simulink library "outp"  (R2021b)
settings: Solver=VariableStepAuto  StartTime=0.0  StopTime=10.0  RelTol=1e-3
undefined symbols (not defined in the file): ENUM_PMMMODE_CHARGE, ENUM_PMMMODE_IDLE, ENUM_PMMMODE_INITIALIZE, ENUM_PMMMODE_POWERDOWN, ENUM_PMMMODE_SLEEP, Left, outp, slcm, TRUE
libraries: FVT_lib x1177, hcu_lib x4, simulink x1
(part 2 of 11)

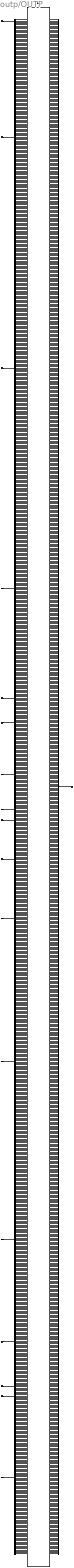
== system outp/OUTP ==
  BACC_outputs : Inport  OutDataTypeStr=Bus: BACC_outputs
  BAPM_outputs : Inport  Port=2  OutDataTypeStr=Bus: BAPM_outputs
  BBCM_outputs : Inport  Port=3  OutDataTypeStr=Bus: BBCM_outputs
  BDDM_outputs : Inport  Port=4  OutDataTypeStr=Bus: BDDM_outputs
  BDHP_outputs : Inport  Port=5  OutDataTypeStr=Bus: BDHP_outputs
  BDID_outputs : Inport  Port=6  OutDataTypeStr=Bus: BDID_outputs
  BDKC_outputs : Inport  Port=7  OutDataTypeStr=Bus: BDKC_outputs
  BDSC_outputs : Inport  Port=8  OutDataTypeStr=Bus: BDSC_outputs
  BNMM_outputs : Inport  Port=9  OutDataTypeStr=Bus: BNMM_outputs
  BPMM_outputs : Inport  Port=10  OutDataTypeStr=Bus: BPMM_outputs
  BSYS_outputs : Inport  Port=11  OutDataTypeStr=Bus: BSYS_outputs
  BTHC_outputs : Inport  Port=12  OutDataTypeStr=Bus: BTHC_outputs
  BTPM_outputs : Inport  Port=13  OutDataTypeStr=Bus: BTPM_outputs
  BTQD_outputs : Inport  Port=14  OutDataTypeStr=Bus: BTQD_outputs
  BTQR_outputs : Inport  Port=15  OutDataTypeStr=Bus: BTQR_outputs
  BV2L_outputs : Inport  Port=16  OutDataTypeStr=Bus: BV2L_outputs
  BVMC_outputs : Inport  Port=17  OutDataTypeStr=Bus: BVMC_outputs
  trig_OUTP : TriggerPort  TriggerType=function-call  VariantControl=(inherit)
  bus_creator : BusCreator  Inputs=1177  OutDataTypeStr=Bus: BOUTP_outputs  NonVirtualBus=on
  bus_selector1 : BusSelector  OutputSignals=VACC_HVTHCMSysAvail_enum,VACC_LVBattVoltSta_enum,VACC_VehHVPwrAvail4THCM_W
  bus_selector10 : BusSelector  OutputSignals=VPMM_PowerUpState_enum,VPMM_PowerDownState_enum,VPMM_PowerUpFault_enum,VPMM_PowerDownFault_enum,VPMM_ActiveDischargeReq_flg,VPMM_DCDCEnaReq_flg,VPMM_DCDCVoltSetpoint_V,VPMM_HVBatCnctReq_flg,VPMM_HVSysReadyToCharge_enum,VPMM_PowerSta_enum,VPMM_LVPwrSta_flg,VPMM_HVPwrSta_flg,VPMM_SysPowerMode_enum,VPMM_FrMCUEnaReq_flg,VPMM_RrMCUEnaReq_flg,VPMM_DrivetrainSelect_enum,VPMM_DrSeatSta_enum,VPMM_PwrStaSelect_enum,VPMM_PwrStaConstraint_enum,VPMM_TCountSta_enum,VPMM_PwrUpReq_enum,VPMM_PwrDownReq_enum,VPMM_LowSOCWarn_enum,VPMM_ReVehThdChkSta_enum,VPMM_EvccAplusPwrUpReq_flg,VPMM_PwrStaONTOPopReq_flg,VPMM_IVIPwrStaONTOPopT_s,VPMM_LVChrgHoldTtimer_s,VPMM_LVBattChrgTimeCnt_s,VPMM_SilentChkAllowSleep_flg,VPMM_TimerAllowSleep_flg,VPMM_FDADC12VDetAvg_mV,VPMM_PMMAllowECUSleep_flg,VPMM_LVSilentChrgSta_enum,VPMM_LVSilentChrgReq_flg,VPMM_LVSilentChrgLv_enum,VPMM_CtrlFrPwrStbA1P_flg,VPMM_CtrlFrRC1_flg,VPMM_CtrlFrBMSCCUCIR_flg,VPMM_CtrlFrEDUINVERTER_flg,VPMM_HWResetSta_enum,VPMM_CtrlDrPwrStbA2_flg,VPMM_PwrStaTOSta_enum,VPMM_Sched_ChgTOSta_enum,VPMM_PwrReq_OTA_enum,VPMM_OTAPwrReqOFFChkSta_enum,VPMM_OTAPwrReqStdChkSta_enum,VPMM_PwrReqRAPSAvail_flg
  bus_selector11 : BusSelector  OutputSignals=VSYS_HWVer1_cnt,VSYS_HWVer2_cnt,VSYS_HWVer3_cnt,VSYS_CarModel1_cnt,VSYS_CarModel2_cnt,VSYS_CarModel3_cnt,VSYS_ECU1_cnt,VSYS_ECU2_cnt,VSYS_Major1_cnt,VSYS_Major2_cnt,VSYS_Minor1_cnt,VSYS_Minor2_cnt,VSYS_Patch1_cnt,VSYS_Patch2_cnt,VSYS_Country1_cnt,VSYS_Country2_cnt,VSYS_Variation_cnt,VSYS_Dash1_cnt,VSYS_Change1_cnt,VSYS_Change2_cnt,VSYS_Dash2_cnt,VSYS_SHA1_cnt,VSYS_SHA2_cnt,VSYS_SHA3_cnt,VSYS_SHA4_cnt,VSYS_SHA5_cnt,VSYS_SHA6_cnt,VSYS_SHA7_cnt,VSYS_SHA8_cnt,VSYS_NvWriteReqRisingEdge_flg,VSYS_FdcSlpReqRisingEdge_flg,VSYS_FdcSlpTime_sec,VSYS_PmicBootReason_enum,VSYS_WisrBootReason_raw32,VSYS_AcoreRebootCmdACK_flg,VSYS_CurrentNmState_enum,VSYS_ECUGen1_cnt,VSYS_ECUGen2_cnt,VSYS_PmicBootPath_raw32,VSYS_DrivingMode_cnt,VSYS_ModelYear_cnt,VSYS_Var4_cnt,VSYS_Var5_cnt
  bus_selector12 : BusSelector  OutputSignals=VTHC_FDCompCmd_rpm,VTHC_FDSOV1Cmd_flg,VTHC_FDSOV2Cmd_flg,VTHC_FDSOV3Cmd_flg,VTHC_FDEXV1Cmd_step,VTHC_FDEXV2Cmd_step,VTHC_FDSOTXVCmd_flg,VTHC_FDFWVCmd_flg,VTHC_FDTWVCmd_pct,VTHC_FDFrWPTCHeatPwrCmd_W,VTHC_CoolgFanActDuty_pct,VTHC_FDAGSCmd_enum,VTHC_FDEWP1Cmd_enum,VTHC_FDEWP2Cmd_enum,VTHC_FDEWP3Cmd_enum,VTHC_FDFrLeAPTCHeatPwrCmd_W,VTHC_FDFrRiAPTCHeatPwrCmd_W,VTHC_FDRrAPTCHeatPwrCmd_W,VTHC_FDBlowerCmd_pct,VTHC_BatteryMode_enum,VTHC_EDriveMode_enum,VTHC_CabinMode_enum,VTHC_CCUACLampSts_flg,VTHC_CCUAutoLampSts_flg,VTHC_CCUACMaxLampSts_flg,VTHC_CCUSyncLampSts_flg,VTHC_sigAirIntenZon1St_enum,VTHC_sigWindDirZon1St_enum,VTHC_sigRecircSt_flg,VTHC_sigSetTempZon1St_C,VTHC_sigSetTempZon2St_C,VTHC_sigClntTHvBattOut_C,VTHC_sigCbnSolarLeft_W,VTHC_sigClntTHvBattIn_C,VTHC_sigCbnSolarRight_W,VTHC_sigAmbAirT_C,VTHC_sigCbnAirT_C,VTHC_ACSubMode_enum,VTHC_FDRecyAutoCmd_enum,VTHC_ACModeMem_enum,VTHC_Face_flg,VTHC_Foot_flg,VTHC_Frost_flg,VTHC_FaceM_flg,VTHC_FootM_flg,VTHC_CCUSyncSts_flg,VTHC_ACForceOFF_flg,VTHC_RecAutoFlg_flg,VTHC_AirIntenZone1M_enum,VTHC_fdefog_flg,VTHC_sigSetTempZon2StM_C,VTHC_sigDfrstSt_flg,VTHC_FDCTHCAirIntZ3Sta_enum,VTHC_FDCTHCLEVentModeSta_enum,VTHC_FDCTHCREVentModeSta_enum,VTHC_FDCTHCLEVentZSta_enum,VTHC_FDCTHCCLEVentZSta_enum,VTHC_FDCTHCREVentZSta_enum,VTHC_FDCTHCCREVentZSta_enum,VTHC_FDCTHCLEVentYSta_enum,VTHC_FDCTHCLVentENSta_flg,VTHC_FDCTHCCLEVentYSta_enum,VTHC_FDCTHCCLVentENSta_flg,VTHC_FDCTHCREVentYSta_enum,VTHC_FDCTHCRVentENSta_flg,VTHC_FDCTHCCREVentYSta_enum,VTHC_FDCTHCCRVentENSta_flg,VTHC_FDCTHCMAPTCForceOFFSta_flg,VTHC_FDCFGSAirIntSta_enum,VTHC_FDCFGSChSta_enum,VTHC_FDCFGSAirIntCmd_enum,VTHC_FDCFGSFuncSta_enum,VTHC_FDCFGSChCmd_enum,VTHC_FDCFGSIONSWSta_flg,VTHC_FDCFGSIONCmd_flg,VTHC_FDCTHCMPreWPTCHeatSta_enum,VTHC_EWPBUflag1_flg,VTHC_EWPBUflag2_flg,VTHC_EWPBUflag3_flg,VTHC_FaceMSet_enum,VTHC_FootMSet_enum,VTHC_fdefogSet_enum,VTHC_CCUSyncStsSet_enum,VTHC_sigRecircStSet_enum,VTHC_RecyAutoSet_enum,VTHC_AirIntenZone1MSet1_enum,VTHC_AirIntenZone1MSet2_enum,VTHC_AirIntenZone1MSet3_enum,VTHC_AirIntenZone1MSet4_enum,VTHC_AirIntenZone1MSet5_enum,VTHC_AirIntenZone1MSet7_enum,VTHC_AirIntenZone3MSet1_enum,VTHC_AirIntenZone3MSet2_enum,VTHC_AirIntenZone3MSet3_enum,VTHC_AirIntenZone3MSet4_enum,VTHC_AirIntenZone3MSet5_enum,VTHC_AirIntenZone3MSet7_enum,VTHC_IONSWStaSet_enum,VTHC_FDCFGSChStaSet123_enum,VTHC_FDCFGSChStaSet457_enum,VTHC_FDCFGSAirIntStaSet123_enum,VTHC_FDCFGSAirIntStaSet457_enum,VTHC_LVentENSet_enum,VTHC_CLVentENSet_enum,VTHC_RVentENSet_enum,VTHC_CRVentENSet_enum,VTHC_LEVentModeStaSet123_enum,VTHC_LEVentModeStaSet457_enum,VTHC_REVentModeStaSet123_enum,VTHC_REVentModeStaSet457_enum,VTHC_FDCTHCLEVentZStaSet1_enum,VTHC_FDCTHCLEVentZStaSet2_enum,VTHC_FDCTHCLEVentZStaSet3_enum,VTHC_FDCTHCLEVentZStaSet4_enum,VTHC_FDCTHCLEVentZStaSet5_enum,VTHC_FDCTHCLEVentZStaSet7_enum,VTHC_FDCTHCCLEVentZStaSet1_enum,VTHC_FDCTHCCLEVentZStaSet2_enum,VTHC_FDCTHCCLEVentZStaSet3_enum,VTHC_FDCTHCCLEVentZStaSet4_enum,VTHC_FDCTHCCLEVentZStaSet5_enum,VTHC_FDCTHCCLEVentZStaSet7_enum,VTHC_FDCTHCREVentZStaSet1_enum,VTHC_FDCTHCREVentZStaSet2_enum,VTHC_FDCTHCREVentZStaSet3_enum,VTHC_FDCTHCREVentZStaSet4_enum,VTHC_FDCTHCREVentZStaSet5_enum,VTHC_FDCTHCREVentZStaSet7_enum,VTHC_FDCTHCCREVentZStaSet1_enum,VTHC_FDCTHCCREVentZStaSet2_enum,VTHC_FDCTHCCREVentZStaSet3_enum,VTHC_FDCTHCCREVentZStaSet4_enum,VTHC_FDCTHCCREVentZStaSet5_enum,VTHC_FDCTHCCREVentZStaSet7_enum,VTHC_FDCTHCLEVentYStaSet1_enum,VTHC_FDCTHCLEVentYStaSet2_enum,VTHC_FDCTHCLEVentYStaSet3_enum,VTHC_FDCTHCLEVentYStaSet4_enum,VTHC_FDCTHCLEVentYStaSet5_enum,VTHC_FDCTHCLEVentYStaSet7_enum,VTHC_FDCTHCCLEVentYStaSet1_enum,VTHC_FDCTHCCLEVentYStaSet2_enum,VTHC_FDCTHCCLEVentYStaSet3_enum,VTHC_FDCTHCCLEVentYStaSet4_enum,VTHC_FDCTHCCLEVentYStaSet5_enum,VTHC_FDCTHCCLEVentYStaSet7_enum,VTHC_FDCTHCREVentYStaSet1_enum,VTHC_FDCTHCREVentYStaSet2_enum,VTHC_FDCTHCREVentYStaSet3_enum,VTHC_FDCTHCREVentYStaSet4_enum,VTHC_FDCTHCREVentYStaSet5_enum,VTHC_FDCTHCREVentYStaSet7_enum,VTHC_FDCTHCCREVentYStaSet1_enum,VTHC_FDCTHCCREVentYStaSet2_enum,VTHC_FDCTHCCREVentYStaSet3_enum,VTHC_FDCTHCCREVentYStaSet4_enum,VTHC_FDCTHCCREVentYStaSet5_enum,VTHC_FDCTHCCREVentYStaSet7_enum,VTHC_SettempZon1Set1_enum,VTHC_SettempZon1Set2_enum,VTHC_SettempZon1Set3_enum,VTHC_SettempZon1Set4_enum,VTHC_SettempZon1Set5_enum,VTHC_SettempZon1Set7_enum,VTHC_ACModeSet123_enum,VTHC_ACModeSet457_enum,VTHC_FACESet_enum,VTHC_FOOTSet_enum,VTHC_FrostSet_enum,VTHC_LVentEN_flg,VTHC_CLVentEN_flg,VTHC_RVentEN_flg,VTHC_CRVentEN_flg,VTHC_FDCFGSLearnCmd_enum,VTHC_FDCFGSFuncSta_flg,VTHC_THSysErrlampReq_flg
  bus_selector13 : BusSelector  OutputSignals=VTPM_LFBatWarn_flg,VTPM_RFBatWarn_flg,VTPM_LRBatWarn_flg,VTPM_RRBatWarn_flg,VTPM_LFWheelPress_raw8,VTPM_RFWheelPress_raw8,VTPM_LRWheelPress_raw8,VTPM_RRWheelPress_raw8,VTPM_LFWheelTemp_C,VTPM_RFWheelTemp_C,VTPM_LRWheelTemp_C,VTPM_RRWheelTemp_C,VTPM_LFSensorFail_flg,VTPM_RFSensorFail_flg,VTPM_LRSensorFail_flg,VTPM_RRSensorFail_flg,VTPM_LFWheelDebug_flg,VTPM_LRWheelDebug_flg,VTPM_RFWheelDebug_flg,VTPM_RRWheelDebug_flg,VTPM_TPMSResButtAllow_flg,VTPM_TPMSCaliButtAllow_flg,VTPM_LFPressIndi_enum,VTPM_RFPressIndi_enum,VTPM_LRPressIndi_enum,VTPM_RRPressIndi_enum,VTPM_TPMSWarnIndi_enum,VTPM_LFWheelTmpIndi_flg,VTPM_RFWheelTmpIndi_flg,VTPM_LRWheelTmpIndi_flg,VTPM_RRWheelTmpIndi_flg,VTPM_LFWheelPSW_raw8,VTPM_LRWheelPSW_raw8,VTPM_RFWheelPSW_raw8,VTPM_RRWheelPSW_raw8,VTPM_CWheelTips_enum,VTPM_AutoLTips_enum,VTPM_LFSensorMode_flg,VTPM_RFSensorMode_flg,VTPM_LRSensorMode_flg,VTPM_RRSensorMode_flg,VTPM_S1ID_raw32,VTPM_S2ID_raw32,VTPM_S3ID_raw32,VTPM_S4ID_raw32,VTPM_S1L_enum,VTPM_S2L_enum,VTPM_S3L_enum,VTPM_S4L_enum,VTPM_ALFin_flg,VTPM_LFP20_raw8,VTPM_RFP20_raw8,VTPM_LRP20_raw8,VTPM_RRP20_raw8,VTPM_FAT_flg,VTPM_IDin_raw32,VTPM_S1WheelDebugALTU_pct,VTPM_S2WheelDebugALTU_pct,VTPM_S3WheelDebugALTU_pct,VTPM_S4WheelDebugALTU_pct,VTPM_ID1messageALTU_raw8,VTPM_ID2messageALTU_raw8,VTPM_ID3messageALTU_raw8,VTPM_ID4messageALTU_raw8,VTPM_Chkfin_flg,VTPM_SetIDLoc_flg,VTPM_TPMSStorge_flg,VTPM_ChkStorge_flg,VTPM_TPMSResButt_flg,VTPM_LFPindi_enum,VTPM_RFPind_enum,VTPM_LRPindi_enum,VTPM_RRPindi_enum,VTPM_WriteChkLFID_raw,VTPM_WriteChkRFID_raw,VTPM_WriteChkLRID_raw,VTPM_WriteChkRRID_raw,VTPM_WriteChkfinLFID_raw,VTPM_WriteChkfinRFID_raw,VTPM_WriteChkfinLRID_raw,VTPM_WriteChkfinRRID_raw,VTPM_Flashchkdatavalid_enum,VTPM_Flashdatavalid_enum,VTPM_unlearnSfali_flg,VTPM_unlearnSfailvalid_enum,VTPM_Prepresstempvalid_enum,VTPM_FlashS1ID_raw,VTPM_FlashS2ID_raw,VTPM_FlashS3ID_raw,VTPM_FlashS4ID_raw,VTPM_FlashIDvalid_enum,VTPM_WritingCnt_enum,VTPM_TPMSTLCmd_flg,VTPM_LProgress_enum,VTPM_TPMSSensorIDRegStart_flg,VTPM_ModelVersion_raw,VTPM_ModelVersionChksum_raw
  bus_selector14 : BusSelector  OutputSignals=VTQD_ParkRequest_flg,VTQD_TqSourceFr_enum,VTQD_TqSourceRr_enum,VTQD_FrEDUAvailBrkRgnTq_Nm,VTQD_RrEDUAvailBrkRgnTq_Nm,VTQD_EVDriveMode_enum,VTQD_ShiftGearPosn_enum,VTQD_PButtonSta_enum,VTQD_FrActvDmpDisabReq_flg,VTQD_RrActvDmpDisabReq_flg,VTQD_FrRgnDecrSta_flg,VTQD_RrRgnDecrSta_flg,VTQD_DriverWhlTqDemFr_Nm,VTQD_DriverWhlTqDemRr_Nm,VTQD_FrEDUActTq_Nm,VTQD_RrEDUActTq_Nm,VTQD_FrEDURolRgnTq_Nm,VTQD_RrEDURolRgnTq_Nm,VTQD_FrEDUSpd_rpm,VTQD_RrEDUSpd_rpm,VTQD_FrEDUSpdValid_flg,VTQD_FrEDUAvailBrkRgnTqV_flg,VTQD_RrEDUSpdValid_flg,VTQD_RrEDUAvailBrkRgnTqV_flg,VTQD_RgnAbnorSta_flg,VTQD_PTCSPermSta_flg,VTQD_FrRgnPermSta_flg,VTQD_RrRgnPermSta_flg,VTQD_FrIdcMin_A,VTQD_FrIdcMax_A,VTQD_FrUdcMin_V,VTQD_FrUdcMax_V,VTQD_RrIdcMin_A,VTQD_RrIdcMax_A,VTQD_RrUdcMin_V,VTQD_RrUdcMax_V,VTQD_ReBrakeLPReq_flg,VTQD_BOSEnable_flg,VTQD_CreepON_flg,VTQD_RDCActive_enum,VTQD_EquivAccPedalSWSta_flg,VTQD_DriveProtEn_flg,VTQD_ActParkRequest_flg,VTQD_RegenTqLimitEn_flg,VTQD_IVIPwrLockSta_enum,VTQD_OPDHoldLamp_flg,VTQD_SaveRegenMode_enum,VTQD_FDCVCURegenMode_enum,VTQD_SpdCtrlMode_enum,VTQD_SpdCtrlSta_flg,VTQD_SetSpd_kph,VTQD_VehActSpd_kph,VTQD_RegenLimIndSta_flg,VTQD_SetSpdLimWarn_flg,VTQD_MaxWhlSlideRate_pct,VTQD_TrailerDisOPDSta_flg,VTQD_ForceP_flg,VTQD_SlideRegenLimTq_Nm,VTQD_SimSoundCmd_pct,VTQD_SimSouWaveReq_pct
  bus_selector15 : BusSelector  OutputSignals=VTQR_FrTMTqReq_Nm,VTQR_RrTMTqReq_Nm,VTQR_FrFirstOrderInpTs_c,VTQR_RrFirstOrderInpTs_c,VTQR_FrRateLimitInc_Nm,VTQR_FrRateLimitDec_Nm,VTQR_RrRateLimitInc_Nm,VTQR_RrRateLimitDec_Nm
  bus_selector16 : BusSelector  OutputSignals=VV2L_ReqOBCV2LEna_enum,VV2L_ReqV2LIVIPopup_enum,VV2L_ReqV2LIVIDisChrg_enum,VV2L_ReqOBCExtrV2LEna_enum,VV2L_ReqOBCIntrV2LEna_enum,VV2L_HVPO120VGrpALDSt_enum,VV2L_HVPO120VGrpBLDSt_enum
  bus_selector17 : BusSelector  OutputSignals=VVMC_FeatSetSpdFinal_raw32,VVMC_VehicleSpeed_mph,VVMC_VehicleSpeed_kph,VVMC_MeterIndSpeed_raw32,VVMC_VMCAEBCtrlAvail_flg,VVMC_VMCACCCtrlAvail_flg,VVMC_VMCCCCtrlAvail_flg,VVMC_VMCMSACtrlAvail_flg,VVMC_FeatArbitrSta_enum,VVMC_FeatReqSpd_kph,VVMC_JerkPCT_pct,VVMC_LimitPCT_pct,VVMC_FrontRearSlipRatioCtrl_flg,VVMC_RearWhlSlipRatioCtrl_flg,VVMC_SingleWhlSlipRatioCtrl_flg,VVMC_LatAccCtrl_flg,VVMC_SafetyCtrl_flg,VVMC_SPD2ACCAct_flg,VVMC_AccCalcuPID_mps2,VVMC_ISOAccLimit_mps2,VVMC_ISODecLimit_mps2,VVMC_ISOJerkLimit_mps3,VVMC_ACCRequiredAccel_mps2,VVMC_DISCReqAcc_mps2,VVMC_FeatArbitrFinal_enum,VVMC_ActACCRequiredAccel_mps2,VVMC_LateralCtrl_flg,VVMC_ADASLKASta_enum,VVMC_LKAStrToqReq_Nm,VVMC_LKATOIFault_flg,VVMC_LKATOIAct_enum,VVMC_ADASAEBReq_enum,VVMC_ADASFaultSta_flg,VVMC_AEBVehHoldReq_flg,VVMC_ACCVehHoldReq_flg,VVMC_ADASDBSReq_enum,VVMC_ADASACCSta_enum,VVMC_ACCObjDist_m,VVMC_ACCObjRelSpd_mps,VVMC_TimeGapLevel_enum,VVMC_ACCJerkUpperLimit_mps3,VVMC_ACCComfortBandUpper_mps2,VVMC_ACCJerkLowerLimit_mps3,VVMC_ACCComfortBandLower_mps2,VVMC_ADASVehSpdLim_raw32,VVMC_ADASShftPosnReqA_flg,VVMC_ADASShftPosnReq_enum,VVMC_ADASForceIdle_flg,VVMC_HazardWarningReq_flg,VVMC_RightTurnLightReq_flg,VVMC_LeftTurnLightReq_flg,VVMC_ADASFCWSta_enum,VVMC_ADASLDWSta_enum,VVMC_ADASFltWrnReq_flg,VVMC_ACCObjDstLvl_enum,VVMC_ForceLowBeam_enum,VVMC_ACCTakeoverReq_flg,VVMC_ADASWarningMsg_enum,VVMC_ADASCAMSpdLim_enum,VVMC_TargetType_enum,VVMC_ADASSLIFSpdLim_enum,VVMC_LKAHODDisplayWarning_flg,VVMC_LKAHODSoundWarning_flg,VVMC_ADASLFCSta_enum,VVMC_ADASLaneModeL_enum,VVMC_ADASLaneModeR_enum,VVMC_ADASSLIFSta_enum,VVMC_ADASISASta_enum,VVMC_ADASLDWMute_flg,VVMC_ADASFCWMute_flg,VVMC_ADASLFCHandsOffWarning_enum,VVMC_LVDADisabled_flg,VVMC_LVDAMuteSta_enum,VVMC_LVDAFailinfo_flg,VVMC_LVDAWarning_flg,VVMC_LVDAACCStatusInformation_flg,VVMC_ADASLFCWarnSound_enum,VVMC_FCMACCmode_enum,VVMC_ADASLanetypeR_enum,VVMC_ADASLanetypeL_enum,VVMC_ADASLanecurveL_raw32,VVMC_ADASLanecurveR_raw32,VVMC_ADASAEBSta_enum,VVMC_FCMLDWRequest_enum,VVMC_FCMLDWFault_flg,VVMC_ACCCtrlAvail_flg,VVMC_ACCPedalOvrd_flg,VVMC_TimeGapCalcu_s,VVMC_CCCtrlSta_enum,VVMC_MSACtrlSta_enum,VVMC_APSCtrlAvail_flg,VVMC_APSActive_flg,VVMC_APSStaSys_enum,VVMC_APSDecReqA_flg,VVMC_APSDecReq_mps2,VVMC_APSReq_enum,VVMC_LongAcc_Gps,VVMC_CCMSASpdWar_flg,VVMC_IMUEnaCmd_flg,VVMC_ActStESCYaw_Dps,VVMC_CAASCtrlAvail_flg,VVMC_CAASActive_flg,VVMC_ExtraMSACtrlSta_enum,VVMC_CalibratedAccX_G,VVMC_CalibratedAccY_G,VVMC_CalibratedAccZ_G,VVMC_CalibratedGyroX_Dps,VVMC_CalibratedGyroY_Dps,VVMC_CalibratedGyroZ_Dps,VVMC_FDCVMCAPSVRqEPSCtrl_flg,VVMC_FDCVMCAPSAngleTarget_deg,VVMC_FDCVMCAPSRqEPSCtrl_flg,VVMC_FDCVMCAngCtrlTqWtGn_pct,VVMC_FDCVMCDrInpTqBstAct_flg,VVMC_FDCVMCMaxAngCtrlOutTqLim_Nm,VVMC_FDCVMCDrInpTqBstGn_pct,VVMC_VehPitchAngleSta_enum,VVMC_DMSModeCmd_enum
  bus_selector2 : BusSelector  OutputSignals=VAPM_VehSpeed_kph,VAPM_VehSpeedTimeOut_flg,VAPM_FSOffSw_enum,VAPM_FSOffSwTimeOut_flg,VAPM_ChrgPlugSta_enum,VAPM_PASDRMR_cm,VAPM_PASDRML_cm,VAPM_PASDRCR_cm,VAPM_PASDRCL_cm,VAPM_PASDFMR_cm,VAPM_PASDFML_cm,VAPM_PASDFCR_cm,VAPM_PASDFCL_cm,VAPM_APSDRLR_cm,VAPM_APSDRLL_cm,VAPM_APSDFLR_cm,VAPM_APSDFLL_cm,VAPM_PASAFCL_enum,VAPM_PASARMR_enum,VAPM_PASARML_enum,VAPM_PASARCR_enum,VAPM_PASARCL_enum,VAPM_PASAFMR_enum,VAPM_PASAFML_enum,VAPM_PASAFCR_enum,VAPM_USSStaRMR_flg,VAPM_USSStaRML_flg,VAPM_USSStaRLR_flg,VAPM_USSStaRLL_flg,VAPM_USSStaRCR_flg,VAPM_USSStaRCL_flg,VAPM_USSStaFMR_flg,VAPM_USSStaFML_flg,VAPM_USSStaFLR_flg,VAPM_USSStaFLL_flg,VAPM_USSStaFCR_flg,VAPM_USSStaFCL_flg,VAPM_Chime_enum,VAPM_SNSRLayout_enum,VAPM_StaFSya_flg,VAPM_ModOperation_enum,VAPM_BrkPedalPos_pct,VAPM_BrkPedalPosTimeOut_flg,VAPM_LFRawWhlSpeed_kph,VAPM_LFRawWhlSpeedTimeOut_flg,VAPM_RFRawWhlSpeed_kph,VAPM_RFRawWhlSpeedTimeOut_flg,VAPM_LRRawWhlSpeed_kph,VAPM_LRRawWhlSpeedTimeOut_flg,VAPM_RRRawWhlSpeed_kph,VAPM_RRRawWhlSpeedTimeOut_flg,VAPM_LFRawWhlSpeedV_flg,VAPM_LFRawWhlSpeedVTimeOut_flg,VAPM_RFRawWhlSpeedV_flg,VAPM_RFRawWhlSpeedVTimeOut_flg,VAPM_LRRawWhlSpeedV_flg,VAPM_LRRawWhlSpeedVTimeOut_flg,VAPM_RRRawWhlSpeedV_flg,VAPM_RRRawWhlSpeedVTimeOut_flg,VAPM_LFWhlRotDir_enum,VAPM_LFWhlRotDirTimeOut_flg,VAPM_RFWhlRotDir_enum,VAPM_RFWhlRotDirTimeOut_flg,VAPM_LRWhlRotDir_enum,VAPM_LRWhlRotDirTimeOut_flg,VAPM_RRWhlRotDir_enum,VAPM_RRWhlRotDirTimeOut_flg,VAPM_LFPulseCountV_flg,VAPM_LFPulseCountVTimeOut_flg,VAPM_RFPulseCountV_flg,VAPM_RFPulseCountVTimeOut_flg,VAPM_LRPulseCountV_flg,VAPM_LRPulseCountVTimeOut_flg,VAPM_RRPulseCountV_flg,VAPM_RRPulseCountVTimeOut_flg,VAPM_LFPulseCount_enum,VAPM_LFPulseCountTimeOut_flg,VAPM_RFPulseCount_enum,VAPM_RFPulseCountTimeOut_flg,VAPM_LRPulseCount_enum,VAPM_LRPulseCountTimeOut_flg,VAPM_RRPulseCount_enum,VAPM_RRPulseCountTimeOut_flg,VAPM_ShifterHandleCmd_enum,VAPM_ShifterHandleCmdTimeOut_flg,VAPM_DriIntend_enum,VAPM_DriIntendTimeOut_flg,VAPM_EPSAOIControl_enum,VAPM_EPSAOIControlTimeOut_flg,VAPM_SASAngle_Deg,VAPM_SASAngleTimeOut_flg,VAPM_SASSpeed_degps,VAPM_SASSpeedTimeOut_flg,VAPM_SASSpeedValid_flg,VAPM_SASSpeedValidTimeOut_flg,VAPM_SASCAL_flg,VAPM_SASCALTimeOut_flg,VAPM_SASV_flg,VAPM_SASVTimeOut_flg,VAPM_GRADE_Deg,VAPM_GRADETimeOut_flg,VAPM_YawRate_degps,VAPM_YawRateTimeOut_flg,VAPM_LatAccel_Gps,VAPM_LatAccelTimeOut_flg,VAPM_LongAccel_Gps,VAPM_LongAccelTimeOut_flg,VAPM_MCPressure_bar,VAPM_MCPressureTimeOut_flg,VAPM_YawRateV_flg,VAPM_YawRateVTimeOut_flg,VAPM_LatAccelV_flg,VAPM_LatAccelVTimeOut_flg,VAPM_LongAccelV_flg,VAPM_LongAccelVTimeOut_flg,VAPM_MCPressureV_bar,VAPM_MCPressureVTimeOut_flg,VAPM_BrkSwSta_flg,VAPM_BrkSwStaTimeOut_flg,VAPM_BrkSwV_flg,VAPM_BrkSwVTimeOut_flg,VAPM_ESCStandstill_flg,VAPM_ESCStandstillTimeOut_flg,VAPM_ESCAPSSta_enum,VAPM_ESCAPSStaTimeOut_flg,VAPM_EPBExtReleaseAvail_flg,VAPM_EPBExtReleaseAvailTimeOut_flg,VAPM_EPBExtApplyAvail_flg,VAPM_EPBExtApplyAvailTimeOut_flg,VAPM_EPBErrSta_enum,VAPM_EPBErrStaTimeOut_flg,VAPM_EPBSta_enum,VAPM_EPBStaTimeOut_flg,VAPM_AVMparkingcancel_enum,VAPM_AVMparkingcancelTimeOut_flg,VAPM_AVMparkingexcute_enum,VAPM_AVMparkingexcuteTimeOut_flg,VAPM_AVMParkingmode_enum,VAPM_AVMParkingmodeTimeOut_flg,VAPM_AVMErrSTA_flg,VAPM_AVMErrSTATimeOut_flg,VAPM_IVIStatus_flg,VAPM_IVIStatusTimeOut_flg,VAPM_CAASSw_enum,VAPM_CAASSwTimeOut_flg,VAPM_IVIScreen_enum,VAPM_IVIScreenTimeOut_flg,VAPM_ABSActive_flg,VAPM_ABSActiveTimeOut_flg,VAPM_TCSActive_flg,VAPM_TCSActiveTimeOut_flg,VAPM_DriverSeatBeltCmd_flg,VAPM_DriverSeatBeltCmdTimeOut_flg,VAPM_APSProgressPCT_pct,VAPM_APSRQDisplay_enum,VAPM_APSSWVer_enum,VAPM_APSHWVer_enum,VAPM_APSExitCondition_enum,VAPM_APSAngleTarget_Deg,VAPM_APSVRqEPASCtrl_flg,VAPM_APSRqEPASCtrl_flg,VAPM_CAASSta_enum,VAPM_DKCPDkeyAreaRAPSSta_enum,VAPM_DKCParkingModeCmd_enum,VAPM_PUIDLowPower_flg,VAPM_CAASVMCReqA_flg,VAPM_APSShiftPosnReq_enum,VAPM_APSSpeedCMD_kph,VAPM_APSVMCReqA_flg,VAPM_RAPSBCMLamp_enum,VAPM_RAPSBCMLockReq_flg,VAPM_APSPwrReq_enum,VAPM_RAPSErrWarnSta_enum,VAPM_RAPSErrLv1_flg,VAPM_IVIUserTakeOverAPSSta_flg
  bus_selector3 : BusSelector  OutputSignals=VBCM_AntitheftSta_enum,VBCM_TailgateRemote_enum,VBCM_HornCtrl_flg,VBCM_AllDoorSW_flg,VBCM_BCMDoorLockSta_flg,VBCM_AntitheftSeatFlod_flg,VBCM_HoodSW_flg,VBCM_TailgateSW_flg,VBCM_DrDoorSW_flg,VBCM_PsDoorSW_flg,VBCM_RLDoorSW_flg,VBCM_RRDoorSW_flg,VBCM_LockSetting_flg,VBCM_FrChargingDoorCtrl_enum,VBCM_RrChargingDoorCtrl_enum,VBCM_CrashDetd_flg,VBCM_CTDCtrl_enum,VBCM_DoorLockIND_flg,VBCM_CTDLockSW_flg,VBCM_Dimmer_pct,VBCM_DimmerEN_flg,VBCM_PosLamp_flg,VBCM_LBeam_flg,VBCM_HBeam_flg,VBCM_RrFogLamp_flg,VBCM_BrakeLamp_flg,VBCM_ReverseLamp_flg,VBCM_LDRL_flg,VBCM_RDRL_flg,VBCM_LBSD_flg,VBCM_RBSD_flg,VBCM_HazardSW_flg,VBCM_LTurnLP_flg,VBCM_RTurnLP_flg,VBCM_BCMBuzzerReq_flg,VBCM_MirrorCtrl_enum,VBCM_MirrorDefog_flg,VBCM_RrDefog_flg,VBCM_RoomLampH_flg,VBCM_RoomLampL_flg,VBCM_TrunkRel_flg,VBCM_TailgateHDSW_flg,VBCM_FrWiperL_flg,VBCM_FrWiperH_flg,VBCM_RrWiper_flg,VBCM_WasherCtrl_enum,VBCM_WiperFixMode_flg,VBCM_AmbLightBreath1_enum,VBCM_AmbLightBreath2_enum,VBCM_AmbLightBreath3_enum,VBCM_AmbLightBreath4_enum,VBCM_AmbLightBreath5_enum,VBCM_AmbLightBreath6_enum,VBCM_AmbLightBrightness1_enum,VBCM_AmbLightBrightness2_enum,VBCM_AmbLightBrightness3_enum,VBCM_AmbLightBrightness4_enum,VBCM_AmbLightBrightness5_enum,VBCM_AmbLightBrightness6_enum,VBCM_AmbLightColor1_enum,VBCM_AmbLightColor2_enum,VBCM_AmbLightColor3_enum,VBCM_AmbLightColor4_enum,VBCM_AmbLightColor5_enum,VBCM_AmbLightColor6_enum,VBCM_LampPwr_flg,VBCM_SPTGDet_flg,VBCM_APSOpenPTG_flg,VBCM_FollowMe_flg,VBCM_IVIRST_flg,VBCM_CountAlarm_enum,VBCM_MFSWTri_flg,VBCM_MirrorFlodPos_flg,VBCM_FuelDoorPos_flg,VBCM_MFRDNBrightReq_pct,VBCM_PTGInnerSW2_enum,VBCM_DrvWdwCtrlCmd_pct,VBCM_PasWdwCtrlCmd_pct,VBCM_DrRWdwCtrlCmd_pct,VBCM_PsRWdwCtrlCmd_pct,VBCM_APMDoorControlSta_flg,VBCM_AmbFunEN_flg,VBCM_AmbWelEN_flg,VBCM_AmbDimEN_flg,VBCM_AmbLinkDriSta_flg,VBCM_AmbPwrWarnEN_flg,VBCM_AmbODAEN_flg,VBCM_AmbColorSta_enum,VBCM_AmbBrightSta_enum,VBCM_LockAlarm_enum,VBCM_ATCtrl_enum,VBCM_fUnlockSingle_flg,VBCM_UserNow_enum,VBCM_AmbFunENFlash_enum,VBCM_AmbWelENFlash_enum,VBCM_AmbDimENFlash_enum,VBCM_AmbLinkDriStaFlash_enum,VBCM_AmbPwrWarnENFlash_enum,VBCM_AmbODAENFlash_enum,VBCM_AmbColorSta1_enum,VBCM_AmbColorSta2_enum,VBCM_AmbColorSta3_enum,VBCM_AmbColorSta4_enum,VBCM_AmbColorSta5_enum,VBCM_AmbColorSta7_enum,VBCM_AmbBrightnessSta1_enum,VBCM_AmbBrightnessSta2_enum,VBCM_AmbBrightnessSta3_enum,VBCM_AmbBrightnessSta4_enum,VBCM_AmbBrightnessSta5_enum,VBCM_AmbBrightnessSta7_enum,VBCM_HazardIND_flg,VBCM_DimSwSta_flg,VBCM_PassSWSta_flg,VBCM_FWipSwSta_enum,VBCM_FWasSwSta_enum,VBCM_TurnSwSta_enum,VBCM_TurnSwTSetSta_enum,VBCM_SPTGENFun_flg,VBCM_SPTGENFunMem_enum,VBCM_OutMode_enum,VBCM_TurnSwTimeSetSta123_enum,VBCM_TurnSwTimeSetSta457_enum,VBCM_FDLHandleLampCmd_flg,VBCM_FDRHandleLampCmd_flg,VBCM_FDHandleCmd_enum,VBCM_HBeamADB_enum,VBCM_WalkInUnLkENMem_enum,VBCM_WalkOutLkENMem_enum,VBCM_RmLpModeENMem_enum,VBCM_LockSettingStaMem_enum,VBCM_FollowMeENMem_enum,VBCM_WalkInUnLkENFunSta_flg,VBCM_WalkOutLkENFunSta_flg,VBCM_RmLpModeENFunSta_flg,VBCM_FollowMeENFunSta_flg,VBCM_HoodRelCmd_flg,VBCM_WelcomeLight_enum,VBCM_PTGOpenHeightSta_enum,VBCM_UserHeightSet_cnt,VBCM_PTGUserHeight1_cnt,VBCM_PTGUserHeight2_cnt,VBCM_PTGUserHeight3_cnt,VBCM_PTGUserHeight4_cnt,VBCM_PTGUserHeight5_cnt,VBCM_PTGUserHeight7_cnt,VBCM_PTGOpenHeight12_enum,VBCM_PTGOpenHeight34_enum,VBCM_PTGOpenHeight57_enum,VBCM_SenstivityPosnCmd_enum,VBCM_TimeGapLevelSta_enum,VBCM_ACCLevelMem12_enum,VBCM_ACCLevelMem34_enum,VBCM_ACCLevelMem57_enum,VBCM_LRightStaCmd_flg,VBCM_LLeftStaCmd_flg,VBCM_AutoLockSta_flg,VBCM_AutoLockMem_enum,VBCM_AutoUnlockSta_flg,VBCM_AutoUnlockMem_enum,VBCM_HMIKey1FuncSta_enum,VBCM_HMIKey2FuncSta_enum,VBCM_HMIKey3FuncSta_enum,VBCM_HMIKey4FuncSta_enum,VBCM_HMIKey5FuncSta_enum,VBCM_HMIKey6FuncSta_enum,VBCM_HMIKey7FuncSta_enum,VBCM_HMIKey8FuncSta_enum,VBCM_AutoWipHSpdENSta_flg,VBCM_DrvWdwReqAP_enum,VBCM_PasWdwReqAP_enum,VBCM_DrRWdwReqAP_enum,VBCM_PsRWdwReqAP_enum,VBCM_CLWinLockDrSta_flg,VBCM_CLWinLockDrStaMem_enum,VBCM_WinLFOpenedSta_pct,VBCM_WinRFOpenedSta_pct,VBCM_WinLROpenedSta_pct,VBCM_WinRROpenedSta_pct
  bus_selector4 : BusSelector  OutputSignals=VDDM_C3BMS6RCDTC_raw32,VDDM_C3BMS6CSDTC_raw32,VDDM_C3BMS6LCDTC_raw32,VDDM_C3BMS1RCDTC_raw32,VDDM_C3BMS1CSDTC_raw32,VDDM_C3BMS1LCDTC_raw32,VDDM_C3CCU1RCDTC_raw32,VDDM_C3CCU1CSDTC_raw32,VDDM_C3CCU1LCDTC_raw32,VDDM_C3CCU2RCDTC_raw32,VDDM_C3CCU2CSDTC_raw32,VDDM_C3CCU2LCDTC_raw32,VDDM_C1ABM1RCDTC_raw32,VDDM_C1ABM1CSDTC_raw32,VDDM_C1ABM1LCDTC_raw32,VDDM_Lv1ErrDTC_raw32,VDDM_Lv2ErrDTC_raw32,VDDM_Lv3ErrDTC_raw32,VDDM_Lv4ErrDTC_raw32,VDDM_BrkSWErrDTC_raw32,VDDM_BrkSWNoBacDTC_raw32,VDDM_KeyAuthDTC_raw32,VDDM_ONtoRdyDTC_raw32,VDDM_HVB4PreDTC_raw32,VDDM_MCU4PreDTC_raw32,VDDM_DCDC4PreDTC_raw32,VDDM_HVRlyCloDTC_raw32,VDDM_BMSRdyDTC_raw32,VDDM_DCDCEnaDTC_raw32,VDDM_HiLvSaChkDTC_raw32,VDDM_MidLvSaChkDTC_raw32,VDDM_MCUDisDTC_raw32,VDDM_DCDCDisDTC_raw32,VDDM_HVRlyOpDTC_raw32,VDDM_MCUActDTC_raw32,VDDM_OBC4PreDTC_raw32,VDDM_IniLVLoDTC_raw32,VDDM_LVSupLoDTC_raw32,VDDM_LVSupHiDTC_raw32,VDDM_DrStSWDTC_raw32,VDDM_FLDoorSWDTC_raw32,VDDM_RLDoorSWDTC_raw32,VDDM_FRDoorSWDTC_raw32,VDDM_RRDoorSWDTC_raw32,VDDM_HoodSWDTC_raw32,VDDM_TailgaSWDTC_raw32,VDDM_EDriveSysErrVCUErr_flg,VDDM_VehMalfunLevel_enum,VDDM_APS1SigOoRDTC_raw32,VDDM_APS2SigOoRDTC_raw32,VDDM_APSCorrErrDTC_raw32,VDDM_MCUF1NoComDTC_raw32,VDDM_MCUR1NoComDTC_raw32,VDDM_Shifter1NoComDTC_raw32,VDDM_ESC7NoComDTC_raw32,VDDM_ESC1NoComDTC_raw32,VDDM_ESC5NoComDTC_raw32,VDDM_EnterNewOperCyc_flg,VDDM_DiagHCrashDTC_raw32,VDDM_DiagFLTSDTC_raw32,VDDM_DiagFRTSDTC_raw32,VDDM_DiagRLTSDTC_raw32,VDDM_DiagRRTSDTC_raw32,VDDM_FCLUSSDTC_raw32,VDDM_FMLUSSDTC_raw32,VDDM_FMRUSSDTC_raw32,VDDM_FCRUSSDTC_raw32,VDDM_RCLUSSDTC_raw32,VDDM_RMLUSSDTC_raw32,VDDM_RMRUSSDTC_raw32,VDDM_RCRUSSDTC_raw32,VDDM_FLLUSSDTC_raw32,VDDM_FLRUSSDTC_raw32,VDDM_RLLUSSDTC_raw32,VDDM_RLRUSSDTC_raw32,VDDM_FCM2NoComDTC_raw32,VDDM_FCM2RCErrDTC_raw32,VDDM_FCM2CSErrDTC_raw32,VDDM_FCM3NoComDTC_raw32,VDDM_FCM3RCErrDTC_raw32,VDDM_FCM3CSErrDTC_raw32,VDDM_FCM4NoComDTC_raw32,VDDM_FCM4CSErrDTC_raw32,VDDM_FCM5NoComDTC_raw32,VDDM_FCM5CSErrDTC_raw32,VDDM_ZoneSCPNoComDTC_raw32,VDDM_BMSSigErrDetDTC_raw32,VDDM_FCMACCSigErrDetDTC_raw32,VDDM_FrMCUSigErrDetDTC_raw32,VDDM_RrMCUSigErrDetDTC_raw32,VDDM_CCUSigErrDetDTC_raw32,VDDM_ACCAccelCmdErrDetDTC_raw32,VDDM_ACCMalfuncDetDTC_raw32,VDDM_CCMalfuncDetDTC_raw32,VDDM_MSAMalfuncDetDTC_raw32,VDDM_ISAMalfuncDetDTC_raw32,VDDM_MCUF1RCErrDTC_raw32,VDDM_MCUR1RCErrDTC_raw32,VDDM_MCUF1CSErrDTC_raw32,VDDM_MCUR1CSErrDTC_raw32,VDDM_Shifter1RCErrDTC_raw32,VDDM_Shifter1CSErrDTC_raw32,VDDM_ESC7RCErrDTC_raw32,VDDM_ESC7CSErrDTC_raw32,VDDM_ESC1RCErrDTC_raw32,VDDM_ESC1CSErrDTC_raw32,VDDM_ESC5RCErrDTC_raw32,VDDM_ESC5CSErrDTC_raw32,VDDM_FrMCUTqErrDTC_raw32,VDDM_RrMCUTqErrDTC_raw32,VDDM_LFBatwarnDTC_raw32,VDDM_RFBatwarnDTC_raw32,VDDM_LRBatwarnDTC_raw32,VDDM_RRBatwarnDTC_raw32,VDDM_LFPressIndiDTC_raw32,VDDM_RFPressIndiDTC_raw32,VDDM_LRPressIndiDTC_raw32,VDDM_RRPressIndiDTC_raw32,VDDM_LFWheelTmpHighDTC_raw32,VDDM_RFWheelTmpHighDTC_raw32,VDDM_LRWheelTmpHighDTC_raw32,VDDM_RRWheelTmpHighDTC_raw32,VDDM_LFSensorFailDTC_raw32,VDDM_RFSensorFailDTC_raw32,VDDM_LRSensorFailDTC_raw32,VDDM_RRSensorFailDTC_raw32,VDDM_C1EPAS2LCDTC_raw32,VDDM_5vAPS1PwrErrDTC_raw32,VDDM_5vAPS2PwrErrDTC_raw32,VDDM_EPBLockTODTC_raw32,VDDM_EPBUnlockTODTC_raw32,VDDM_LimpHomeAct_flg,VDDM_DTCDetect_enum,VDDM_EngagePFail_flg,VDDM_DisengagePFail_flg,VDDM_VCURAPSErrLv2_flg,VDDM_VCURAPSErrLv3_flg,VDDM_EDriveSysErrShifterErr_flg,VDDM_LVSysErrPwrOutErr_flg,VDDM_HVRlyOpFail_flg,VDDM_MCUActDisFail_flg,VDDM_VCUBrkSWSta_enum,VDDM_VCUFLDoorSta_flg,VDDM_VCUFRDoorSta_flg,VDDM_VCURLDoorSta_flg,VDDM_VCURRDoorSta_flg,VDDM_SysAllowReadySta_flg,VDDM_VCUHoodSWSta_flg,VDDM_VCUTailgateSWSta_flg,VDDM_CAN1BusErrorDTC_raw32,VDDM_CAN2BusErrorDTC_raw32,VDDM_CAN3BusErrorDTC_raw32,VDDM_CAN4BusErrorDTC_raw32,VDDM_CAN5BusErrorDTC_raw32,VDDM_CAN6BusErrorDTC_raw32,VDDM_FrMCU4PreDTC_raw32,VDDM_FrMCUDisDTC_raw32,VDDM_FrMCUActDTC_raw32,VDDM_RegenErrDTC_raw32
  bus_selector5 : BusSelector  OutputSignals=VDHP_ActAPSPosn_pct,VDHP_LowIdleAccPedal_flg,VDHP_EAPS1MIN_pct,VDHP_EAPS2MIN_pct,VDHP_ResetPedalZeroPosStart_flg,VDHP_EAPS1NRM_pct,VDHP_EAPS2NRM_pct,VDHP_EAPS1RAW_pct,VDHP_EAPS2RAW_pct
  bus_selector6 : BusSelector  OutputSignals=VDID_VSS_kph,VDID_RUNTM_s,VDID_MILDIST_km,VDID_CLRDIST_km,VDID_APPD_pct,VDID_APPE_pct,VDID_ODOMETER_km,VDID_NUMPSATRIPSFLTMEMCLR_cnt,VDID_PSAR_sec,VDID_PSAL_sec,VDID_IPSAR_sec,VDID_IPSAL_sec,VDID_CPSAR_sec,VDID_CPSAL_sec,VDID_PKER_kphsqr,VDID_PKEL_kphsqr,VDID_ResetCDEODTR_km,VDID_CDEODTR_km,VDID_CDEODTL_km,VDID_QTYPSATRIPSR_cnt,VDID_QTYPSATRIPSL_cnt,VDID_PROTOCOLID_enum,VDID_CALID_cnt,VDID_ECUNAME_cnt,VDID_PKERNumerator_kphsqr,VDID_PKELNumerator_kphsqr,VDID_VinCode_cnt,VDID_DIDModelVersion_raw,VDID_DIDModelVersionChksum_raw
  bus_selector7 : BusSelector  OutputSignals=VDKC_DKCTimeSN_cnt,VDKC_DKCAuthSta_enum,VDKC_TimeSNDKCFbk_cnt,VDKC_PCommandToBCM_enum,VDKC_KeyAreaLockUnlock_enum,VDKC_KeyMissSta_flg,VDKC_ShippingMode_flg,VDKC_KeyNumSta_enum,VDKC_DkeyShowIVISta_enum,VDKC_DkeyAreaRAPSSta_enum,VDKC_KeyAreaPS_enum,VDKC_KeyAreaSPTGSta_enum,VDKC_KeyAreaPTG_enum,VDKC_UWB4Invalid_flg,VDKC_UWBOnOff_flg,VDKC_UWB3Invalid_flg,VDKC_UWB1Invalid_flg,VDKC_UWB2Invalid_flg,VDKC_UWB0Invalid_flg,VDKC_UIDBatVolt_enum,VDKC_CoordinateX_enum,VDKC_FDCSPTGDet_flg,VDKC_FDCSPTGOpen_flg,VDKC_UIDLowPowerSta_flg,VDKC_CoordinateY_enum,VDKC_AllowSleep_flg,VDKC_KeyTypeSta_enum,VDKC_CalDistance_enum,VDKC_UWBDetPTGArea_enum,VDKC_A0UWBEvent_enum,VDKC_ParkingModeCmd_enum,VDKC_KeyModeSta_enum,VDKC_ReVehData_enum,VDKC_UWB0Distance_enum,VDKC_DKeyWelcomeSta_enum,VDKC_UWB1Distance_enum,VDKC_UWB2Distance_enum,VDKC_UWB3Distance_enum,VDKC_UWB4Distance_enum,VDKC_BLERSSI_enum,VDKC_BLEdcEvent_enum,VDKC_UWB0FPP_enum,VDKC_UWB1FPP_enum,VDKC_UWB2FPP_enum,VDKC_UWB3FPP_enum,VDKC_UWB4FPP_enum,VDKC_UWBDetArea_enum,VDKC_OutputPCMDModule_enum,VDKC_FDCDKCAllowSleep_flg,VDKC_JudgeKeepUnlockZone_flg
  bus_selector8 : BusSelector  OutputSignals=VDSC_DISCTurn_flg,VDSC_DISCTargetSpd_kph,VDSC_DISCSta_enum,VDSC_DISCButtSta_flg
  bus_selector9 : BusSelector  OutputSignals=VNMM_AllCANTxReq_flg,VNMM_NMmTxReq_flg,VNMM_Awake_enum,VNMM_CSB_flg,VNMM_ErrorState_enum,VNMM_NodeID_enum,VNMM_PNI_flg,VNMM_RptMsgReq_flg,VNMM_WakeUp_enum,VNMM_ActiveWU_flg,VNMM_SysNMmSta_enum,VNMM_NetworkReq_flg
  outpmodule : Subsystem
  BOUTP_outputs : Outport  OutDataTypeStr=Bus: BOUTP_outputs
  wires:
  outpmodule/204(VOUTP_BrakeLamp_flg) -> bus_creator/204
  outpmodule/209(VOUTP_RBSD_flg) -> bus_creator/209
  outpmodule/367(VOUTP_C3CCU2RCDTC_raw32) -> bus_creator/367
  outpmodule/355(VOUTP_WinRFOpenedSta_pct) -> bus_creator/355
  outpmodule/273(VOUTP_AmbWelENFlash_enum) -> bus_creator/273
  outpmodule/1000(VOUTP_RrEDUActTq_Nm) -> bus_creator/1000
  outpmodule/999(VOUTP_FrEDUActTq_Nm) -> bus_creator/999
  outpmodule/998(VOUTP_DriverWhlTqDemRr_Nm) -> bus_creator/998
  outpmodule/996(VOUTP_RrRgnDecrSta_flg) -> bus_creator/996
  outpmodule/995(VOUTP_FrRgnDecrSta_flg) -> bus_creator/995
  outpmodule/993(VOUTP_FrActvDmpDisabReq_flg) -> bus_creator/993
  outpmodule/994(VOUTP_RrActvDmpDisabReq_flg) -> bus_creator/994
  outpmodule/992(VOUTP_PButtonSta_enum) -> bus_creator/992
  outpmodule/990(VOUTP_EVDriveMode_enum) -> bus_creator/990
  outpmodule/988(VOUTP_FrEDUAvailBrkRgnTq_Nm) -> bus_creator/988
  outpmodule/989(VOUTP_RrEDUAvailBrkRgnTq_Nm) -> bus_creator/989
  outpmodule/986(VOUTP_TqSourceFr_enum) -> bus_creator/986
  outpmodule/987(VOUTP_TqSourceRr_enum) -> bus_creator/987
  outpmodule/984(VOUTP_ModelVersionChksum_raw) -> bus_creator/984
  outpmodule/983(VOUTP_ModelVersion_raw) -> bus_creator/983
  outpmodule/981(VOUTP_LProgress_enum) -> bus_creator/981
  outpmodule/977(VOUTP_FlashS4ID_raw) -> bus_creator/977
  outpmodule/975(VOUTP_FlashS2ID_raw) -> bus_creator/975
  outpmodule/973(VOUTP_Prepresstempvalid_enum) -> bus_creator/973
  outpmodule/972(VOUTP_unlearnSfailvalid_enum) -> bus_creator/972
  outpmodule/969(VOUTP_Flashchkdatavalid_enum) -> bus_creator/969
  outpmodule/970(VOUTP_Flashdatavalid_enum) -> bus_creator/970
  outpmodule/967(VOUTP_WriteChkfinLRID_raw) -> bus_creator/967
  outpmodule/965(VOUTP_WriteChkfinLFID_raw) -> bus_creator/965
  outpmodule/1002(VOUTP_RrEDURolRgnTq_Nm) -> bus_creator/1002
  outpmodule/1003(VOUTP_FrEDUSpd_rpm) -> bus_creator/1003
  bus_selector7/7 -> outpmodule/561(VDKC_ShippingMode_flg)  "<VDKC_ShippingMode_flg>"
  bus_selector7/6 -> outpmodule/560(VDKC_KeyMissSta_flg)  "<VDKC_KeyMissSta_flg>"
  bus_selector7/4 -> outpmodule/558(VDKC_PCommandToBCM_enum)  "<VDKC_PCommandToBCM_enum>"
  BDID_outputs/1 -> bus_selector6/1
  bus_selector6/28 -> outpmodule/553(VDID_DIDModelVersion_raw)  "<VDID_DIDModelVersion_raw>"
  bus_selector6/26 -> outpmodule/551(VDID_PKELNumerator_kphsqr)  "<VDID_PKELNumerator_kphsqr>"
  bus_selector6/25 -> outpmodule/550(VDID_PKERNumerator_kphsqr)  "<VDID_PKERNumerator_kphsqr>"
  bus_selector6/23 -> outpmodule/548(VDID_CALID_cnt)  "<VDID_CALID_cnt>"
  bus_selector6/22 -> outpmodule/547(VDID_PROTOCOLID_enum)  "<VDID_PROTOCOLID_enum>"
  bus_selector6/24 -> outpmodule/549(VDID_ECUNAME_cnt)  "<VDID_ECUNAME_cnt>"
  bus_selector6/21 -> outpmodule/546(VDID_QTYPSATRIPSL_cnt)  "<VDID_QTYPSATRIPSL_cnt>"
  bus_selector6/19 -> outpmodule/544(VDID_CDEODTL_km)  "<VDID_CDEODTL_km>"
  bus_selector6/18 -> outpmodule/543(VDID_CDEODTR_km)  "<VDID_CDEODTR_km>"
  bus_selector6/13 -> outpmodule/538(VDID_CPSAR_sec)  "<VDID_CPSAR_sec>"
  bus_selector6/16 -> outpmodule/541(VDID_PKEL_kphsqr)  "<VDID_PKEL_kphsqr>"
  bus_selector6/15 -> outpmodule/540(VDID_PKER_kphsqr)  "<VDID_PKER_kphsqr>"
  bus_selector17/116 -> outpmodule/1175(VVMC_FDCVMCDrInpTqBstGn_pct)  "<VVMC_FDCVMCDrInpTqBstGn_pct>"
  bus_selector17/111 -> outpmodule/1170(VVMC_FDCVMCAPSAngleTarget_deg)  "<VVMC_FDCVMCAPSAngleTarget_deg>"
  bus_selector17/112 -> outpmodule/1171(VVMC_FDCVMCAPSRqEPSCtrl_flg)  "<VVMC_FDCVMCAPSRqEPSCtrl_flg>"
  bus_selector17/113 -> outpmodule/1172(VVMC_FDCVMCAngCtrlTqWtGn_pct)  "<VVMC_FDCVMCAngCtrlTqWtGn_pct>"
  bus_selector17/110 -> outpmodule/1169(VVMC_FDCVMCAPSVRqEPSCtrl_flg)  "<VVMC_FDCVMCAPSVRqEPSCtrl_flg>"
  bus_selector17/109 -> outpmodule/1168(VVMC_CalibratedGyroZ_Dps)  "<VVMC_CalibratedGyroZ_Dps>"
  bus_selector17/108 -> outpmodule/1167(VVMC_CalibratedGyroY_Dps)  "<VVMC_CalibratedGyroY_Dps>"
  bus_selector17/106 -> outpmodule/1165(VVMC_CalibratedAccZ_G)  "<VVMC_CalibratedAccZ_G>"
  bus_selector17/107 -> outpmodule/1166(VVMC_CalibratedGyroX_Dps)  "<VVMC_CalibratedGyroX_Dps>"
  bus_selector17/104 -> outpmodule/1163(VVMC_CalibratedAccX_G)  "<VVMC_CalibratedAccX_G>"
  bus_selector17/103 -> outpmodule/1162(VVMC_ExtraMSACtrlSta_enum)  "<VVMC_ExtraMSACtrlSta_enum>"
  bus_selector17/102 -> outpmodule/1161(VVMC_CAASActive_flg)  "<VVMC_CAASActive_flg>"
  bus_selector17/101 -> outpmodule/1160(VVMC_CAASCtrlAvail_flg)  "<VVMC_CAASCtrlAvail_flg>"
  bus_selector17/100 -> outpmodule/1159(VVMC_ActStESCYaw_Dps)  "<VVMC_ActStESCYaw_Dps>"
  bus_selector17/97 -> outpmodule/1156(VVMC_LongAcc_Gps)  "<VVMC_LongAcc_Gps>"
  bus_selector17/95 -> outpmodule/1154(VVMC_APSDecReq_mps2)  "<VVMC_APSDecReq_mps2>"
  bus_selector17/96 -> outpmodule/1155(VVMC_APSReq_enum)  "<VVMC_APSReq_enum>"
  bus_selector17/94 -> outpmodule/1153(VVMC_APSDecReqA_flg)  "<VVMC_APSDecReqA_flg>"
  bus_selector17/91 -> outpmodule/1150(VVMC_APSCtrlAvail_flg)  "<VVMC_APSCtrlAvail_flg>"
  bus_selector17/93 -> outpmodule/1152(VVMC_APSStaSys_enum)  "<VVMC_APSStaSys_enum>"
  bus_selector17/87 -> outpmodule/1146(VVMC_ACCPedalOvrd_flg)  "<VVMC_ACCPedalOvrd_flg>"
  bus_selector17/85 -> outpmodule/1144(VVMC_FCMLDWFault_flg)  "<VVMC_FCMLDWFault_flg>"
  bus_selector17/89 -> outpmodule/1148(VVMC_CCCtrlSta_enum)  "<VVMC_CCCtrlSta_enum>"
  bus_selector17/88 -> outpmodule/1147(VVMC_TimeGapCalcu_s)  "<VVMC_TimeGapCalcu_s>"
  bus_selector17/86 -> outpmodule/1145(VVMC_ACCCtrlAvail_flg)  "<VVMC_ACCCtrlAvail_flg>"
  bus_selector17/82 -> outpmodule/1141(VVMC_ADASLanecurveR_raw32)  "<VVMC_ADASLanecurveR_raw32>"
  bus_selector17/79 -> outpmodule/1138(VVMC_ADASLanetypeR_enum)  "<VVMC_ADASLanetypeR_enum>"
  bus_selector17/80 -> outpmodule/1139(VVMC_ADASLanetypeL_enum)  "<VVMC_ADASLanetypeL_enum>"
  bus_selector17/78 -> outpmodule/1137(VVMC_FCMACCmode_enum)  "<VVMC_FCMACCmode_enum>"
  bus_selector17/81 -> outpmodule/1140(VVMC_ADASLanecurveL_raw32)  "<VVMC_ADASLanecurveL_raw32>"
  bus_selector17/74 -> outpmodule/1133(VVMC_LVDAFailinfo_flg)  "<VVMC_LVDAFailinfo_flg>"
  bus_selector17/73 -> outpmodule/1132(VVMC_LVDAMuteSta_enum)  "<VVMC_LVDAMuteSta_enum>"
  bus_selector17/72 -> outpmodule/1131(VVMC_LVDADisabled_flg)  "<VVMC_LVDADisabled_flg>"
  bus_selector17/68 -> outpmodule/1127(VVMC_ADASISASta_enum)  "<VVMC_ADASISASta_enum>"
  bus_selector17/70 -> outpmodule/1129(VVMC_ADASFCWMute_flg)  "<VVMC_ADASFCWMute_flg>"
  bus_selector17/71 -> outpmodule/1130(VVMC_ADASLFCHandsOffWarning_enum)  "<VVMC_ADASLFCHandsOffWarning_enum>"
  bus_selector17/69 -> outpmodule/1128(VVMC_ADASLDWMute_flg)  "<VVMC_ADASLDWMute_flg>"
  bus_selector17/66 -> outpmodule/1125(VVMC_ADASLaneModeR_enum)  "<VVMC_ADASLaneModeR_enum>"
  outpmodule/279(VOUTP_AmbColorSta2_enum) -> bus_creator/279
  bus_selector4/132 -> outpmodule/489(VDDM_LimpHomeAct_flg)  "<VDDM_LimpHomeAct_flg>"
  bus_selector4/131 -> outpmodule/488(VDDM_EPBUnlockTODTC_raw32)  "<VDDM_EPBUnlockTODTC_raw32>"
  bus_selector4/130 -> outpmodule/487(VDDM_EPBLockTODTC_raw32)  "<VDDM_EPBLockTODTC_raw32>"
  bus_selector4/129 -> outpmodule/486(VDDM_5vAPS2PwrErrDTC_raw32)  "<VDDM_5vAPS2PwrErrDTC_raw32>"
  bus_selector4/124 -> outpmodule/481(VDDM_RFSensorFailDTC_raw32)  "<VDDM_RFSensorFailDTC_raw32>"
  bus_selector4/123 -> outpmodule/480(VDDM_LFSensorFailDTC_raw32)  "<VDDM_LFSensorFailDTC_raw32>"
  bus_selector4/119 -> outpmodule/476(VDDM_LFWheelTmpHighDTC_raw32)  "<VDDM_LFWheelTmpHighDTC_raw32>"
  bus_selector4/116 -> outpmodule/473(VDDM_RFPressIndiDTC_raw32)  "<VDDM_RFPressIndiDTC_raw32>"
  bus_selector4/117 -> outpmodule/474(VDDM_LRPressIndiDTC_raw32)  "<VDDM_LRPressIndiDTC_raw32>"
  bus_selector4/114 -> outpmodule/471(VDDM_RRBatwarnDTC_raw32)  "<VDDM_RRBatwarnDTC_raw32>"
  bus_selector4/107 -> outpmodule/464(VDDM_ESC5RCErrDTC_raw32)  "<VDDM_ESC5RCErrDTC_raw32>"
  bus_selector4/106 -> outpmodule/463(VDDM_ESC1CSErrDTC_raw32)  "<VDDM_ESC1CSErrDTC_raw32>"
  bus_selector4/105 -> outpmodule/462(VDDM_ESC1RCErrDTC_raw32)  "<VDDM_ESC1RCErrDTC_raw32>"
  bus_selector4/104 -> outpmodule/461(VDDM_ESC7CSErrDTC_raw32)  "<VDDM_ESC7CSErrDTC_raw32>"
  bus_selector4/103 -> outpmodule/460(VDDM_ESC7RCErrDTC_raw32)  "<VDDM_ESC7RCErrDTC_raw32>"
  bus_selector4/102 -> outpmodule/459(VDDM_Shifter1CSErrDTC_raw32)  "<VDDM_Shifter1CSErrDTC_raw32>"
  bus_selector4/101 -> outpmodule/458(VDDM_Shifter1RCErrDTC_raw32)  "<VDDM_Shifter1RCErrDTC_raw32>"
  bus_selector4/99 -> outpmodule/456(VDDM_MCUF1CSErrDTC_raw32)  "<VDDM_MCUF1CSErrDTC_raw32>"
  bus_selector4/97 -> outpmodule/454(VDDM_MCUF1RCErrDTC_raw32)  "<VDDM_MCUF1RCErrDTC_raw32>"
  bus_selector4/95 -> outpmodule/452(VDDM_MSAMalfuncDetDTC_raw32)  "<VDDM_MSAMalfuncDetDTC_raw32>"
  bus_selector4/93 -> outpmodule/450(VDDM_ACCMalfuncDetDTC_raw32)  "<VDDM_ACCMalfuncDetDTC_raw32>"
  bus_selector4/92 -> outpmodule/449(VDDM_ACCAccelCmdErrDetDTC_raw32)  "<VDDM_ACCAccelCmdErrDetDTC_raw32>"
  bus_selector4/89 -> outpmodule/446(VDDM_FrMCUSigErrDetDTC_raw32)  "<VDDM_FrMCUSigErrDetDTC_raw32>"
  bus_selector4/91 -> outpmodule/448(VDDM_CCUSigErrDetDTC_raw32)  "<VDDM_CCUSigErrDetDTC_raw32>"
  bus_selector2/116 -> outpmodule/119(VAPM_MCPressureV_bar)  "<VAPM_MCPressureV_bar>"
  bus_selector2/118 -> outpmodule/121(VAPM_BrkSwSta_flg)  "<VAPM_BrkSwSta_flg>"
  bus_selector2/113 -> outpmodule/116(VAPM_LatAccelVTimeOut_flg)  "<VAPM_LatAccelVTimeOut_flg>"
  bus_selector2/115 -> outpmodule/118(VAPM_LongAccelVTimeOut_flg)  "<VAPM_LongAccelVTimeOut_flg>"
  bus_selector2/111 -> outpmodule/114(VAPM_YawRateVTimeOut_flg)  "<VAPM_YawRateVTimeOut_flg>"
  bus_selector2/112 -> outpmodule/115(VAPM_LatAccelV_flg)  "<VAPM_LatAccelV_flg>"
  bus_selector2/109 -> outpmodule/112(VAPM_MCPressureTimeOut_flg)  "<VAPM_MCPressureTimeOut_flg>"
  bus_selector2/110 -> outpmodule/113(VAPM_YawRateV_flg)  "<VAPM_YawRateV_flg>"
  bus_selector2/105 -> outpmodule/108(VAPM_LatAccelTimeOut_flg)  "<VAPM_LatAccelTimeOut_flg>"
  bus_selector2/133 -> outpmodule/136(VAPM_EPBStaTimeOut_flg)  "<VAPM_EPBStaTimeOut_flg>"
  bus_selector2/126 -> outpmodule/129(VAPM_EPBExtReleaseAvail_flg)  "<VAPM_EPBExtReleaseAvail_flg>"
  bus_selector2/128 -> outpmodule/131(VAPM_EPBExtApplyAvail_flg)  "<VAPM_EPBExtApplyAvail_flg>"
  bus_selector2/131 -> outpmodule/134(VAPM_EPBErrStaTimeOut_flg)  "<VAPM_EPBErrStaTimeOut_flg>"
  bus_selector2/129 -> outpmodule/132(VAPM_EPBExtApplyAvailTimeOut_flg)  "<VAPM_EPBExtApplyAvailTimeOut_flg>"
  bus_selector2/127 -> outpmodule/130(VAPM_EPBExtReleaseAvailTimeOut_flg)  "<VAPM_EPBExtReleaseAvailTimeOut_flg>"
  bus_selector2/130 -> outpmodule/133(VAPM_EPBErrSta_enum)  "<VAPM_EPBErrSta_enum>"
  bus_selector2/125 -> outpmodule/128(VAPM_ESCAPSStaTimeOut_flg)  "<VAPM_ESCAPSStaTimeOut_flg>"
  bus_selector2/121 -> outpmodule/124(VAPM_BrkSwVTimeOut_flg)  "<VAPM_BrkSwVTimeOut_flg>"
  bus_selector2/122 -> outpmodule/125(VAPM_ESCStandstill_flg)  "<VAPM_ESCStandstill_flg>"
  bus_selector2/120 -> outpmodule/123(VAPM_BrkSwV_flg)  "<VAPM_BrkSwV_flg>"
  bus_selector2/119 -> outpmodule/122(VAPM_BrkSwStaTimeOut_flg)  "<VAPM_BrkSwStaTimeOut_flg>"
  bus_selector3/127 -> outpmodule/305(VBCM_HBeamADB_enum)  "<VBCM_HBeamADB_enum>"
  bus_selector3/128 -> outpmodule/306(VBCM_WalkInUnLkENMem_enum)  "<VBCM_WalkInUnLkENMem_enum>"
  bus_selector3/126 -> outpmodule/304(VBCM_FDHandleCmd_enum)  "<VBCM_FDHandleCmd_enum>"
  bus_selector3/124 -> outpmodule/302(VBCM_FDLHandleLampCmd_flg)  "<VBCM_FDLHandleLampCmd_flg>"
  bus_selector3/122 -> outpmodule/300(VBCM_TurnSwTimeSetSta123_enum)  "<VBCM_TurnSwTimeSetSta123_enum>"
  bus_selector3/121 -> outpmodule/299(VBCM_OutMode_enum)  "<VBCM_OutMode_enum>"
  bus_selector3/118 -> outpmodule/296(VBCM_TurnSwTSetSta_enum)  "<VBCM_TurnSwTSetSta_enum>"
  bus_selector3/117 -> outpmodule/295(VBCM_TurnSwSta_enum)  "<VBCM_TurnSwSta_enum>"
  bus_selector3/111 -> outpmodule/289(VBCM_AmbBrightnessSta7_enum)  "<VBCM_AmbBrightnessSta7_enum>"
  bus_selector3/112 -> outpmodule/290(VBCM_HazardIND_flg)  "<VBCM_HazardIND_flg>"
  bus_selector3/114 -> outpmodule/292(VBCM_PassSWSta_flg)  "<VBCM_PassSWSta_flg>"
  bus_selector3/104 -> outpmodule/282(VBCM_AmbColorSta5_enum)  "<VBCM_AmbColorSta5_enum>"
  bus_selector3/105 -> outpmodule/283(VBCM_AmbColorSta7_enum)  "<VBCM_AmbColorSta7_enum>"
  bus_selector3/131 -> outpmodule/309(VBCM_LockSettingStaMem_enum)  "<VBCM_LockSettingStaMem_enum>"
  bus_selector3/102 -> outpmodule/280(VBCM_AmbColorSta3_enum)  "<VBCM_AmbColorSta3_enum>"
  bus_selector3/103 -> outpmodule/281(VBCM_AmbColorSta4_enum)  "<VBCM_AmbColorSta4_enum>"
  bus_selector3/100 -> outpmodule/278(VBCM_AmbColorSta1_enum)  "<VBCM_AmbColorSta1_enum>"
  bus_selector3/130 -> outpmodule/308(VBCM_RmLpModeENMem_enum)  "<VBCM_RmLpModeENMem_enum>"
  bus_selector3/96 -> outpmodule/274(VBCM_AmbDimENFlash_enum)  "<VBCM_AmbDimENFlash_enum>"
  bus_selector3/95 -> outpmodule/273(VBCM_AmbWelENFlash_enum)  "<VBCM_AmbWelENFlash_enum>"
  bus_selector3/94 -> outpmodule/272(VBCM_AmbFunENFlash_enum)  "<VBCM_AmbFunENFlash_enum>"
  bus_selector3/90 -> outpmodule/268(VBCM_LockAlarm_enum)  "<VBCM_LockAlarm_enum>"
  bus_selector3/129 -> outpmodule/307(VBCM_WalkOutLkENMem_enum)  "<VBCM_WalkOutLkENMem_enum>"
  bus_selector6/27 -> outpmodule/552(VDID_VinCode_cnt)  "<VDID_VinCode_cnt>"
  bus_selector3/93 -> outpmodule/271(VBCM_UserNow_enum)  "<VBCM_UserNow_enum>"
  bus_selector3/92 -> outpmodule/270(VBCM_fUnlockSingle_flg)  "<VBCM_fUnlockSingle_flg>"
  bus_selector3/89 -> outpmodule/267(VBCM_AmbBrightSta_enum)  "<VBCM_AmbBrightSta_enum>"
  bus_selector3/88 -> outpmodule/266(VBCM_AmbColorSta_enum)  "<VBCM_AmbColorSta_enum>"
  bus_selector3/86 -> outpmodule/264(VBCM_AmbPwrWarnEN_flg)  "<VBCM_AmbPwrWarnEN_flg>"
  bus_selector3/83 -> outpmodule/261(VBCM_AmbWelEN_flg)  "<VBCM_AmbWelEN_flg>"
  bus_selector3/85 -> outpmodule/263(VBCM_AmbLinkDriSta_flg)  "<VBCM_AmbLinkDriSta_flg>"
  bus_selector3/81 -> outpmodule/259(VBCM_APMDoorControlSta_flg)  "<VBCM_APMDoorControlSta_flg>"
  bus_selector3/84 -> outpmodule/262(VBCM_AmbDimEN_flg)  "<VBCM_AmbDimEN_flg>"
  outpmodule/183(VOUTP_BCMDoorLockSta_flg) -> bus_creator/183
  outpmodule/182(VOUTP_AllDoorSW_flg) -> bus_creator/182
  outpmodule/180(VOUTP_TailgateRemote_enum) -> bus_creator/180
  outpmodule/179(VOUTP_AntitheftSta_enum) -> bus_creator/179
  bus_selector13/97 -> outpmodule/984(VTPM_ModelVersionChksum_raw)  "<VTPM_ModelVersionChksum_raw>"
  bus_selector13/94 -> outpmodule/981(VTPM_LProgress_enum)  "<VTPM_LProgress_enum>"
  bus_selector13/95 -> outpmodule/982(VTPM_TPMSSensorIDRegStart_flg)  "<VTPM_TPMSSensorIDRegStart_flg>"
  bus_selector13/92 -> outpmodule/979(VTPM_WritingCnt_enum)  "<VTPM_WritingCnt_enum>"
  bus_selector13/93 -> outpmodule/980(VTPM_TPMSTLCmd_flg)  "<VTPM_TPMSTLCmd_flg>"
  bus_selector13/89 -> outpmodule/976(VTPM_FlashS3ID_raw)  "<VTPM_FlashS3ID_raw>"
  bus_selector13/88 -> outpmodule/975(VTPM_FlashS2ID_raw)  "<VTPM_FlashS2ID_raw>"
  bus_selector13/87 -> outpmodule/974(VTPM_FlashS1ID_raw)  "<VTPM_FlashS1ID_raw>"
  bus_selector13/86 -> outpmodule/973(VTPM_Prepresstempvalid_enum)  "<VTPM_Prepresstempvalid_enum>"
  bus_selector13/85 -> outpmodule/972(VTPM_unlearnSfailvalid_enum)  "<VTPM_unlearnSfailvalid_enum>"
  bus_selector13/84 -> outpmodule/971(VTPM_unlearnSfali_flg)  "<VTPM_unlearnSfali_flg>"
  bus_selector13/83 -> outpmodule/970(VTPM_Flashdatavalid_enum)  "<VTPM_Flashdatavalid_enum>"
  bus_selector13/81 -> outpmodule/968(VTPM_WriteChkfinRRID_raw)  "<VTPM_WriteChkfinRRID_raw>"
  bus_selector13/78 -> outpmodule/965(VTPM_WriteChkfinLFID_raw)  "<VTPM_WriteChkfinLFID_raw>"
  outpmodule/447(VOUTP_RrMCUSigErrDetDTC_raw32) -> bus_creator/447
  outpmodule/443(VOUTP_ZoneSCPNoComDTC_raw32) -> bus_creator/443
  outpmodule/444(VOUTP_BMSSigErrDetDTC_raw32) -> bus_creator/444
  outpmodule/445(VOUTP_FCMACCSigErrDetDTC_raw32) -> bus_creator/445
  outpmodule/442(VOUTP_FCM5CSErrDTC_raw32) -> bus_creator/442
  outpmodule/440(VOUTP_FCM4CSErrDTC_raw32) -> bus_creator/440
  outpmodule/436(VOUTP_FCM3NoComDTC_raw32) -> bus_creator/436
  outpmodule/434(VOUTP_FCM2RCErrDTC_raw32) -> bus_creator/434
  outpmodule/435(VOUTP_FCM2CSErrDTC_raw32) -> bus_creator/435
  outpmodule/432(VOUTP_RLRUSSDTC_raw32) -> bus_creator/432
  outpmodule/433(VOUTP_FCM2NoComDTC_raw32) -> bus_creator/433
  outpmodule/431(VOUTP_RLLUSSDTC_raw32) -> bus_creator/431
  outpmodule/429(VOUTP_FLLUSSDTC_raw32) -> bus_creator/429
  outpmodule/430(VOUTP_FLRUSSDTC_raw32) -> bus_creator/430
  outpmodule/428(VOUTP_RCRUSSDTC_raw32) -> bus_creator/428
  outpmodule/427(VOUTP_RMRUSSDTC_raw32) -> bus_creator/427
  outpmodule/426(VOUTP_RMLUSSDTC_raw32) -> bus_creator/426
  outpmodule/181(VOUTP_HornCtrl_flg) -> bus_creator/181
  outpmodule/424(VOUTP_FCRUSSDTC_raw32) -> bus_creator/424
  outpmodule/425(VOUTP_RCLUSSDTC_raw32) -> bus_creator/425
  outpmodule/422(VOUTP_FMLUSSDTC_raw32) -> bus_creator/422
  outpmodule/421(VOUTP_FCLUSSDTC_raw32) -> bus_creator/421
  outpmodule/420(VOUTP_DiagRRTSDTC_raw32) -> bus_creator/420
  outpmodule/418(VOUTP_DiagFRTSDTC_raw32) -> bus_creator/418
  outpmodule/498(VOUTP_MCUActDisFail_flg) -> bus_creator/498
  outpmodule/493(VOUTP_VCURAPSErrLv2_flg) -> bus_creator/493
  outpmodule/490(VOUTP_DTCDetect_enum) -> bus_creator/490
  outpmodule/491(VOUTP_EngagePFail_flg) -> bus_creator/491
  outpmodule/485(VOUTP_5vAPS1PwrErrDTC_raw32) -> bus_creator/485
  outpmodule/482(VOUTP_LRSensorFailDTC_raw32) -> bus_creator/482
  outpmodule/481(VOUTP_RFSensorFailDTC_raw32) -> bus_creator/481
  outpmodule/476(VOUTP_LFWheelTmpHighDTC_raw32) -> bus_creator/476
  outpmodule/475(VOUTP_RRPressIndiDTC_raw32) -> bus_creator/475
  bus_selector4/113 -> outpmodule/470(VDDM_LRBatwarnDTC_raw32)  "<VDDM_LRBatwarnDTC_raw32>"
  outpmodule/474(VOUTP_LRPressIndiDTC_raw32) -> bus_creator/474
  outpmodule/470(VOUTP_LRBatwarnDTC_raw32) -> bus_creator/470
  outpmodule/469(VOUTP_RFBatwarnDTC_raw32) -> bus_creator/469
  outpmodule/468(VOUTP_LFBatwarnDTC_raw32) -> bus_creator/468
  outpmodule/461(VOUTP_ESC7CSErrDTC_raw32) -> bus_creator/461
  outpmodule/460(VOUTP_ESC7RCErrDTC_raw32) -> bus_creator/460
  outpmodule/458(VOUTP_Shifter1RCErrDTC_raw32) -> bus_creator/458
  outpmodule/457(VOUTP_MCUR1CSErrDTC_raw32) -> bus_creator/457
  outpmodule/495(VOUTP_EDriveSysErrShifterErr_flg) -> bus_creator/495
  outpmodule/497(VOUTP_HVRlyOpFail_flg) -> bus_creator/497
  outpmodule/496(VOUTP_LVSysErrPwrOutErr_flg) -> bus_creator/496
  bus_selector3/29 -> outpmodule/207(VBCM_RDRL_flg)  "<VBCM_RDRL_flg>"
  outpmodule/369(VOUTP_C3CCU2LCDTC_raw32) -> bus_creator/369
  bus_selector4/122 -> outpmodule/479(VDDM_RRWheelTmpHighDTC_raw32)  "<VDDM_RRWheelTmpHighDTC_raw32>"
  bus_selector10/41 -> outpmodule/661(VPMM_HWResetSta_enum)  "<VPMM_HWResetSta_enum>"
  bus_selector10/37 -> outpmodule/657(VPMM_CtrlFrPwrStbA1P_flg)  "<VPMM_CtrlFrPwrStbA1P_flg>"
  bus_selector10/36 -> outpmodule/656(VPMM_LVSilentChrgLv_enum)  "<VPMM_LVSilentChrgLv_enum>"
  bus_selector10/31 -> outpmodule/651(VPMM_TimerAllowSleep_flg)  "<VPMM_TimerAllowSleep_flg>"
  bus_selector10/25 -> outpmodule/645(VPMM_EvccAplusPwrUpReq_flg)  "<VPMM_EvccAplusPwrUpReq_flg>"
  bus_selector10/26 -> outpmodule/646(VPMM_PwrStaONTOPopReq_flg)  "<VPMM_PwrStaONTOPopReq_flg>"
  bus_selector10/24 -> outpmodule/644(VPMM_ReVehThdChkSta_enum)  "<VPMM_ReVehThdChkSta_enum>"
  bus_selector17/92 -> outpmodule/1151(VVMC_APSActive_flg)  "<VVMC_APSActive_flg>"
  bus_selector10/17 -> outpmodule/637(VPMM_DrSeatSta_enum)  "<VPMM_DrSeatSta_enum>"
  bus_selector10/9 -> outpmodule/629(VPMM_HVSysReadyToCharge_enum)  "<VPMM_HVSysReadyToCharge_enum>"
  bus_selector10/10 -> outpmodule/630(VPMM_PowerSta_enum)  "<VPMM_PowerSta_enum>"
  bus_selector10/7 -> outpmodule/627(VPMM_DCDCVoltSetpoint_V)  "<VPMM_DCDCVoltSetpoint_V>"
  bus_selector10/2 -> outpmodule/622(VPMM_PowerDownState_enum)  "<VPMM_PowerDownState_enum>"
  BTPM_outputs/1 -> bus_selector13/1
  bus_selector13/25 -> outpmodule/912(VTPM_LRPressIndi_enum)  "<VTPM_LRPressIndi_enum>"
  bus_selector13/24 -> outpmodule/911(VTPM_RFPressIndi_enum)  "<VTPM_RFPressIndi_enum>"
  bus_selector13/18 -> outpmodule/905(VTPM_LRWheelDebug_flg)  "<VTPM_LRWheelDebug_flg>"
  bus_selector13/19 -> outpmodule/906(VTPM_RFWheelDebug_flg)  "<VTPM_RFWheelDebug_flg>"
  bus_selector13/13 -> outpmodule/900(VTPM_LFSensorFail_flg)  "<VTPM_LFSensorFail_flg>"
  bus_selector13/6 -> outpmodule/893(VTPM_RFWheelPress_raw8)  "<VTPM_RFWheelPress_raw8>"
  bus_selector13/1 -> outpmodule/888(VTPM_LFBatWarn_flg)  "<VTPM_LFBatWarn_flg>"
  bus_selector2/89 -> outpmodule/92(VAPM_EPSAOIControlTimeOut_flg)  "<VAPM_EPSAOIControlTimeOut_flg>"
  bus_selector2/50 -> outpmodule/53(VAPM_RRRawWhlSpeed_kph)  "<VAPM_RRRawWhlSpeed_kph>"
  bus_selector2/46 -> outpmodule/49(VAPM_RFRawWhlSpeed_kph)  "<VAPM_RFRawWhlSpeed_kph>"
  bus_selector2/43 -> outpmodule/46(VAPM_BrkPedalPosTimeOut_flg)  "<VAPM_BrkPedalPosTimeOut_flg>"
  bus_selector2/134 -> outpmodule/137(VAPM_AVMparkingcancel_enum)  "<VAPM_AVMparkingcancel_enum>"
  bus_selector2/40 -> outpmodule/43(VAPM_StaFSya_flg)  "<VAPM_StaFSya_flg>"
  bus_selector2/41 -> outpmodule/44(VAPM_ModOperation_enum)  "<VAPM_ModOperation_enum>"
  outpmodule/923(VOUTP_CWheelTips_enum) -> bus_creator/923
  outpmodule/920(VOUTP_LRWheelPSW_raw8) -> bus_creator/920
  outpmodule/914(VOUTP_TPMSWarnIndi_enum) -> bus_creator/914
  outpmodule/488(VOUTP_EPBUnlockTODTC_raw32) -> bus_creator/488
  outpmodule/912(VOUTP_LRPressIndi_enum) -> bus_creator/912
  outpmodule/910(VOUTP_LFPressIndi_enum) -> bus_creator/910
  bus_selector3/109 -> outpmodule/287(VBCM_AmbBrightnessSta4_enum)  "<VBCM_AmbBrightnessSta4_enum>"
  outpmodule/907(VOUTP_RRWheelDebug_flg) -> bus_creator/907
  outpmodule/904(VOUTP_LFWheelDebug_flg) -> bus_creator/904
  outpmodule/901(VOUTP_RFSensorFail_flg) -> bus_creator/901
  outpmodule/356(VOUTP_WinLROpenedSta_pct) -> bus_creator/356
  outpmodule/902(VOUTP_LRSensorFail_flg) -> bus_creator/902
  outpmodule/898(VOUTP_LRWheelTemp_C) -> bus_creator/898
  outpmodule/978(VOUTP_FlashIDvalid_enum) -> bus_creator/978
  outpmodule/899(VOUTP_RRWheelTemp_C) -> bus_creator/899
  bus_selector2/124 -> outpmodule/127(VAPM_ESCAPSSta_enum)  "<VAPM_ESCAPSSta_enum>"
  outpmodule/925(VOUTP_LFSensorMode_flg) -> bus_creator/925
  outpmodule/514(VOUTP_FrMCUDisDTC_raw32) -> bus_creator/514
  outpmodule/509(VOUTP_CAN3BusErrorDTC_raw32) -> bus_creator/509
  bus_selector13/76 -> outpmodule/963(VTPM_WriteChkLRID_raw)  "<VTPM_WriteChkLRID_raw>"
  outpmodule/504(VOUTP_SysAllowReadySta_flg) -> bus_creator/504
  outpmodule/503(VOUTP_VCURRDoorSta_flg) -> bus_creator/503
  outpmodule/502(VOUTP_VCURLDoorSta_flg) -> bus_creator/502
  outpmodule/499(VOUTP_VCUBrkSWSta_enum) -> bus_creator/499
  bus_selector2/59 -> outpmodule/62(VAPM_RRRawWhlSpeedVTimeOut_flg)  "<VAPM_RRRawWhlSpeedVTimeOut_flg>"
  bus_selector2/55 -> outpmodule/58(VAPM_RFRawWhlSpeedVTimeOut_flg)  "<VAPM_RFRawWhlSpeedVTimeOut_flg>"
  bus_selector10/38 -> outpmodule/658(VPMM_CtrlFrRC1_flg)  "<VPMM_CtrlFrRC1_flg>"
  bus_selector2/54 -> outpmodule/57(VAPM_RFRawWhlSpeedV_flg)  "<VAPM_RFRawWhlSpeedV_flg>"
  bus_selector2/52 -> outpmodule/55(VAPM_LFRawWhlSpeedV_flg)  "<VAPM_LFRawWhlSpeedV_flg>"
  bus_selector12/175 -> outpmodule/886(VTHC_FDCFGSFuncSta_flg)  "<VTHC_FDCFGSFuncSta_flg>"
  bus_selector12/176 -> outpmodule/887(VTHC_THSysErrlampReq_flg)  "<VTHC_THSysErrlampReq_flg>"
  bus_selector12/169 -> outpmodule/880(VTHC_FrostSet_enum)  "<VTHC_FrostSet_enum>"
  bus_selector12/170 -> outpmodule/881(VTHC_LVentEN_flg)  "<VTHC_LVentEN_flg>"
  bus_selector13/68 -> outpmodule/955(VTPM_ChkStorge_flg)  "<VTPM_ChkStorge_flg>"
  bus_selector13/69 -> outpmodule/956(VTPM_TPMSResButt_flg)  "<VTPM_TPMSResButt_flg>"
  bus_selector13/65 -> outpmodule/952(VTPM_Chkfin_flg)  "<VTPM_Chkfin_flg>"
  bus_selector13/61 -> outpmodule/948(VTPM_ID1messageALTU_raw8)  "<VTPM_ID1messageALTU_raw8>"
  bus_selector13/58 -> outpmodule/945(VTPM_S2WheelDebugALTU_pct)  "<VTPM_S2WheelDebugALTU_pct>"
  bus_selector13/60 -> outpmodule/947(VTPM_S4WheelDebugALTU_pct)  "<VTPM_S4WheelDebugALTU_pct>"
  bus_selector13/57 -> outpmodule/944(VTPM_S1WheelDebugALTU_pct)  "<VTPM_S1WheelDebugALTU_pct>"
  bus_selector13/55 -> outpmodule/942(VTPM_FAT_flg)  "<VTPM_FAT_flg>"
  bus_selector13/51 -> outpmodule/938(VTPM_LFP20_raw8)  "<VTPM_LFP20_raw8>"
  bus_selector13/50 -> outpmodule/937(VTPM_ALFin_flg)  "<VTPM_ALFin_flg>"
  bus_selector13/49 -> outpmodule/936(VTPM_S4L_enum)  "<VTPM_S4L_enum>"
  bus_selector13/45 -> outpmodule/932(VTPM_S4ID_raw32)  "<VTPM_S4ID_raw32>"
  bus_selector13/39 -> outpmodule/926(VTPM_RFSensorMode_flg)  "<VTPM_RFSensorMode_flg>"
  bus_selector13/30 -> outpmodule/917(VTPM_LRWheelTmpIndi_flg)  "<VTPM_LRWheelTmpIndi_flg>"
  bus_selector13/27 -> outpmodule/914(VTPM_TPMSWarnIndi_enum)  "<VTPM_TPMSWarnIndi_enum>"
  bus_selector4/120 -> outpmodule/477(VDDM_RFWheelTmpHighDTC_raw32)  "<VDDM_RFWheelTmpHighDTC_raw32>"
  outpmodule/916(VOUTP_RFWheelTmpIndi_flg) -> bus_creator/916
  bus_selector13/72 -> outpmodule/959(VTPM_LRPindi_enum)  "<VTPM_LRPindi_enum>"
  bus_selector17/10 -> outpmodule/1069(VVMC_FeatReqSpd_kph)  "<VVMC_FeatReqSpd_kph>"
  bus_selector17/11 -> outpmodule/1070(VVMC_JerkPCT_pct)  "<VVMC_JerkPCT_pct>"
  bus_selector17/12 -> outpmodule/1071(VVMC_LimitPCT_pct)  "<VVMC_LimitPCT_pct>"
  bus_selector17/6 -> outpmodule/1065(VVMC_VMCACCCtrlAvail_flg)  "<VVMC_VMCACCCtrlAvail_flg>"
  bus_selector17/7 -> outpmodule/1066(VVMC_VMCCCCtrlAvail_flg)  "<VVMC_VMCCCCtrlAvail_flg>"
  outpmodule/915(VOUTP_LFWheelTmpIndi_flg) -> bus_creator/915
  bus_selector13/46 -> outpmodule/933(VTPM_S1L_enum)  "<VTPM_S1L_enum>"
  bus_selector17/3 -> outpmodule/1062(VVMC_VehicleSpeed_kph)  "<VVMC_VehicleSpeed_kph>"
  bus_selector17/17 -> outpmodule/1076(VVMC_SafetyCtrl_flg)  "<VVMC_SafetyCtrl_flg>"
  bus_selector17/15 -> outpmodule/1074(VVMC_SingleWhlSlipRatioCtrl_flg)  "<VVMC_SingleWhlSlipRatioCtrl_flg>"
  bus_selector17/16 -> outpmodule/1075(VVMC_LatAccCtrl_flg)  "<VVMC_LatAccCtrl_flg>"
  outpmodule/67(VOUTP_LRWhlRotDir_enum) -> bus_creator/67
  outpmodule/63(VOUTP_LFWhlRotDir_enum) -> bus_creator/63
  outpmodule/62(VOUTP_RRRawWhlSpeedVTimeOut_flg) -> bus_creator/62
  outpmodule/61(VOUTP_RRRawWhlSpeedV_flg) -> bus_creator/61
  outpmodule/58(VOUTP_RFRawWhlSpeedVTimeOut_flg) -> bus_creator/58
  outpmodule/57(VOUTP_RFRawWhlSpeedV_flg) -> bus_creator/57
  outpmodule/56(VOUTP_LFRawWhlSpeedVTimeOut_flg) -> bus_creator/56
  outpmodule/917(VOUTP_LRWheelTmpIndi_flg) -> bus_creator/917
  outpmodule/55(VOUTP_LFRawWhlSpeedV_flg) -> bus_creator/55
  outpmodule/53(VOUTP_RRRawWhlSpeed_kph) -> bus_creator/53
  outpmodule/50(VOUTP_RFRawWhlSpeedTimeOut_flg) -> bus_creator/50
  outpmodule/47(VOUTP_LFRawWhlSpeed_kph) -> bus_creator/47
  outpmodule/46(VOUTP_BrkPedalPosTimeOut_flg) -> bus_creator/46
  outpmodule/45(VOUTP_BrkPedalPos_pct) -> bus_creator/45
  outpmodule/921(VOUTP_RFWheelPSW_raw8) -> bus_creator/921
  outpmodule/44(VOUTP_ModOperation_enum) -> bus_creator/44
  outpmodule/43(VOUTP_StaFSya_flg) -> bus_creator/43
  outpmodule/69(VOUTP_RRWhlRotDir_enum) -> bus_creator/69
  outpmodule/68(VOUTP_LRWhlRotDirTimeOut_flg) -> bus_creator/68
  outpmodule/848(VOUTP_FDCTHCLEVentYStaSet3_enum) -> bus_creator/848
  outpmodule/845(VOUTP_FDCTHCCREVentZStaSet7_enum) -> bus_creator/845
  bus_selector7/5 -> outpmodule/559(VDKC_KeyAreaLockUnlock_enum)  "<VDKC_KeyAreaLockUnlock_enum>"
  outpmodule/477(VOUTP_RFWheelTmpHighDTC_raw32) -> bus_creator/477
  outpmodule/918(VOUTP_RRWheelTmpIndi_flg) -> bus_creator/918
  outpmodule/846(VOUTP_FDCTHCLEVentYStaSet1_enum) -> bus_creator/846
  outpmodule/841(VOUTP_FDCTHCCREVentZStaSet2_enum) -> bus_creator/841
  outpmodule/842(VOUTP_FDCTHCCREVentZStaSet3_enum) -> bus_creator/842
  outpmodule/840(VOUTP_FDCTHCCREVentZStaSet1_enum) -> bus_creator/840
  outpmodule/837(VOUTP_FDCTHCREVentZStaSet4_enum) -> bus_creator/837
  outpmodule/836(VOUTP_FDCTHCREVentZStaSet3_enum) -> bus_creator/836
  outpmodule/834(VOUTP_FDCTHCREVentZStaSet1_enum) -> bus_creator/834
  outpmodule/833(VOUTP_FDCTHCCLEVentZStaSet7_enum) -> bus_creator/833
  outpmodule/832(VOUTP_FDCTHCCLEVentZStaSet5_enum) -> bus_creator/832
  outpmodule/829(VOUTP_FDCTHCCLEVentZStaSet2_enum) -> bus_creator/829
  bus_selector2/44 -> outpmodule/47(VAPM_LFRawWhlSpeed_kph)  "<VAPM_LFRawWhlSpeed_kph>"
  outpmodule/828(VOUTP_FDCTHCCLEVentZStaSet1_enum) -> bus_creator/828
  outpmodule/826(VOUTP_FDCTHCLEVentZStaSet5_enum) -> bus_creator/826
  outpmodule/824(VOUTP_FDCTHCLEVentZStaSet3_enum) -> bus_creator/824
  outpmodule/823(VOUTP_FDCTHCLEVentZStaSet2_enum) -> bus_creator/823
  outpmodule/976(VOUTP_FlashS3ID_raw) -> bus_creator/976
  outpmodule/825(VOUTP_FDCTHCLEVentZStaSet4_enum) -> bus_creator/825
  outpmodule/821(VOUTP_REVentModeStaSet457_enum) -> bus_creator/821
  outpmodule/822(VOUTP_FDCTHCLEVentZStaSet1_enum) -> bus_creator/822
  outpmodule/820(VOUTP_REVentModeStaSet123_enum) -> bus_creator/820
  outpmodule/818(VOUTP_LEVentModeStaSet123_enum) -> bus_creator/818
  outpmodule/966(VOUTP_WriteChkfinRFID_raw) -> bus_creator/966
  outpmodule/815(VOUTP_CLVentENSet_enum) -> bus_creator/815
  outpmodule/812(VOUTP_FDCFGSAirIntStaSet123_enum) -> bus_creator/812
  outpmodule/811(VOUTP_FDCFGSChStaSet457_enum) -> bus_creator/811
  outpmodule/208(VOUTP_LBSD_flg) -> bus_creator/208
  outpmodule/235(VOUTP_AmbLightBrightness4_enum) -> bus_creator/235
  outpmodule/233(VOUTP_AmbLightBrightness2_enum) -> bus_creator/233
  outpmodule/234(VOUTP_AmbLightBrightness3_enum) -> bus_creator/234
  outpmodule/231(VOUTP_AmbLightBreath6_enum) -> bus_creator/231
  bus_selector3/26 -> outpmodule/204(VBCM_BrakeLamp_flg)  "<VBCM_BrakeLamp_flg>"
  outpmodule/232(VOUTP_AmbLightBrightness1_enum) -> bus_creator/232
  outpmodule/228(VOUTP_AmbLightBreath3_enum) -> bus_creator/228
  bus_selector17/67 -> outpmodule/1126(VVMC_ADASSLIFSta_enum)  "<VVMC_ADASSLIFSta_enum>"
  outpmodule/229(VOUTP_AmbLightBreath4_enum) -> bus_creator/229
  outpmodule/224(VOUTP_WasherCtrl_enum) -> bus_creator/224
  outpmodule/216(VOUTP_RrDefog_flg) -> bus_creator/216
  outpmodule/218(VOUTP_RoomLampL_flg) -> bus_creator/218
  outpmodule/608(VOUTP_DISCButtSta_flg) -> bus_creator/608
  outpmodule/605(VOUTP_DISCTurn_flg) -> bus_creator/605
  outpmodule/600(VOUTP_UWB4FPP_enum) -> bus_creator/600
  bus_selector13/42 -> outpmodule/929(VTPM_S1ID_raw32)  "<VTPM_S1ID_raw32>"
  outpmodule/597(VOUTP_UWB1FPP_enum) -> bus_creator/597
  outpmodule/596(VOUTP_UWB0FPP_enum) -> bus_creator/596
  outpmodule/595(VOUTP_BLEdcEvent_enum) -> bus_creator/595
  outpmodule/589(VOUTP_DKeyWelcomeSta_enum) -> bus_creator/589
  outpmodule/588(VOUTP_UWB0Distance_enum) -> bus_creator/588
  outpmodule/587(VOUTP_ReVehData_enum) -> bus_creator/587
  outpmodule/581(VOUTP_KeyTypeSta_enum) -> bus_creator/581
  outpmodule/579(VOUTP_CoordinateY_enum) -> bus_creator/579
  outpmodule/574(VOUTP_UIDBatVolt_enum) -> bus_creator/574
  bus_selector10/16 -> outpmodule/636(VPMM_DrivetrainSelect_enum)  "<VPMM_DrivetrainSelect_enum>"
  outpmodule/573(VOUTP_UWB0Invalid_flg) -> bus_creator/573
  outpmodule/572(VOUTP_UWB2Invalid_flg) -> bus_creator/572
  bus_selector16/7 -> outpmodule/1059(VV2L_HVPO120VGrpBLDSt_enum)  "<VV2L_HVPO120VGrpBLDSt_enum>"
  BV2L_outputs/1 -> bus_selector16/1
  bus_selector16/3 -> outpmodule/1055(VV2L_ReqV2LIVIDisChrg_enum)  "<VV2L_ReqV2LIVIDisChrg_enum>"
  outpmodule/604(VOUTP_JudgeKeepUnlockZone_flg) -> bus_creator/604
  bus_selector16/2 -> outpmodule/1054(VV2L_ReqV2LIVIPopup_enum)  "<VV2L_ReqV2LIVIPopup_enum>"
  bus_selector16/4 -> outpmodule/1056(VV2L_ReqOBCExtrV2LEna_enum)  "<VV2L_ReqOBCExtrV2LEna_enum>"
  bus_selector15/7 -> outpmodule/1051(VTQR_RrRateLimitInc_Nm)  "<VTQR_RrRateLimitInc_Nm>"
  bus_selector15/8 -> outpmodule/1052(VTQR_RrRateLimitDec_Nm)  "<VTQR_RrRateLimitDec_Nm>"
  bus_selector15/3 -> outpmodule/1047(VTQR_FrFirstOrderInpTs_c)  "<VTQR_FrFirstOrderInpTs_c>"
  bus_selector15/2 -> outpmodule/1046(VTQR_RrTMTqReq_Nm)  "<VTQR_RrTMTqReq_Nm>"
  bus_selector15/6 -> outpmodule/1050(VTQR_FrRateLimitDec_Nm)  "<VTQR_FrRateLimitDec_Nm>"
  bus_selector15/4 -> outpmodule/1048(VTQR_RrFirstOrderInpTs_c)  "<VTQR_RrFirstOrderInpTs_c>"
  BVMC_outputs/1 -> bus_selector17/1
  outpmodule/467(VOUTP_RrMCUTqErrDTC_raw32) -> bus_creator/467
  outpmodule/900(VOUTP_LFSensorFail_flg) -> bus_creator/900
  bus_selector17/118 -> outpmodule/1177(VVMC_DMSModeCmd_enum)  "<VVMC_DMSModeCmd_enum>"
  bus_selector2/17 -> outpmodule/20(VAPM_APSDFLL_cm)  "<VAPM_APSDFLL_cm>"
  outpmodule/459(VOUTP_Shifter1CSErrDTC_raw32) -> bus_creator/459
  bus_selector2/12 -> outpmodule/15(VAPM_PASDFCR_cm)  "<VAPM_PASDFCR_cm>"
  bus_selector2/13 -> outpmodule/16(VAPM_PASDFCL_cm)  "<VAPM_PASDFCL_cm>"
  bus_selector2/10 -> outpmodule/13(VAPM_PASDFMR_cm)  "<VAPM_PASDFMR_cm>"
  bus_selector4/88 -> outpmodule/445(VDDM_FCMACCSigErrDetDTC_raw32)  "<VDDM_FCMACCSigErrDetDTC_raw32>"
  bus_selector2/37 -> outpmodule/40(VAPM_USSStaFCL_flg)  "<VAPM_USSStaFCL_flg>"
  bus_selector17/114 -> outpmodule/1173(VVMC_FDCVMCDrInpTqBstAct_flg)  "<VVMC_FDCVMCDrInpTqBstAct_flg>"
  bus_selector2/33 -> outpmodule/36(VAPM_USSStaFML_flg)  "<VAPM_USSStaFML_flg>"
  bus_selector2/35 -> outpmodule/38(VAPM_USSStaFLL_flg)  "<VAPM_USSStaFLL_flg>"
  bus_selector2/31 -> outpmodule/34(VAPM_USSStaRCL_flg)  "<VAPM_USSStaRCL_flg>"
  bus_selector2/32 -> outpmodule/35(VAPM_USSStaFMR_flg)  "<VAPM_USSStaFMR_flg>"
  bus_selector2/141 -> outpmodule/144(VAPM_AVMErrSTATimeOut_flg)  "<VAPM_AVMErrSTATimeOut_flg>"
  bus_selector2/29 -> outpmodule/32(VAPM_USSStaRLL_flg)  "<VAPM_USSStaRLL_flg>"
  bus_selector2/27 -> outpmodule/30(VAPM_USSStaRML_flg)  "<VAPM_USSStaRML_flg>"
  outpmodule/896(VOUTP_LFWheelTemp_C) -> bus_creator/896
  bus_selector2/137 -> outpmodule/140(VAPM_AVMparkingexcuteTimeOut_flg)  "<VAPM_AVMparkingexcuteTimeOut_flg>"
  bus_selector2/26 -> outpmodule/29(VAPM_USSStaRMR_flg)  "<VAPM_USSStaRMR_flg>"
  bus_selector2/21 -> outpmodule/24(VAPM_PASARCR_enum)  "<VAPM_PASARCR_enum>"
  bus_selector2/20 -> outpmodule/23(VAPM_PASARML_enum)  "<VAPM_PASARML_enum>"
  bus_selector17/90 -> outpmodule/1149(VVMC_MSACtrlSta_enum)  "<VVMC_MSACtrlSta_enum>"
  bus_selector2/164 -> outpmodule/167(VAPM_DKCParkingModeCmd_enum)  "<VAPM_DKCParkingModeCmd_enum>"
  bus_selector2/149 -> outpmodule/152(VAPM_ABSActiveTimeOut_flg)  "<VAPM_ABSActiveTimeOut_flg>"
  bus_selector2/150 -> outpmodule/153(VAPM_TCSActive_flg)  "<VAPM_TCSActive_flg>"
  bus_selector2/148 -> outpmodule/151(VAPM_ABSActive_flg)  "<VAPM_ABSActive_flg>"
  bus_selector3/116 -> outpmodule/294(VBCM_FWasSwSta_enum)  "<VBCM_FWasSwSta_enum>"
  outpmodule/65(VOUTP_RFWhlRotDir_enum) -> bus_creator/65
  bus_selector2/171 -> outpmodule/174(VAPM_RAPSBCMLockReq_flg)  "<VAPM_RAPSBCMLockReq_flg>"
  bus_selector2/163 -> outpmodule/166(VAPM_DKCPDkeyAreaRAPSSta_enum)  "<VAPM_DKCPDkeyAreaRAPSSta_enum>"
  bus_selector2/159 -> outpmodule/162(VAPM_APSAngleTarget_Deg)  "<VAPM_APSAngleTarget_Deg>"
  bus_selector2/160 -> outpmodule/163(VAPM_APSVRqEPASCtrl_flg)  "<VAPM_APSVRqEPASCtrl_flg>"
  bus_selector2/155 -> outpmodule/158(VAPM_APSRQDisplay_enum)  "<VAPM_APSRQDisplay_enum>"
  bus_selector2/151 -> outpmodule/154(VAPM_TCSActiveTimeOut_flg)  "<VAPM_TCSActiveTimeOut_flg>"
  bus_selector3/115 -> outpmodule/293(VBCM_FWipSwSta_enum)  "<VBCM_FWipSwSta_enum>"
  outpmodule/211(VOUTP_LTurnLP_flg) -> bus_creator/211
  outpmodule/199(VOUTP_DimmerEN_flg) -> bus_creator/199
  outpmodule/190(VOUTP_RRDoorSW_flg) -> bus_creator/190
  outpmodule/924(VOUTP_AutoLTips_enum) -> bus_creator/924
  outpmodule/205(VOUTP_ReverseLamp_flg) -> bus_creator/205
  outpmodule/1176(VOUTP_VehPitchAngleSta_enum) -> bus_creator/1176
  bus_selector2/68 -> outpmodule/71(VAPM_LFPulseCountV_flg)  "<VAPM_LFPulseCountV_flg>"
  bus_selector2/67 -> outpmodule/70(VAPM_RRWhlRotDirTimeOut_flg)  "<VAPM_RRWhlRotDirTimeOut_flg>"
  bus_selector2/138 -> outpmodule/141(VAPM_AVMParkingmode_enum)  "<VAPM_AVMParkingmode_enum>"
  bus_selector2/63 -> outpmodule/66(VAPM_RFWhlRotDirTimeOut_flg)  "<VAPM_RFWhlRotDirTimeOut_flg>"
  bus_selector13/16 -> outpmodule/903(VTPM_RRSensorFail_flg)  "<VTPM_RRSensorFail_flg>"
  bus_selector2/64 -> outpmodule/67(VAPM_LRWhlRotDir_enum)  "<VAPM_LRWhlRotDir_enum>"
  bus_selector10/35 -> outpmodule/655(VPMM_LVSilentChrgReq_flg)  "<VPMM_LVSilentChrgReq_flg>"
  outpmodule/449(VOUTP_ACCAccelCmdErrDetDTC_raw32) -> bus_creator/449
  outpmodule/1077(VOUTP_SPD2ACCAct_flg) -> bus_creator/1077
  outpmodule/1076(VOUTP_SafetyCtrl_flg) -> bus_creator/1076
  outpmodule/1071(VOUTP_LimitPCT_pct) -> bus_creator/1071
  outpmodule/1068(VOUTP_FeatArbitrSta_enum) -> bus_creator/1068
  outpmodule/178(VOUTP_IVIUserTakeOverAPSSta_flg) -> bus_creator/178
  bus_selector4/126 -> outpmodule/483(VDDM_RRSensorFailDTC_raw32)  "<VDDM_RRSensorFailDTC_raw32>"
  outpmodule/1070(VOUTP_JerkPCT_pct) -> bus_creator/1070
  outpmodule/817(VOUTP_CRVentENSet_enum) -> bus_creator/817
  outpmodule/1067(VOUTP_VMCMSACtrlAvail_flg) -> bus_creator/1067
  outpmodule/1061(VOUTP_VehicleSpeed_mph) -> bus_creator/1061
  outpmodule/1060(VOUTP_FeatSetSpdFinal_raw32) -> bus_creator/1060
  outpmodule/1055(VOUTP_ReqV2LIVIDisChrg_enum) -> bus_creator/1055
  outpmodule/1053(VOUTP_ReqOBCV2LEna_enum) -> bus_creator/1053
  outpmodule/187(VOUTP_DrDoorSW_flg) -> bus_creator/187
  outpmodule/1052(VOUTP_RrRateLimitDec_Nm) -> bus_creator/1052
  outpmodule/1047(VOUTP_FrFirstOrderInpTs_c) -> bus_creator/1047
  outpmodule/1048(VOUTP_RrFirstOrderInpTs_c) -> bus_creator/1048
  outpmodule/1049(VOUTP_FrRateLimitInc_Nm) -> bus_creator/1049
  outpmodule/1046(VOUTP_RrTMTqReq_Nm) -> bus_creator/1046
  outpmodule/1044(VOUTP_SimSouWaveReq_pct) -> bus_creator/1044
  outpmodule/575(VOUTP_CoordinateX_enum) -> bus_creator/575
  outpmodule/1042(VOUTP_SlideRegenLimTq_Nm) -> bus_creator/1042
  outpmodule/1079(VOUTP_ISOAccLimit_mps2) -> bus_creator/1079
  bus_selector2/145 -> outpmodule/148(VAPM_CAASSwTimeOut_flg)  "<VAPM_CAASSwTimeOut_flg>"
  bus_selector2/72 -> outpmodule/75(VAPM_LRPulseCountV_flg)  "<VAPM_LRPulseCountV_flg>"
  bus_selector2/70 -> outpmodule/73(VAPM_RFPulseCountV_flg)  "<VAPM_RFPulseCountV_flg>"
  bus_selector2/73 -> outpmodule/76(VAPM_LRPulseCountVTimeOut_flg)  "<VAPM_LRPulseCountVTimeOut_flg>"
  bus_selector2/71 -> outpmodule/74(VAPM_RFPulseCountVTimeOut_flg)  "<VAPM_RFPulseCountVTimeOut_flg>"
  bus_selector2/7 -> outpmodule/10(VAPM_PASDRML_cm)  "<VAPM_PASDRML_cm>"
  bus_selector2/6 -> outpmodule/9(VAPM_PASDRMR_cm)  "<VAPM_PASDRMR_cm>"
  bus_selector2/5 -> outpmodule/8(VAPM_ChrgPlugSta_enum)  "<VAPM_ChrgPlugSta_enum>"
  bus_selector2/1 -> outpmodule/4(VAPM_VehSpeed_kph)  "<VAPM_VehSpeed_kph>"
  bus_selector17/9 -> outpmodule/1068(VVMC_FeatArbitrSta_enum)  "<VVMC_FeatArbitrSta_enum>"
  bus_selector2/175 -> outpmodule/178(VAPM_IVIUserTakeOverAPSSta_flg)  "<VAPM_IVIUserTakeOverAPSSta_flg>"
  bus_selector2/173 -> outpmodule/176(VAPM_RAPSErrWarnSta_enum)  "<VAPM_RAPSErrWarnSta_enum>"
  outpmodule/1164(VOUTP_CalibratedAccY_G) -> bus_creator/1164
  outpmodule/1059(VOUTP_HVPO120VGrpBLDSt_enum) -> bus_creator/1059
  outpmodule/1165(VOUTP_CalibratedAccZ_G) -> bus_creator/1165
  outpmodule/1156(VOUTP_LongAcc_Gps) -> bus_creator/1156
  outpmodule/1158(VOUTP_IMUEnaCmd_flg) -> bus_creator/1158
  outpmodule/1154(VOUTP_APSDecReq_mps2) -> bus_creator/1154
  outpmodule/1173(VOUTP_FDCVMCDrInpTqBstAct_flg) -> bus_creator/1173
  outpmodule/1168(VOUTP_CalibratedGyroZ_Dps) -> bus_creator/1168
  outpmodule/1169(VOUTP_FDCVMCAPSVRqEPSCtrl_flg) -> bus_creator/1169
  bus_selector2/34 -> outpmodule/37(VAPM_USSStaFLR_flg)  "<VAPM_USSStaFLR_flg>"
  outpmodule/1167(VOUTP_CalibratedGyroY_Dps) -> bus_creator/1167
  outpmodule/1086(VOUTP_LateralCtrl_flg) -> bus_creator/1086
  outpmodule/1085(VOUTP_ActACCRequiredAccel_mps2) -> bus_creator/1085
  bus_selector10/4 -> outpmodule/624(VPMM_PowerDownFault_enum)  "<VPMM_PowerDownFault_enum>"
  outpmodule/1083(VOUTP_DISCReqAcc_mps2) -> bus_creator/1083
  outpmodule/1081(VOUTP_ISOJerkLimit_mps3) -> bus_creator/1081
  outpmodule/1105(VOUTP_ADASShftPosnReqA_flg) -> bus_creator/1105
  bus_selector4/118 -> outpmodule/475(VDDM_RRPressIndiDTC_raw32)  "<VDDM_RRPressIndiDTC_raw32>"
  outpmodule/979(VOUTP_WritingCnt_enum) -> bus_creator/979
  outpmodule/1101(VOUTP_ACCComfortBandUpper_mps2) -> bus_creator/1101
  bus_selector7/1 -> outpmodule/555(VDKC_DKCTimeSN_cnt)  "<VDKC_DKCTimeSN_cnt>"
  outpmodule/1102(VOUTP_ACCJerkLowerLimit_mps3) -> bus_creator/1102
  outpmodule/219(VOUTP_TrunkRel_flg) -> bus_creator/219
  outpmodule/1099(VOUTP_TimeGapLevel_enum) -> bus_creator/1099
  outpmodule/1098(VOUTP_ACCObjRelSpd_mps) -> bus_creator/1098
  outpmodule/1096(VOUTP_ADASACCSta_enum) -> bus_creator/1096
  outpmodule/1097(VOUTP_ACCObjDist_m) -> bus_creator/1097
  outpmodule/225(VOUTP_WiperFixMode_flg) -> bus_creator/225
  outpmodule/897(VOUTP_RFWheelTemp_C) -> bus_creator/897
  outpmodule/1094(VOUTP_ACCVehHoldReq_flg) -> bus_creator/1094
  outpmodule/1093(VOUTP_AEBVehHoldReq_flg) -> bus_creator/1093
  outpmodule/1092(VOUTP_ADASFaultSta_flg) -> bus_creator/1092
  outpmodule/201(VOUTP_LBeam_flg) -> bus_creator/201
  outpmodule/191(VOUTP_LockSetting_flg) -> bus_creator/191
  bus_selector4/82 -> outpmodule/439(VDDM_FCM4NoComDTC_raw32)  "<VDDM_FCM4NoComDTC_raw32>"
  bus_selector4/79 -> outpmodule/436(VDDM_FCM3NoComDTC_raw32)  "<VDDM_FCM3NoComDTC_raw32>"
  bus_selector4/80 -> outpmodule/437(VDDM_FCM3RCErrDTC_raw32)  "<VDDM_FCM3RCErrDTC_raw32>"
  bus_selector4/77 -> outpmodule/434(VDDM_FCM2RCErrDTC_raw32)  "<VDDM_FCM2RCErrDTC_raw32>"
  bus_selector4/74 -> outpmodule/431(VDDM_RLLUSSDTC_raw32)  "<VDDM_RLLUSSDTC_raw32>"
  bus_selector13/22 -> outpmodule/909(VTPM_TPMSCaliButtAllow_flg)  "<VTPM_TPMSCaliButtAllow_flg>"
  bus_selector2/107 -> outpmodule/110(VAPM_LongAccelTimeOut_flg)  "<VAPM_LongAccelTimeOut_flg>"
  bus_selector4/76 -> outpmodule/433(VDDM_FCM2NoComDTC_raw32)  "<VDDM_FCM2NoComDTC_raw32>"
  bus_selector17/77 -> outpmodule/1136(VVMC_ADASLFCWarnSound_enum)  "<VVMC_ADASLFCWarnSound_enum>"
  bus_selector4/70 -> outpmodule/427(VDDM_RMRUSSDTC_raw32)  "<VDDM_RMRUSSDTC_raw32>"
  bus_selector4/64 -> outpmodule/421(VDDM_FCLUSSDTC_raw32)  "<VDDM_FCLUSSDTC_raw32>"
  bus_selector4/63 -> outpmodule/420(VDDM_DiagRRTSDTC_raw32)  "<VDDM_DiagRRTSDTC_raw32>"
  bus_selector4/57 -> outpmodule/414(VDDM_ESC5NoComDTC_raw32)  "<VDDM_ESC5NoComDTC_raw32>"
  outpmodule/1082(VOUTP_ACCRequiredAccel_mps2) -> bus_creator/1082
  bus_selector4/49 -> outpmodule/406(VDDM_APS1SigOoRDTC_raw32)  "<VDDM_APS1SigOoRDTC_raw32>"
  bus_selector4/48 -> outpmodule/405(VDDM_VehMalfunLevel_enum)  "<VDDM_VehMalfunLevel_enum>"
  bus_selector17/5 -> outpmodule/1064(VVMC_VMCAEBCtrlAvail_flg)  "<VVMC_VMCAEBCtrlAvail_flg>"
  bus_selector4/46 -> outpmodule/403(VDDM_TailgaSWDTC_raw32)  "<VDDM_TailgaSWDTC_raw32>"
  outpmodule/506(VOUTP_VCUTailgateSWSta_flg) -> bus_creator/506
  bus_selector4/44 -> outpmodule/401(VDDM_RRDoorSWDTC_raw32)  "<VDDM_RRDoorSWDTC_raw32>"
  bus_selector4/43 -> outpmodule/400(VDDM_FRDoorSWDTC_raw32)  "<VDDM_FRDoorSWDTC_raw32>"
  bus_selector4/42 -> outpmodule/399(VDDM_RLDoorSWDTC_raw32)  "<VDDM_RLDoorSWDTC_raw32>"
  bus_selector4/37 -> outpmodule/394(VDDM_IniLVLoDTC_raw32)  "<VDDM_IniLVLoDTC_raw32>"
  outpmodule/894(VOUTP_LRWheelPress_raw8) -> bus_creator/894
  bus_selector4/40 -> outpmodule/397(VDDM_DrStSWDTC_raw32)  "<VDDM_DrStSWDTC_raw32>"
  bus_selector4/39 -> outpmodule/396(VDDM_LVSupHiDTC_raw32)  "<VDDM_LVSupHiDTC_raw32>"
  outpmodule/210(VOUTP_HazardSW_flg) -> bus_creator/210
  bus_selector10/6 -> outpmodule/626(VPMM_DCDCEnaReq_flg)  "<VPMM_DCDCEnaReq_flg>"
  bus_selector4/85 -> outpmodule/442(VDDM_FCM5CSErrDTC_raw32)  "<VDDM_FCM5CSErrDTC_raw32>"
  bus_selector4/134 -> outpmodule/491(VDDM_EngagePFail_flg)  "<VDDM_EngagePFail_flg>"
  outpmodule/21(VOUTP_PASAFCL_enum) -> bus_creator/21
  outpmodule/20(VOUTP_APSDFLL_cm) -> bus_creator/20
  outpmodule/19(VOUTP_APSDFLR_cm) -> bus_creator/19
  bus_selector2/102 -> outpmodule/105(VAPM_YawRate_degps)  "<VAPM_YawRate_degps>"
  outpmodule/18(VOUTP_APSDRLL_cm) -> bus_creator/18
  outpmodule/17(VOUTP_APSDRLR_cm) -> bus_creator/17
  outpmodule/455(VOUTP_MCUR1RCErrDTC_raw32) -> bus_creator/455
  outpmodule/16(VOUTP_PASDFCL_cm) -> bus_creator/16
  outpmodule/15(VOUTP_PASDFCR_cm) -> bus_creator/15
  outpmodule/14(VOUTP_PASDFML_cm) -> bus_creator/14
  outpmodule/7(VOUTP_FSOffSwTimeOut_flg) -> bus_creator/7
  outpmodule/5(VOUTP_VehSpeedTimeOut_flg) -> bus_creator/5
  outpmodule/42(VOUTP_SNSRLayout_enum) -> bus_creator/42
  outpmodule/39(VOUTP_USSStaFCR_flg) -> bus_creator/39
  outpmodule/36(VOUTP_USSStaFML_flg) -> bus_creator/36
  bus_selector13/34 -> outpmodule/921(VTPM_RFWheelPSW_raw8)  "<VTPM_RFWheelPSW_raw8>"
  outpmodule/35(VOUTP_USSStaFMR_flg) -> bus_creator/35
  outpmodule/1157(VOUTP_CCMSASpdWar_flg) -> bus_creator/1157
  outpmodule/30(VOUTP_USSStaRML_flg) -> bus_creator/30
  bus_selector13/31 -> outpmodule/918(VTPM_RRWheelTmpIndi_flg)  "<VTPM_RRWheelTmpIndi_flg>"
  outpmodule/451(VOUTP_CCMalfuncDetDTC_raw32) -> bus_creator/451
  outpmodule/27(VOUTP_PASAFML_enum) -> bus_creator/27
  bus_selector2/19 -> outpmodule/22(VAPM_PASARMR_enum)  "<VAPM_PASARMR_enum>"
  outpmodule/28(VOUTP_PASAFCR_enum) -> bus_creator/28
  outpmodule/25(VOUTP_PASARCL_enum) -> bus_creator/25
  outpmodule/24(VOUTP_PASARCR_enum) -> bus_creator/24
  outpmodule/1064(VOUTP_VMCAEBCtrlAvail_flg) -> bus_creator/1064
  outpmodule/23(VOUTP_PASARML_enum) -> bus_creator/23
  bus_selector15/1 -> outpmodule/1045(VTQR_FrTMTqReq_Nm)  "<VTQR_FrTMTqReq_Nm>"
  bus_selector14/60 -> outpmodule/1044(VTQD_SimSouWaveReq_pct)  "<VTQD_SimSouWaveReq_pct>"
  bus_selector14/59 -> outpmodule/1043(VTQD_SimSoundCmd_pct)  "<VTQD_SimSoundCmd_pct>"
  bus_selector14/56 -> outpmodule/1040(VTQD_TrailerDisOPDSta_flg)  "<VTQD_TrailerDisOPDSta_flg>"
  outpmodule/184(VOUTP_AntitheftSeatFlod_flg) -> bus_creator/184
  bus_selector14/57 -> outpmodule/1041(VTQD_ForceP_flg)  "<VTQD_ForceP_flg>"
  outpmodule/448(VOUTP_CCUSigErrDetDTC_raw32) -> bus_creator/448
  bus_selector4/61 -> outpmodule/418(VDDM_DiagFRTSDTC_raw32)  "<VDDM_DiagFRTSDTC_raw32>"
  bus_selector14/53 -> outpmodule/1037(VTQD_RegenLimIndSta_flg)  "<VTQD_RegenLimIndSta_flg>"
  bus_selector14/52 -> outpmodule/1036(VTQD_VehActSpd_kph)  "<VTQD_VehActSpd_kph>"
  bus_selector2/91 -> outpmodule/94(VAPM_SASAngleTimeOut_flg)  "<VAPM_SASAngleTimeOut_flg>"
  bus_selector14/55 -> outpmodule/1039(VTQD_MaxWhlSlideRate_pct)  "<VTQD_MaxWhlSlideRate_pct>"
  bus_selector14/48 -> outpmodule/1032(VTQD_FDCVCURegenMode_enum)  "<VTQD_FDCVCURegenMode_enum>"
  outpmodule/1161(VOUTP_CAASActive_flg) -> bus_creator/1161
  bus_selector14/47 -> outpmodule/1031(VTQD_SaveRegenMode_enum)  "<VTQD_SaveRegenMode_enum>"
  bus_selector14/44 -> outpmodule/1028(VTQD_RegenTqLimitEn_flg)  "<VTQD_RegenTqLimitEn_flg>"
  bus_selector14/42 -> outpmodule/1026(VTQD_DriveProtEn_flg)  "<VTQD_DriveProtEn_flg>"
  outpmodule/1170(VOUTP_FDCVMCAPSAngleTarget_deg) -> bus_creator/1170
  bus_selector14/41 -> outpmodule/1025(VTQD_EquivAccPedalSWSta_flg)  "<VTQD_EquivAccPedalSWSta_flg>"
  outpmodule/227(VOUTP_AmbLightBreath2_enum) -> bus_creator/227
  bus_selector14/39 -> outpmodule/1023(VTQD_CreepON_flg)  "<VTQD_CreepON_flg>"
  bus_selector14/33 -> outpmodule/1017(VTQD_RrIdcMin_A)  "<VTQD_RrIdcMin_A>"
  bus_selector14/38 -> outpmodule/1022(VTQD_BOSEnable_flg)  "<VTQD_BOSEnable_flg>"
  bus_selector14/34 -> outpmodule/1018(VTQD_RrIdcMax_A)  "<VTQD_RrIdcMax_A>"
  outpmodule/416(VOUTP_DiagHCrashDTC_raw32) -> bus_creator/416
  bus_selector2/81 -> outpmodule/84(VAPM_LRPulseCountTimeOut_flg)  "<VAPM_LRPulseCountTimeOut_flg>"
  bus_selector14/35 -> outpmodule/1019(VTQD_RrUdcMin_V)  "<VTQD_RrUdcMin_V>"
  outpmodule/196(VOUTP_DoorLockIND_flg) -> bus_creator/196
  bus_selector13/62 -> outpmodule/949(VTPM_ID2messageALTU_raw8)  "<VTPM_ID2messageALTU_raw8>"
  bus_selector4/94 -> outpmodule/451(VDDM_CCMalfuncDetDTC_raw32)  "<VDDM_CCMalfuncDetDTC_raw32>"
  outpmodule/272(VOUTP_AmbFunENFlash_enum) -> bus_creator/272
  outpmodule/816(VOUTP_RVentENSet_enum) -> bus_creator/816
  outpmodule/248(VOUTP_IVIRST_flg) -> bus_creator/248
  outpmodule/486(VOUTP_5vAPS2PwrErrDTC_raw32) -> bus_creator/486
  bus_selector10/15 -> outpmodule/635(VPMM_RrMCUEnaReq_flg)  "<VPMM_RrMCUEnaReq_flg>"
  outpmodule/250(VOUTP_MFSWTri_flg) -> bus_creator/250
  outpmodule/267(VOUTP_AmbBrightSta_enum) -> bus_creator/267
  outpmodule/266(VOUTP_AmbColorSta_enum) -> bus_creator/266
  outpmodule/54(VOUTP_RRRawWhlSpeedTimeOut_flg) -> bus_creator/54
  outpmodule/270(VOUTP_fUnlockSingle_flg) -> bus_creator/270
  bus_selector13/47 -> outpmodule/934(VTPM_S2L_enum)  "<VTPM_S2L_enum>"
  outpmodule/269(VOUTP_ATCtrl_enum) -> bus_creator/269
  outpmodule/274(VOUTP_AmbDimENFlash_enum) -> bus_creator/274
  bus_selector2/76 -> outpmodule/79(VAPM_LFPulseCount_enum)  "<VAPM_LFPulseCount_enum>"
  bus_selector2/78 -> outpmodule/81(VAPM_RFPulseCount_enum)  "<VAPM_RFPulseCount_enum>"
  outpmodule/64(VOUTP_LFWhlRotDirTimeOut_flg) -> bus_creator/64
  bus_selector2/77 -> outpmodule/80(VAPM_LFPulseCountTimeOut_flg)  "<VAPM_LFPulseCountTimeOut_flg>"
  bus_selector2/75 -> outpmodule/78(VAPM_RRPulseCountVTimeOut_flg)  "<VAPM_RRPulseCountVTimeOut_flg>"
  outpmodule/52(VOUTP_LRRawWhlSpeedTimeOut_flg) -> bus_creator/52
  outpmodule/366(VOUTP_C3CCU1LCDTC_raw32) -> bus_creator/366
  bus_selector4/98 -> outpmodule/455(VDDM_MCUR1RCErrDTC_raw32)  "<VDDM_MCUR1RCErrDTC_raw32>"
  outpmodule/1144(VOUTP_FCMLDWFault_flg) -> bus_creator/1144
  outpmodule/1140(VOUTP_ADASLanecurveL_raw32) -> bus_creator/1140
  outpmodule/1142(VOUTP_ADASAEBSta_enum) -> bus_creator/1142
  outpmodule/1139(VOUTP_ADASLanetypeL_enum) -> bus_creator/1139
  outpmodule/1138(VOUTP_ADASLanetypeR_enum) -> bus_creator/1138
  outpmodule/1135(VOUTP_LVDAACCStatusInformation_flg) -> bus_creator/1135
  outpmodule/1136(VOUTP_ADASLFCWarnSound_enum) -> bus_creator/1136
  outpmodule/849(VOUTP_FDCTHCLEVentYStaSet4_enum) -> bus_creator/849
  outpmodule/1134(VOUTP_LVDAWarning_flg) -> bus_creator/1134
  outpmodule/610(VOUTP_NMmTxReq_flg) -> bus_creator/610
  outpmodule/1149(VOUTP_MSACtrlSta_enum) -> bus_creator/1149
  outpmodule/452(VOUTP_MSAMalfuncDetDTC_raw32) -> bus_creator/452
  outpmodule/1148(VOUTP_CCCtrlSta_enum) -> bus_creator/1148
  outpmodule/591(VOUTP_UWB2Distance_enum) -> bus_creator/591
  outpmodule/1147(VOUTP_TimeGapCalcu_s) -> bus_creator/1147
  outpmodule/413(VOUTP_ESC1NoComDTC_raw32) -> bus_creator/413
  outpmodule/411(VOUTP_Shifter1NoComDTC_raw32) -> bus_creator/411
  outpmodule/407(VOUTP_APS2SigOoRDTC_raw32) -> bus_creator/407
  bus_selector2/48 -> outpmodule/51(VAPM_LRRawWhlSpeed_kph)  "<VAPM_LRRawWhlSpeed_kph>"
  outpmodule/409(VOUTP_MCUF1NoComDTC_raw32) -> bus_creator/409
  bus_selector2/69 -> outpmodule/72(VAPM_LFPulseCountVTimeOut_flg)  "<VAPM_LFPulseCountVTimeOut_flg>"
  outpmodule/405(VOUTP_VehMalfunLevel_enum) -> bus_creator/405
  outpmodule/406(VOUTP_APS1SigOoRDTC_raw32) -> bus_creator/406
  outpmodule/402(VOUTP_HoodSWDTC_raw32) -> bus_creator/402
  outpmodule/403(VOUTP_TailgaSWDTC_raw32) -> bus_creator/403
  outpmodule/400(VOUTP_FRDoorSWDTC_raw32) -> bus_creator/400
  outpmodule/847(VOUTP_FDCTHCLEVentYStaSet2_enum) -> bus_creator/847
  outpmodule/399(VOUTP_RLDoorSWDTC_raw32) -> bus_creator/399
  outpmodule/398(VOUTP_FLDoorSWDTC_raw32) -> bus_creator/398
  outpmodule/396(VOUTP_LVSupHiDTC_raw32) -> bus_creator/396
  bus_selector17/1 -> outpmodule/1060(VVMC_FeatSetSpdFinal_raw32)  "<VVMC_FeatSetSpdFinal_raw32>"
  outpmodule/395(VOUTP_LVSupLoDTC_raw32) -> bus_creator/395
  bus_selector3/120 -> outpmodule/298(VBCM_SPTGENFunMem_enum)  "<VBCM_SPTGENFunMem_enum>"
  outpmodule/843(VOUTP_FDCTHCCREVentZStaSet4_enum) -> bus_creator/843
  outpmodule/394(VOUTP_IniLVLoDTC_raw32) -> bus_creator/394
  outpmodule/392(VOUTP_MCUActDTC_raw32) -> bus_creator/392
  outpmodule/393(VOUTP_OBC4PreDTC_raw32) -> bus_creator/393
  outpmodule/391(VOUTP_HVRlyOpDTC_raw32) -> bus_creator/391
  outpmodule/387(VOUTP_HiLvSaChkDTC_raw32) -> bus_creator/387
  outpmodule/389(VOUTP_MCUDisDTC_raw32) -> bus_creator/389
  outpmodule/386(VOUTP_DCDCEnaDTC_raw32) -> bus_creator/386
  outpmodule/911(VOUTP_RFPressIndi_enum) -> bus_creator/911
  outpmodule/385(VOUTP_BMSRdyDTC_raw32) -> bus_creator/385
  bus_selector13/79 -> outpmodule/966(VTPM_WriteChkfinRFID_raw)  "<VTPM_WriteChkfinRFID_raw>"
  outpmodule/381(VOUTP_HVB4PreDTC_raw32) -> bus_creator/381
  outpmodule/378(VOUTP_BrkSWNoBacDTC_raw32) -> bus_creator/378
  outpmodule/376(VOUTP_Lv4ErrDTC_raw32) -> bus_creator/376
  outpmodule/374(VOUTP_Lv2ErrDTC_raw32) -> bus_creator/374
  bus_selector10/13 -> outpmodule/633(VPMM_SysPowerMode_enum)  "<VPMM_SysPowerMode_enum>"
  bus_selector17/99 -> outpmodule/1158(VVMC_IMUEnaCmd_flg)  "<VVMC_IMUEnaCmd_flg>"
  outpmodule/913(VOUTP_RRPressIndi_enum) -> bus_creator/913
  bus_selector13/21 -> outpmodule/908(VTPM_TPMSResButtAllow_flg)  "<VTPM_TPMSResButtAllow_flg>"
  outpmodule/375(VOUTP_Lv3ErrDTC_raw32) -> bus_creator/375
  bus_selector6/29 -> outpmodule/554(VDID_DIDModelVersionChksum_raw)  "<VDID_DIDModelVersionChksum_raw>"
  outpmodule/1118(VOUTP_ADASCAMSpdLim_enum) -> bus_creator/1118
  bus_selector2/88 -> outpmodule/91(VAPM_EPSAOIControl_enum)  "<VAPM_EPSAOIControl_enum>"
  outpmodule/1115(VOUTP_ForceLowBeam_enum) -> bus_creator/1115
  outpmodule/1112(VOUTP_ADASLDWSta_enum) -> bus_creator/1112
  bus_selector10/18 -> outpmodule/638(VPMM_PwrStaSelect_enum)  "<VPMM_PwrStaSelect_enum>"
  outpmodule/827(VOUTP_FDCTHCLEVentZStaSet7_enum) -> bus_creator/827
  outpmodule/1108(VOUTP_HazardWarningReq_flg) -> bus_creator/1108
  outpmodule/580(VOUTP_AllowSleep_flg) -> bus_creator/580
  outpmodule/1129(VOUTP_ADASFCWMute_flg) -> bus_creator/1129
  outpmodule/1127(VOUTP_ADASISASta_enum) -> bus_creator/1127
  outpmodule/1122(VOUTP_LKAHODSoundWarning_flg) -> bus_creator/1122
  outpmodule/1123(VOUTP_ADASLFCSta_enum) -> bus_creator/1123
  outpmodule/594(VOUTP_BLERSSI_enum) -> bus_creator/594
  outpmodule/1120(VOUTP_ADASSLIFSpdLim_enum) -> bus_creator/1120
  outpmodule/1121(VOUTP_LKAHODDisplayWarning_flg) -> bus_creator/1121
  outpmodule/6(VOUTP_FSOffSw_enum) -> bus_creator/6
  outpmodule/194(VOUTP_CrashDetd_flg) -> bus_creator/194
  outpmodule/1119(VOUTP_TargetType_enum) -> bus_creator/1119
  bus_selector3/28 -> outpmodule/206(VBCM_LDRL_flg)  "<VBCM_LDRL_flg>"
  outpmodule/960(VOUTP_RRPindi_enum) -> bus_creator/960
  outpmodule/961(VOUTP_WriteChkLFID_raw) -> bus_creator/961
  bus_selector10/1 -> outpmodule/621(VPMM_PowerUpState_enum)  "<VPMM_PowerUpState_enum>"
  outpmodule/609(VOUTP_AllCANTxReq_flg) -> bus_creator/609
  outpmodule/959(VOUTP_LRPindi_enum) -> bus_creator/959
  outpmodule/957(VOUTP_LFPindi_enum) -> bus_creator/957
  bus_selector17/4 -> outpmodule/1063(VVMC_MeterIndSpeed_raw32)  "<VVMC_MeterIndSpeed_raw32>"
  outpmodule/954(VOUTP_TPMSStorge_flg) -> bus_creator/954
  outpmodule/956(VOUTP_TPMSResButt_flg) -> bus_creator/956
  bus_selector13/17 -> outpmodule/904(VTPM_LFWheelDebug_flg)  "<VTPM_LFWheelDebug_flg>"
  bus_selector17/76 -> outpmodule/1135(VVMC_LVDAACCStatusInformation_flg)  "<VVMC_LVDAACCStatusInformation_flg>"
  outpmodule/844(VOUTP_FDCTHCCREVentZStaSet5_enum) -> bus_creator/844
  outpmodule/952(VOUTP_Chkfin_flg) -> bus_creator/952
  outpmodule/950(VOUTP_ID3messageALTU_raw8) -> bus_creator/950
  bus_selector13/48 -> outpmodule/935(VTPM_S3L_enum)  "<VTPM_S3L_enum>"
  outpmodule/949(VOUTP_ID2messageALTU_raw8) -> bus_creator/949
  outpmodule/947(VOUTP_S4WheelDebugALTU_pct) -> bus_creator/947
  outpmodule/945(VOUTP_S2WheelDebugALTU_pct) -> bus_creator/945
  outpmodule/941(VOUTP_RRP20_raw8) -> bus_creator/941
  outpmodule/940(VOUTP_LRP20_raw8) -> bus_creator/940
  bus_selector2/65 -> outpmodule/68(VAPM_LRWhlRotDirTimeOut_flg)  "<VAPM_LRWhlRotDirTimeOut_flg>"
  outpmodule/942(VOUTP_FAT_flg) -> bus_creator/942
  outpmodule/939(VOUTP_RFP20_raw8) -> bus_creator/939
  bus_selector10/34 -> outpmodule/654(VPMM_LVSilentChrgSta_enum)  "<VPMM_LVSilentChrgSta_enum>"
  outpmodule/937(VOUTP_ALFin_flg) -> bus_creator/937
  bus_selector17/117 -> outpmodule/1176(VVMC_VehPitchAngleSta_enum)  "<VVMC_VehPitchAngleSta_enum>"
  outpmodule/933(VOUTP_S1L_enum) -> bus_creator/933
  outpmodule/934(VOUTP_S2L_enum) -> bus_creator/934
  outpmodule/930(VOUTP_S2ID_raw32) -> bus_creator/930
  bus_selector16/5 -> outpmodule/1057(VV2L_ReqOBCIntrV2LEna_enum)  "<VV2L_ReqOBCIntrV2LEna_enum>"
  outpmodule/932(VOUTP_S4ID_raw32) -> bus_creator/932
  outpmodule/928(VOUTP_RRSensorMode_flg) -> bus_creator/928
  outpmodule/927(VOUTP_LRSensorMode_flg) -> bus_creator/927
  outpmodule/1056(VOUTP_ReqOBCExtrV2LEna_enum) -> bus_creator/1056
  outpmodule/963(VOUTP_WriteChkLRID_raw) -> bus_creator/963
  outpmodule/962(VOUTP_WriteChkRFID_raw) -> bus_creator/962
  bus_selector13/10 -> outpmodule/897(VTPM_RFWheelTemp_C)  "<VTPM_RFWheelTemp_C>"
  bus_selector6/11 -> outpmodule/536(VDID_IPSAR_sec)  "<VDID_IPSAR_sec>"
  outpmodule/905(VOUTP_LRWheelDebug_flg) -> bus_creator/905
  bus_selector6/7 -> outpmodule/532(VDID_ODOMETER_km)  "<VDID_ODOMETER_km>"
  bus_selector6/8 -> outpmodule/533(VDID_NUMPSATRIPSFLTMEMCLR_cnt)  "<VDID_NUMPSATRIPSFLTMEMCLR_cnt>"
  bus_selector6/5 -> outpmodule/530(VDID_APPD_pct)  "<VDID_APPD_pct>"
  bus_selector6/6 -> outpmodule/531(VDID_APPE_pct)  "<VDID_APPE_pct>"
  bus_selector6/4 -> outpmodule/529(VDID_CLRDIST_km)  "<VDID_CLRDIST_km>"
  bus_selector3/87 -> outpmodule/265(VBCM_AmbODAEN_flg)  "<VBCM_AmbODAEN_flg>"
  bus_selector10/14 -> outpmodule/634(VPMM_FrMCUEnaReq_flg)  "<VPMM_FrMCUEnaReq_flg>"
  bus_selector2/135 -> outpmodule/138(VAPM_AVMparkingcancelTimeOut_flg)  "<VAPM_AVMparkingcancelTimeOut_flg>"
  outpmodule/586(VOUTP_KeyModeSta_enum) -> bus_creator/586
  bus_selector6/2 -> outpmodule/527(VDID_RUNTM_s)  "<VDID_RUNTM_s>"
  BDHP_outputs/1 -> bus_selector5/1
  bus_selector5/8 -> outpmodule/524(VDHP_EAPS1RAW_pct)  "<VDHP_EAPS1RAW_pct>"
  bus_selector5/9 -> outpmodule/525(VDHP_EAPS2RAW_pct)  "<VDHP_EAPS2RAW_pct>"
  bus_selector5/7 -> outpmodule/523(VDHP_EAPS2NRM_pct)  "<VDHP_EAPS2NRM_pct>"
  bus_selector5/6 -> outpmodule/522(VDHP_EAPS1NRM_pct)  "<VDHP_EAPS1NRM_pct>"
  bus_selector3/107 -> outpmodule/285(VBCM_AmbBrightnessSta2_enum)  "<VBCM_AmbBrightnessSta2_enum>"
  bus_selector5/3 -> outpmodule/519(VDHP_EAPS1MIN_pct)  "<VDHP_EAPS1MIN_pct>"
  outpmodule/1074(VOUTP_SingleWhlSlipRatioCtrl_flg) -> bus_creator/1074
  bus_selector5/5 -> outpmodule/521(VDHP_ResetPedalZeroPosStart_flg)  "<VDHP_ResetPedalZeroPosStart_flg>"
  bus_selector3/110 -> outpmodule/288(VBCM_AmbBrightnessSta5_enum)  "<VBCM_AmbBrightnessSta5_enum>"
  bus_selector5/4 -> outpmodule/520(VDHP_EAPS2MIN_pct)  "<VDHP_EAPS2MIN_pct>"
  outpmodule/529(VOUTP_CLRDIST_km) -> bus_creator/529
  outpmodule/527(VOUTP_RUNTM_s) -> bus_creator/527
  outpmodule/524(VOUTP_EAPS1RAW_pct) -> bus_creator/524
  outpmodule/525(VOUTP_EAPS2RAW_pct) -> bus_creator/525
  outpmodule/523(VOUTP_EAPS2NRM_pct) -> bus_creator/523
  outpmodule/522(VOUTP_EAPS1NRM_pct) -> bus_creator/522
  outpmodule/264(VOUTP_AmbPwrWarnEN_flg) -> bus_creator/264
  outpmodule/520(VOUTP_EAPS2MIN_pct) -> bus_creator/520
  outpmodule/521(VOUTP_ResetPedalZeroPosStart_flg) -> bus_creator/521
  outpmodule/519(VOUTP_EAPS1MIN_pct) -> bus_creator/519
  outpmodule/515(VOUTP_FrMCUActDTC_raw32) -> bus_creator/515
  outpmodule/1058(VOUTP_HVPO120VGrpALDSt_enum) -> bus_creator/1058
  outpmodule/388(VOUTP_MidLvSaChkDTC_raw32) -> bus_creator/388
  outpmodule/177(VOUTP_RAPSErrLv1_flg) -> bus_creator/177
  outpmodule/176(VOUTP_RAPSErrWarnSta_enum) -> bus_creator/176
  outpmodule/175(VOUTP_APSPwrReq_enum) -> bus_creator/175
  outpmodule/173(VOUTP_RAPSBCMLamp_enum) -> bus_creator/173
  bus_selector2/80 -> outpmodule/83(VAPM_LRPulseCount_enum)  "<VAPM_LRPulseCount_enum>"
  outpmodule/171(VOUTP_APSSpeedCMD_kph) -> bus_creator/171
  outpmodule/170(VOUTP_APSShiftPosnReq_enum) -> bus_creator/170
  outpmodule/169(VOUTP_CAASVMCReqA_flg) -> bus_creator/169
  bus_selector15/5 -> outpmodule/1049(VTQR_FrRateLimitInc_Nm)  "<VTQR_FrRateLimitInc_Nm>"
  outpmodule/167(VOUTP_DKCParkingModeCmd_enum) -> bus_creator/167
  outpmodule/891(VOUTP_RRBatWarn_flg) -> bus_creator/891
  outpmodule/166(VOUTP_DKCPDkeyAreaRAPSSta_enum) -> bus_creator/166
  outpmodule/163(VOUTP_APSVRqEPASCtrl_flg) -> bus_creator/163
  outpmodule/162(VOUTP_APSAngleTarget_Deg) -> bus_creator/162
  outpmodule/161(VOUTP_APSExitCondition_enum) -> bus_creator/161
  outpmodule/159(VOUTP_APSSWVer_enum) -> bus_creator/159
  bus_selector2/161 -> outpmodule/164(VAPM_APSRqEPASCtrl_flg)  "<VAPM_APSRqEPASCtrl_flg>"
  outpmodule/249(VOUTP_CountAlarm_enum) -> bus_creator/249
  outpmodule/160(VOUTP_APSHWVer_enum) -> bus_creator/160
  outpmodule/158(VOUTP_APSRQDisplay_enum) -> bus_creator/158
  outpmodule/156(VOUTP_DriverSeatBeltCmdTimeOut_flg) -> bus_creator/156
  outpmodule/155(VOUTP_DriverSeatBeltCmd_flg) -> bus_creator/155
  outpmodule/647(VOUTP_IVIPwrStaONTOPopT_s) -> bus_creator/647
  outpmodule/648(VOUTP_LVChrgHoldTtimer_s) -> bus_creator/648
  bus_selector12/173 -> outpmodule/884(VTHC_CRVentEN_flg)  "<VTHC_CRVentEN_flg>"
  outpmodule/12(VOUTP_PASDRCL_cm) -> bus_creator/12
  outpmodule/646(VOUTP_PwrStaONTOPopReq_flg) -> bus_creator/646
  outpmodule/645(VOUTP_EvccAplusPwrUpReq_flg) -> bus_creator/645
  outpmodule/643(VOUTP_LowSOCWarn_enum) -> bus_creator/643
  outpmodule/642(VOUTP_PwrDownReq_enum) -> bus_creator/642
  outpmodule/641(VOUTP_PwrUpReq_enum) -> bus_creator/641
  outpmodule/640(VOUTP_TCountSta_enum) -> bus_creator/640
  outpmodule/639(VOUTP_PwrStaConstraint_enum) -> bus_creator/639
  outpmodule/637(VOUTP_DrSeatSta_enum) -> bus_creator/637
  outpmodule/638(VOUTP_PwrStaSelect_enum) -> bus_creator/638
  outpmodule/636(VOUTP_DrivetrainSelect_enum) -> bus_creator/636
  outpmodule/1131(VOUTP_LVDADisabled_flg) -> bus_creator/1131
  outpmodule/634(VOUTP_FrMCUEnaReq_flg) -> bus_creator/634
  outpmodule/633(VOUTP_SysPowerMode_enum) -> bus_creator/633
  outpmodule/480(VOUTP_LFSensorFailDTC_raw32) -> bus_creator/480
  outpmodule/631(VOUTP_LVPwrSta_flg) -> bus_creator/631
  outpmodule/630(VOUTP_PowerSta_enum) -> bus_creator/630
  outpmodule/627(VOUTP_DCDCVoltSetpoint_V) -> bus_creator/627
  outpmodule/628(VOUTP_HVBatCnctReq_flg) -> bus_creator/628
  bus_selector2/49 -> outpmodule/52(VAPM_LRRawWhlSpeedTimeOut_flg)  "<VAPM_LRRawWhlSpeedTimeOut_flg>"
  bus_selector4/38 -> outpmodule/395(VDDM_LVSupLoDTC_raw32)  "<VDDM_LVSupLoDTC_raw32>"
  outpmodule/625(VOUTP_ActiveDischargeReq_flg) -> bus_creator/625
  bus_selector13/73 -> outpmodule/960(VTPM_RRPindi_enum)  "<VTPM_RRPindi_enum>"
  outpmodule/626(VOUTP_DCDCEnaReq_flg) -> bus_creator/626
  outpmodule/623(VOUTP_PowerUpFault_enum) -> bus_creator/623
  outpmodule/624(VOUTP_PowerDownFault_enum) -> bus_creator/624
  outpmodule/622(VOUTP_PowerDownState_enum) -> bus_creator/622
  bus_selector2/165 -> outpmodule/168(VAPM_PUIDLowPower_flg)  "<VAPM_PUIDLowPower_flg>"
  outpmodule/620(VOUTP_NetworkReq_flg) -> bus_creator/620
  outpmodule/1078(VOUTP_AccCalcuPID_mps2) -> bus_creator/1078
  outpmodule/621(VOUTP_PowerUpState_enum) -> bus_creator/621
  outpmodule/48(VOUTP_LFRawWhlSpeedTimeOut_flg) -> bus_creator/48
  outpmodule/618(VOUTP_ActiveWU_flg) -> bus_creator/618
  outpmodule/478(VOUTP_LRWheelTmpHighDTC_raw32) -> bus_creator/478
  outpmodule/617(VOUTP_WakeUp_enum) -> bus_creator/617
  outpmodule/616(VOUTP_RptMsgReq_flg) -> bus_creator/616
  outpmodule/614(VOUTP_NodeID_enum) -> bus_creator/614
  outpmodule/613(VOUTP_ErrorState_enum) -> bus_creator/613
  outpmodule/189(VOUTP_RLDoorSW_flg) -> bus_creator/189
  outpmodule/611(VOUTP_Awake_enum) -> bus_creator/611
  bus_selector2/87 -> outpmodule/90(VAPM_DriIntendTimeOut_flg)  "<VAPM_DriIntendTimeOut_flg>"
  outpmodule/649(VOUTP_LVBattChrgTimeCnt_s) -> bus_creator/649
  outpmodule/650(VOUTP_SilentChkAllowSleep_flg) -> bus_creator/650
  bus_selector4/60 -> outpmodule/417(VDDM_DiagFLTSDTC_raw32)  "<VDDM_DiagFLTSDTC_raw32>"
  outpmodule/883(VOUTP_RVentEN_flg) -> bus_creator/883
  outpmodule/884(VOUTP_CRVentEN_flg) -> bus_creator/884
  bus_selector10/40 -> outpmodule/660(VPMM_CtrlFrEDUINVERTER_flg)  "<VPMM_CtrlFrEDUINVERTER_flg>"
  bus_selector2/30 -> outpmodule/33(VAPM_USSStaRCR_flg)  "<VAPM_USSStaRCR_flg>"
  outpmodule/868(VOUTP_FDCTHCCREVentYStaSet5_enum) -> bus_creator/868
  outpmodule/864(VOUTP_FDCTHCCREVentYStaSet1_enum) -> bus_creator/864
  outpmodule/862(VOUTP_FDCTHCREVentYStaSet5_enum) -> bus_creator/862
  outpmodule/858(VOUTP_FDCTHCREVentYStaSet1_enum) -> bus_creator/858
  bus_selector14/58 -> outpmodule/1042(VTQD_SlideRegenLimTq_Nm)  "<VTQD_SlideRegenLimTq_Nm>"
  outpmodule/854(VOUTP_FDCTHCCLEVentYStaSet3_enum) -> bus_creator/854
  outpmodule/855(VOUTP_FDCTHCCLEVentYStaSet4_enum) -> bus_creator/855
  outpmodule/852(VOUTP_FDCTHCCLEVentYStaSet1_enum) -> bus_creator/852
  outpmodule/723(VOUTP_FDAGSCmd_enum) -> bus_creator/723
  bus_selector13/71 -> outpmodule/958(VTPM_RFPind_enum)  "<VTPM_RFPind_enum>"
  outpmodule/721(VOUTP_FDFrWPTCHeatPwrCmd_W) -> bus_creator/721
  outpmodule/717(VOUTP_FDEXV2Cmd_step) -> bus_creator/717
  outpmodule/715(VOUTP_FDSOV3Cmd_flg) -> bus_creator/715
  outpmodule/713(VOUTP_FDSOV1Cmd_flg) -> bus_creator/713
  bus_selector2/146 -> outpmodule/149(VAPM_IVIScreen_enum)  "<VAPM_IVIScreen_enum>"
  outpmodule/226(VOUTP_AmbLightBreath1_enum) -> bus_creator/226
  outpmodule/712(VOUTP_FDCompCmd_rpm) -> bus_creator/712
  outpmodule/710(VOUTP_Var4_cnt) -> bus_creator/710
  outpmodule/709(VOUTP_ModelYear_cnt) -> bus_creator/709
  outpmodule/706(VOUTP_ECUGen2_cnt) -> bus_creator/706
  outpmodule/702(VOUTP_WisrBootReason_raw32) -> bus_creator/702
  outpmodule/691(VOUTP_SHA2_cnt) -> bus_creator/691
  bus_selector4/112 -> outpmodule/469(VDDM_RFBatwarnDTC_raw32)  "<VDDM_RFBatwarnDTC_raw32>"
  bus_selector13/74 -> outpmodule/961(VTPM_WriteChkLFID_raw)  "<VTPM_WriteChkLFID_raw>"
  bus_selector3/91 -> outpmodule/269(VBCM_ATCtrl_enum)  "<VBCM_ATCtrl_enum>"
  outpmodule/165(VOUTP_CAASSta_enum) -> bus_creator/165
  outpmodule/948(VOUTP_ID1messageALTU_raw8) -> bus_creator/948
  outpmodule/728(VOUTP_FDFrRiAPTCHeatPwrCmd_W) -> bus_creator/728
  outpmodule/8(VOUTP_ChrgPlugSta_enum) -> bus_creator/8
  outpmodule/729(VOUTP_FDRrAPTCHeatPwrCmd_W) -> bus_creator/729
  outpmodule/1072(VOUTP_FrontRearSlipRatioCtrl_flg) -> bus_creator/1072
  outpmodule/718(VOUTP_FDSOTXVCmd_flg) -> bus_creator/718
  outpmodule/316(VOUTP_WelcomeLight_enum) -> bus_creator/316
  outpmodule/1034(VOUTP_SpdCtrlSta_flg) -> bus_creator/1034
  outpmodule/314(VOUTP_FollowMeENFunSta_flg) -> bus_creator/314
  outpmodule/312(VOUTP_WalkOutLkENFunSta_flg) -> bus_creator/312
  outpmodule/308(VOUTP_RmLpModeENMem_enum) -> bus_creator/308
  outpmodule/306(VOUTP_WalkInUnLkENMem_enum) -> bus_creator/306
  outpmodule/74(VOUTP_RFPulseCountVTimeOut_flg) -> bus_creator/74
  outpmodule/592(VOUTP_UWB3Distance_enum) -> bus_creator/592
  bus_selector6/1 -> outpmodule/526(VDID_VSS_kph)  "<VDID_VSS_kph>"
  outpmodule/304(VOUTP_FDHandleCmd_enum) -> bus_creator/304
  outpmodule/301(VOUTP_TurnSwTimeSetSta457_enum) -> bus_creator/301
  outpmodule/299(VOUTP_OutMode_enum) -> bus_creator/299
  outpmodule/298(VOUTP_SPTGENFunMem_enum) -> bus_creator/298
  outpmodule/297(VOUTP_SPTGENFun_flg) -> bus_creator/297
  outpmodule/296(VOUTP_TurnSwTSetSta_enum) -> bus_creator/296
  outpmodule/213(VOUTP_BCMBuzzerReq_flg) -> bus_creator/213
  bus_selector13/59 -> outpmodule/946(VTPM_S3WheelDebugALTU_pct)  "<VTPM_S3WheelDebugALTU_pct>"
  outpmodule/285(VOUTP_AmbBrightnessSta2_enum) -> bus_creator/285
  outpmodule/685(VOUTP_Variation_cnt) -> bus_creator/685
  bus_selector17/84 -> outpmodule/1143(VVMC_FCMLDWRequest_enum)  "<VVMC_FCMLDWRequest_enum>"
  outpmodule/684(VOUTP_Country2_cnt) -> bus_creator/684
  outpmodule/682(VOUTP_Patch2_cnt) -> bus_creator/682
  bus_selector4/100 -> outpmodule/457(VDDM_MCUR1CSErrDTC_raw32)  "<VDDM_MCUR1CSErrDTC_raw32>"
  outpmodule/683(VOUTP_Country1_cnt) -> bus_creator/683
  bus_selector2/79 -> outpmodule/82(VAPM_RFPulseCountTimeOut_flg)  "<VAPM_RFPulseCountTimeOut_flg>"
  outpmodule/725(VOUTP_FDEWP2Cmd_enum) -> bus_creator/725
  outpmodule/679(VOUTP_Minor1_cnt) -> bus_creator/679
  outpmodule/922(VOUTP_RRWheelPSW_raw8) -> bus_creator/922
  outpmodule/677(VOUTP_Major1_cnt) -> bus_creator/677
  outpmodule/675(VOUTP_ECU1_cnt) -> bus_creator/675
  bus_selector4/69 -> outpmodule/426(VDDM_RMLUSSDTC_raw32)  "<VDDM_RMLUSSDTC_raw32>"
  bus_selector2/92 -> outpmodule/95(VAPM_SASSpeed_degps)  "<VAPM_SASSpeed_degps>"
  outpmodule/676(VOUTP_ECU2_cnt) -> bus_creator/676
  outpmodule/672(VOUTP_CarModel1_cnt) -> bus_creator/672
  outpmodule/671(VOUTP_HWVer3_cnt) -> bus_creator/671
  outpmodule/668(VOUTP_PwrReqRAPSAvail_flg) -> bus_creator/668
  outpmodule/667(VOUTP_OTAPwrReqStdChkSta_enum) -> bus_creator/667
  outpmodule/286(VOUTP_AmbBrightnessSta3_enum) -> bus_creator/286
  outpmodule/663(VOUTP_PwrStaTOSta_enum) -> bus_creator/663
  outpmodule/662(VOUTP_CtrlDrPwrStbA2_flg) -> bus_creator/662
  outpmodule/661(VOUTP_HWResetSta_enum) -> bus_creator/661
  outpmodule/658(VOUTP_CtrlFrRC1_flg) -> bus_creator/658
  outpmodule/656(VOUTP_LVSilentChrgLv_enum) -> bus_creator/656
  outpmodule/657(VOUTP_CtrlFrPwrStbA1P_flg) -> bus_creator/657
  bus_selector10/23 -> outpmodule/643(VPMM_LowSOCWarn_enum)  "<VPMM_LowSOCWarn_enum>"
  outpmodule/653(VOUTP_PMMAllowECUSleep_flg) -> bus_creator/653
  outpmodule/1132(VOUTP_LVDAMuteSta_enum) -> bus_creator/1132
  outpmodule/808(VOUTP_AirIntenZone3MSet7_enum) -> bus_creator/808
  outpmodule/807(VOUTP_AirIntenZone3MSet5_enum) -> bus_creator/807
  outpmodule/803(VOUTP_AirIntenZone3MSet1_enum) -> bus_creator/803
  outpmodule/805(VOUTP_AirIntenZone3MSet3_enum) -> bus_creator/805
  bus_selector13/63 -> outpmodule/950(VTPM_ID3messageALTU_raw8)  "<VTPM_ID3messageALTU_raw8>"
  bus_selector3/101 -> outpmodule/279(VBCM_AmbColorSta2_enum)  "<VBCM_AmbColorSta2_enum>"
  outpmodule/802(VOUTP_AirIntenZone1MSet7_enum) -> bus_creator/802
  outpmodule/798(VOUTP_AirIntenZone1MSet2_enum) -> bus_creator/798
  outpmodule/800(VOUTP_AirIntenZone1MSet4_enum) -> bus_creator/800
  bus_selector13/15 -> outpmodule/902(VTPM_LRSensorFail_flg)  "<VTPM_LRSensorFail_flg>"
  outpmodule/193(VOUTP_RrChargingDoorCtrl_enum) -> bus_creator/193
  outpmodule/799(VOUTP_AirIntenZone1MSet3_enum) -> bus_creator/799
  outpmodule/926(VOUTP_RFSensorMode_flg) -> bus_creator/926
  outpmodule/796(VOUTP_RecyAutoSet_enum) -> bus_creator/796
  outpmodule/795(VOUTP_sigRecircStSet_enum) -> bus_creator/795
  outpmodule/794(VOUTP_CCUSyncStsSet_enum) -> bus_creator/794
  outpmodule/793(VOUTP_fdefogSet_enum) -> bus_creator/793
  outpmodule/980(VOUTP_TPMSTLCmd_flg) -> bus_creator/980
  outpmodule/791(VOUTP_FaceMSet_enum) -> bus_creator/791
  outpmodule/867(VOUTP_FDCTHCCREVentYStaSet4_enum) -> bus_creator/867
  outpmodule/441(VOUTP_FCM5NoComDTC_raw32) -> bus_creator/441
  outpmodule/792(VOUTP_FootMSet_enum) -> bus_creator/792
  outpmodule/789(VOUTP_EWPBUflag2_flg) -> bus_creator/789
  outpmodule/788(VOUTP_EWPBUflag1_flg) -> bus_creator/788
  outpmodule/785(VOUTP_FDCFGSIONSWSta_flg) -> bus_creator/785
  outpmodule/784(VOUTP_FDCFGSChCmd_enum) -> bus_creator/784
  outpmodule/1091(VOUTP_ADASAEBReq_enum) -> bus_creator/1091
  bus_selector13/67 -> outpmodule/954(VTPM_TPMSStorge_flg)  "<VTPM_TPMSStorge_flg>"
  outpmodule/781(VOUTP_FDCFGSChSta_enum) -> bus_creator/781
  outpmodule/870(VOUTP_SettempZon1Set1_enum) -> bus_creator/870
  outpmodule/779(VOUTP_FDCTHCMAPTCForceOFFSta_flg) -> bus_creator/779
  outpmodule/777(VOUTP_FDCTHCCREVentYSta_enum) -> bus_creator/777
  bus_selector12/174 -> outpmodule/885(VTHC_FDCFGSLearnCmd_enum)  "<VTHC_FDCFGSLearnCmd_enum>"
  outpmodule/778(VOUTP_FDCTHCCRVentENSta_flg) -> bus_creator/778
  bus_selector3/82 -> outpmodule/260(VBCM_AmbFunEN_flg)  "<VBCM_AmbFunEN_flg>"
  outpmodule/775(VOUTP_FDCTHCREVentYSta_enum) -> bus_creator/775
  bus_selector17/98 -> outpmodule/1157(VVMC_CCMSASpdWar_flg)  "<VVMC_CCMSASpdWar_flg>"
  outpmodule/773(VOUTP_FDCTHCCLEVentYSta_enum) -> bus_creator/773
  bus_selector2/94 -> outpmodule/97(VAPM_SASSpeedValid_flg)  "<VAPM_SASSpeedValid_flg>"
  outpmodule/168(VOUTP_PUIDLowPower_flg) -> bus_creator/168
  bus_selector2/42 -> outpmodule/45(VAPM_BrkPedalPos_pct)  "<VAPM_BrkPedalPos_pct>"
  outpmodule/772(VOUTP_FDCTHCLVentENSta_flg) -> bus_creator/772
  outpmodule/151(VOUTP_ABSActive_flg) -> bus_creator/151
  outpmodule/150(VOUTP_IVIScreenTimeOut_flg) -> bus_creator/150
  outpmodule/148(VOUTP_CAASSwTimeOut_flg) -> bus_creator/148
  outpmodule/145(VOUTP_IVIStatus_flg) -> bus_creator/145
  outpmodule/603(VOUTP_FDCDKCAllowSleep_flg) -> bus_creator/603
  outpmodule/1151(VOUTP_APSActive_flg) -> bus_creator/1151
  outpmodule/943(VOUTP_IDin_raw32) -> bus_creator/943
  outpmodule/146(VOUTP_IVIStatusTimeOut_flg) -> bus_creator/146
  outpmodule/143(VOUTP_AVMErrSTA_flg) -> bus_creator/143
  outpmodule/1177(VOUTP_DMSModeCmd_enum) -> bus_creator/1177
  outpmodule/144(VOUTP_AVMErrSTATimeOut_flg) -> bus_creator/144
  bus_selector2/114 -> outpmodule/117(VAPM_LongAccelV_flg)  "<VAPM_LongAccelV_flg>"
  outpmodule/140(VOUTP_AVMparkingexcuteTimeOut_flg) -> bus_creator/140
  outpmodule/1117(VOUTP_ADASWarningMsg_enum) -> bus_creator/1117
  outpmodule/135(VOUTP_EPBSta_enum) -> bus_creator/135
  outpmodule/133(VOUTP_EPBErrSta_enum) -> bus_creator/133
  outpmodule/132(VOUTP_EPBExtApplyAvailTimeOut_flg) -> bus_creator/132
  outpmodule/131(VOUTP_EPBExtApplyAvail_flg) -> bus_creator/131
  outpmodule/130(VOUTP_EPBExtReleaseAvailTimeOut_flg) -> bus_creator/130
  outpmodule/129(VOUTP_EPBExtReleaseAvail_flg) -> bus_creator/129
  outpmodule/127(VOUTP_ESCAPSSta_enum) -> bus_creator/127
  outpmodule/102(VOUTP_SASVTimeOut_flg) -> bus_creator/102
  outpmodule/1095(VOUTP_ADASDBSReq_enum) -> bus_creator/1095
  outpmodule/99(VOUTP_SASCAL_flg) -> bus_creator/99
  outpmodule/97(VOUTP_SASSpeedValid_flg) -> bus_creator/97
  outpmodule/98(VOUTP_SASSpeedValidTimeOut_flg) -> bus_creator/98
  outpmodule/95(VOUTP_SASSpeed_degps) -> bus_creator/95
  outpmodule/390(VOUTP_DCDCDisDTC_raw32) -> bus_creator/390
  outpmodule/908(VOUTP_TPMSResButtAllow_flg) -> bus_creator/908
  outpmodule/153(VOUTP_TCSActive_flg) -> bus_creator/153
  outpmodule/154(VOUTP_TCSActiveTimeOut_flg) -> bus_creator/154
  outpmodule/850(VOUTP_FDCTHCLEVentYStaSet5_enum) -> bus_creator/850
  bus_selector4/125 -> outpmodule/482(VDDM_LRSensorFailDTC_raw32)  "<VDDM_LRSensorFailDTC_raw32>"
  outpmodule/121(VOUTP_BrkSwSta_flg) -> bus_creator/121
  outpmodule/698(VOUTP_NvWriteReqRisingEdge_flg) -> bus_creator/698
  bus_selector17/8 -> outpmodule/1067(VVMC_VMCMSACtrlAvail_flg)  "<VVMC_VMCMSACtrlAvail_flg>"
  outpmodule/119(VOUTP_MCPressureV_bar) -> bus_creator/119
  outpmodule/118(VOUTP_LongAccelVTimeOut_flg) -> bus_creator/118
  outpmodule/578(VOUTP_UIDLowPowerSta_flg) -> bus_creator/578
  bus_selector6/14 -> outpmodule/539(VDID_CPSAL_sec)  "<VDID_CPSAL_sec>"
  outpmodule/117(VOUTP_LongAccelV_flg) -> bus_creator/117
  outpmodule/1080(VOUTP_ISODecLimit_mps2) -> bus_creator/1080
  bus_selector13/28 -> outpmodule/915(VTPM_LFWheelTmpIndi_flg)  "<VTPM_LFWheelTmpIndi_flg>"
  outpmodule/116(VOUTP_LatAccelVTimeOut_flg) -> bus_creator/116
  outpmodule/114(VOUTP_YawRateVTimeOut_flg) -> bus_creator/114
  outpmodule/694(VOUTP_SHA5_cnt) -> bus_creator/694
  outpmodule/282(VOUTP_AmbColorSta5_enum) -> bus_creator/282
  outpmodule/111(VOUTP_MCPressure_bar) -> bus_creator/111
  bus_selector4/50 -> outpmodule/407(VDDM_APS2SigOoRDTC_raw32)  "<VDDM_APS2SigOoRDTC_raw32>"
  outpmodule/112(VOUTP_MCPressureTimeOut_flg) -> bus_creator/112
  bus_selector7/2 -> outpmodule/556(VDKC_DKCAuthSta_enum)  "<VDKC_DKCAuthSta_enum>"
  outpmodule/110(VOUTP_LongAccelTimeOut_flg) -> bus_creator/110
  outpmodule/708(VOUTP_DrivingMode_cnt) -> bus_creator/708
  outpmodule/106(VOUTP_YawRateTimeOut_flg) -> bus_creator/106
  outpmodule/105(VOUTP_YawRate_degps) -> bus_creator/105
  outpmodule/92(VOUTP_EPSAOIControlTimeOut_flg) -> bus_creator/92
  outpmodule/462(VOUTP_ESC1RCErrDTC_raw32) -> bus_creator/462
  outpmodule/89(VOUTP_DriIntend_enum) -> bus_creator/89
  outpmodule/701(VOUTP_PmicBootReason_enum) -> bus_creator/701
  outpmodule/1162(VOUTP_ExtraMSACtrlSta_enum) -> bus_creator/1162
  outpmodule/91(VOUTP_EPSAOIControl_enum) -> bus_creator/91
  outpmodule/889(VOUTP_RFBatWarn_flg) -> bus_creator/889
  outpmodule/1159(VOUTP_ActStESCYaw_Dps) -> bus_creator/1159
  bus_selector10/28 -> outpmodule/648(VPMM_LVChrgHoldTtimer_s)  "<VPMM_LVChrgHoldTtimer_s>"
  outpmodule/85(VOUTP_RRPulseCount_enum) -> bus_creator/85
  outpmodule/84(VOUTP_LRPulseCountTimeOut_flg) -> bus_creator/84
  outpmodule/606(VOUTP_DISCTargetSpd_kph) -> bus_creator/606
  outpmodule/82(VOUTP_RFPulseCountTimeOut_flg) -> bus_creator/82
  outpmodule/660(VOUTP_CtrlFrEDUINVERTER_flg) -> bus_creator/660
  outpmodule/77(VOUTP_RRPulseCountV_flg) -> bus_creator/77
  outpmodule/75(VOUTP_LRPulseCountV_flg) -> bus_creator/75
  outpmodule/76(VOUTP_LRPulseCountVTimeOut_flg) -> bus_creator/76
  outpmodule/819(VOUTP_LEVentModeStaSet457_enum) -> bus_creator/819
  outpmodule/123(VOUTP_BrkSwV_flg) -> bus_creator/123
  outpmodule/417(VOUTP_DiagFLTSDTC_raw32) -> bus_creator/417
  bus_selector2/28 -> outpmodule/31(VAPM_USSStaRLR_flg)  "<VAPM_USSStaRLR_flg>"
  bus_selector4/34 -> outpmodule/391(VDDM_HVRlyOpDTC_raw32)  "<VDDM_HVRlyOpDTC_raw32>"
  bus_selector2/23 -> outpmodule/26(VAPM_PASAFMR_enum)  "<VAPM_PASAFMR_enum>"
  bus_selector4/32 -> outpmodule/389(VDDM_MCUDisDTC_raw32)  "<VDDM_MCUDisDTC_raw32>"
  outpmodule/362(VOUTP_C3BMS1CSDTC_raw32) -> bus_creator/362
  bus_selector4/26 -> outpmodule/383(VDDM_DCDC4PreDTC_raw32)  "<VDDM_DCDC4PreDTC_raw32>"
  bus_selector4/22 -> outpmodule/379(VDDM_KeyAuthDTC_raw32)  "<VDDM_KeyAuthDTC_raw32>"
  outpmodule/669(VOUTP_HWVer1_cnt) -> bus_creator/669
  bus_selector4/20 -> outpmodule/377(VDDM_BrkSWErrDTC_raw32)  "<VDDM_BrkSWErrDTC_raw32>"
  bus_selector4/16 -> outpmodule/373(VDDM_Lv1ErrDTC_raw32)  "<VDDM_Lv1ErrDTC_raw32>"
  bus_selector4/17 -> outpmodule/374(VDDM_Lv2ErrDTC_raw32)  "<VDDM_Lv2ErrDTC_raw32>"
  outpmodule/125(VOUTP_ESCStandstill_flg) -> bus_creator/125
  bus_selector10/19 -> outpmodule/639(VPMM_PwrStaConstraint_enum)  "<VPMM_PwrStaConstraint_enum>"
  outpmodule/59(VOUTP_LRRawWhlSpeedV_flg) -> bus_creator/59
  bus_selector4/13 -> outpmodule/370(VDDM_C1ABM1RCDTC_raw32)  "<VDDM_C1ABM1RCDTC_raw32>"
  outpmodule/473(VOUTP_RFPressIndiDTC_raw32) -> bus_creator/473
  outpmodule/1145(VOUTP_ACCCtrlAvail_flg) -> bus_creator/1145
  outpmodule/186(VOUTP_TailgateSW_flg) -> bus_creator/186
  bus_selector4/12 -> outpmodule/369(VDDM_C3CCU2LCDTC_raw32)  "<VDDM_C3CCU2LCDTC_raw32>"
  bus_selector1/3 -> outpmodule/3(VACC_VehHVPwrAvail4THCM_W)  "<VACC_VehHVPwrAvail4THCM_W>"
  bus_selector1/2 -> outpmodule/2(VACC_LVBattVoltSta_enum)  "<VACC_LVBattVoltSta_enum>"
  outpmodule/968(VOUTP_WriteChkfinRRID_raw) -> bus_creator/968
  outpmodule/875(VOUTP_SettempZon1Set7_enum) -> bus_creator/875
  outpmodule/1152(VOUTP_APSStaSys_enum) -> bus_creator/1152
  outpmodule/107(VOUTP_LatAccel_Gps) -> bus_creator/107
  outpmodule/564(VOUTP_DkeyAreaRAPSSta_enum) -> bus_creator/564
  outpmodule/139(VOUTP_AVMparkingexcute_enum) -> bus_creator/139
  bus_selector4/110 -> outpmodule/467(VDDM_RrMCUTqErrDTC_raw32)  "<VDDM_RrMCUTqErrDTC_raw32>"
  outpmodule/562(VOUTP_KeyNumSta_enum) -> bus_creator/562
  bus_selector13/38 -> outpmodule/925(VTPM_LFSensorMode_flg)  "<VTPM_LFSensorMode_flg>"
  outpmodule/560(VOUTP_KeyMissSta_flg) -> bus_creator/560
  bus_selector10/39 -> outpmodule/659(VPMM_CtrlFrBMSCCUCIR_flg)  "<VPMM_CtrlFrBMSCCUCIR_flg>"
  bus_selector14/50 -> outpmodule/1034(VTQD_SpdCtrlSta_flg)  "<VTQD_SpdCtrlSta_flg>"
  outpmodule/561(VOUTP_ShippingMode_flg) -> bus_creator/561
  bus_selector2/162 -> outpmodule/165(VAPM_CAASSta_enum)  "<VAPM_CAASSta_enum>"
  bus_selector4/45 -> outpmodule/402(VDDM_HoodSWDTC_raw32)  "<VDDM_HoodSWDTC_raw32>"
  outpmodule/557(VOUTP_TimeSNDKCFbk_cnt) -> bus_creator/557
  bus_selector7/3 -> outpmodule/557(VDKC_TimeSNDKCFbk_cnt)  "<VDKC_TimeSNDKCFbk_cnt>"
  outpmodule/558(VOUTP_PCommandToBCM_enum) -> bus_creator/558
  outpmodule/553(VOUTP_DIDModelVersion_raw) -> bus_creator/553
  outpmodule/554(VOUTP_DIDModelVersionChksum_raw) -> bus_creator/554
  bus_selector10/8 -> outpmodule/628(VPMM_HVBatCnctReq_flg)  "<VPMM_HVBatCnctReq_flg>"
  outpmodule/548(VOUTP_CALID_cnt) -> bus_creator/548
  outpmodule/879(VOUTP_FOOTSet_enum) -> bus_creator/879
  bus_selector2/157 -> outpmodule/160(VAPM_APSHWVer_enum)  "<VAPM_APSHWVer_enum>"
  bus_selector4/67 -> outpmodule/424(VDDM_FCRUSSDTC_raw32)  "<VDDM_FCRUSSDTC_raw32>"
  bus_selector4/54 -> outpmodule/411(VDDM_Shifter1NoComDTC_raw32)  "<VDDM_Shifter1NoComDTC_raw32>"
  outpmodule/545(VOUTP_QTYPSATRIPSR_cnt) -> bus_creator/545
  outpmodule/103(VOUTP_GRADE_Deg) -> bus_creator/103
  bus_selector2/61 -> outpmodule/64(VAPM_LFWhlRotDirTimeOut_flg)  "<VAPM_LFWhlRotDirTimeOut_flg>"
  outpmodule/540(VOUTP_PKER_kphsqr) -> bus_creator/540
  outpmodule/174(VOUTP_RAPSBCMLockReq_flg) -> bus_creator/174
  outpmodule/539(VOUTP_CPSAL_sec) -> bus_creator/539
  outpmodule/536(VOUTP_IPSAR_sec) -> bus_creator/536
  outpmodule/535(VOUTP_PSAL_sec) -> bus_creator/535
  outpmodule/147(VOUTP_CAASSw_enum) -> bus_creator/147
  outpmodule/533(VOUTP_NUMPSATRIPSFLTMEMCLR_cnt) -> bus_creator/533
  outpmodule/559(VOUTP_KeyAreaLockUnlock_enum) -> bus_creator/559
  outpmodule/1037(VOUTP_RegenLimIndSta_flg) -> bus_creator/1037
  outpmodule/1155(VOUTP_APSReq_enum) -> bus_creator/1155
  outpmodule/532(VOUTP_ODOMETER_km) -> bus_creator/532
  outpmodule/570(VOUTP_UWB3Invalid_flg) -> bus_creator/570
  bus_selector3/146 -> outpmodule/324(VBCM_PTGUserHeight7_cnt)  "<VBCM_PTGUserHeight7_cnt>"
  bus_selector13/75 -> outpmodule/962(VTPM_WriteChkRFID_raw)  "<VTPM_WriteChkRFID_raw>"
  bus_selector3/145 -> outpmodule/323(VBCM_PTGUserHeight5_cnt)  "<VBCM_PTGUserHeight5_cnt>"
  bus_selector10/22 -> outpmodule/642(VPMM_PwrDownReq_enum)  "<VPMM_PwrDownReq_enum>"
  bus_selector3/141 -> outpmodule/319(VBCM_PTGUserHeight1_cnt)  "<VBCM_PTGUserHeight1_cnt>"
  outpmodule/838(VOUTP_FDCTHCREVentZStaSet5_enum) -> bus_creator/838
  bus_selector3/139 -> outpmodule/317(VBCM_PTGOpenHeightSta_enum)  "<VBCM_PTGOpenHeightSta_enum>"
  bus_selector17/13 -> outpmodule/1072(VVMC_FrontRearSlipRatioCtrl_flg)  "<VVMC_FrontRearSlipRatioCtrl_flg>"
  outpmodule/569(VOUTP_UWBOnOff_flg) -> bus_creator/569
  bus_selector4/62 -> outpmodule/419(VDDM_DiagRLTSDTC_raw32)  "<VDDM_DiagRLTSDTC_raw32>"
  bus_selector3/137 -> outpmodule/315(VBCM_HoodRelCmd_flg)  "<VBCM_HoodRelCmd_flg>"
  bus_selector13/80 -> outpmodule/967(VTPM_WriteChkfinLRID_raw)  "<VTPM_WriteChkfinLRID_raw>"
  outpmodule/230(VOUTP_AmbLightBreath5_enum) -> bus_creator/230
  bus_selector3/25 -> outpmodule/203(VBCM_RrFogLamp_flg)  "<VBCM_RrFogLamp_flg>"
  bus_selector4/33 -> outpmodule/390(VDDM_DCDCDisDTC_raw32)  "<VDDM_DCDCDisDTC_raw32>"
  bus_selector3/133 -> outpmodule/311(VBCM_WalkInUnLkENFunSta_flg)  "<VBCM_WalkInUnLkENFunSta_flg>"
  bus_selector3/136 -> outpmodule/314(VBCM_FollowMeENFunSta_flg)  "<VBCM_FollowMeENFunSta_flg>"
  outpmodule/806(VOUTP_AirIntenZone3MSet4_enum) -> bus_creator/806
  BDDM_outputs/1 -> bus_selector4/1
  bus_selector4/159 -> outpmodule/516(VDDM_RegenErrDTC_raw32)  "<VDDM_RegenErrDTC_raw32>"
  bus_selector4/158 -> outpmodule/515(VDDM_FrMCUActDTC_raw32)  "<VDDM_FrMCUActDTC_raw32>"
  outpmodule/465(VOUTP_ESC5CSErrDTC_raw32) -> bus_creator/465
  bus_selector4/157 -> outpmodule/514(VDDM_FrMCUDisDTC_raw32)  "<VDDM_FrMCUDisDTC_raw32>"
  bus_selector4/154 -> outpmodule/511(VDDM_CAN5BusErrorDTC_raw32)  "<VDDM_CAN5BusErrorDTC_raw32>"
  bus_selector4/155 -> outpmodule/512(VDDM_CAN6BusErrorDTC_raw32)  "<VDDM_CAN6BusErrorDTC_raw32>"
  bus_selector3/135 -> outpmodule/313(VBCM_RmLpModeENFunSta_flg)  "<VBCM_RmLpModeENFunSta_flg>"
  outpmodule/612(VOUTP_CSB_flg) -> bus_creator/612
  BTQR_outputs/1 -> bus_selector15/1
  bus_selector4/152 -> outpmodule/509(VDDM_CAN3BusErrorDTC_raw32)  "<VDDM_CAN3BusErrorDTC_raw32>"
  outpmodule/593(VOUTP_UWB4Distance_enum) -> bus_creator/593
  outpmodule/872(VOUTP_SettempZon1Set3_enum) -> bus_creator/872
  bus_selector4/149 -> outpmodule/506(VDDM_VCUTailgateSWSta_flg)  "<VDDM_VCUTailgateSWSta_flg>"
  bus_selector4/148 -> outpmodule/505(VDDM_VCUHoodSWSta_flg)  "<VDDM_VCUHoodSWSta_flg>"
  outpmodule/693(VOUTP_SHA4_cnt) -> bus_creator/693
  bus_selector4/145 -> outpmodule/502(VDDM_VCURLDoorSta_flg)  "<VDDM_VCURLDoorSta_flg>"
  outpmodule/10(VOUTP_PASDRML_cm) -> bus_creator/10
  bus_selector4/146 -> outpmodule/503(VDDM_VCURRDoorSta_flg)  "<VDDM_VCURRDoorSta_flg>"
  bus_selector4/68 -> outpmodule/425(VDDM_RCLUSSDTC_raw32)  "<VDDM_RCLUSSDTC_raw32>"
  bus_selector4/143 -> outpmodule/500(VDDM_VCUFLDoorSta_flg)  "<VDDM_VCUFLDoorSta_flg>"
  bus_selector16/1 -> outpmodule/1053(VV2L_ReqOBCV2LEna_enum)  "<VV2L_ReqOBCV2LEna_enum>"
  bus_selector4/142 -> outpmodule/499(VDDM_VCUBrkSWSta_enum)  "<VDDM_VCUBrkSWSta_enum>"
  bus_selector4/141 -> outpmodule/498(VDDM_MCUActDisFail_flg)  "<VDDM_MCUActDisFail_flg>"
  outpmodule/141(VOUTP_AVMParkingmode_enum) -> bus_creator/141
  outpmodule/501(VOUTP_VCUFRDoorSta_flg) -> bus_creator/501
  bus_selector4/136 -> outpmodule/493(VDDM_VCURAPSErrLv2_flg)  "<VDDM_VCURAPSErrLv2_flg>"
  bus_selector2/143 -> outpmodule/146(VAPM_IVIStatusTimeOut_flg)  "<VAPM_IVIStatusTimeOut_flg>"
  outpmodule/711(VOUTP_Var5_cnt) -> bus_creator/711
  bus_selector4/139 -> outpmodule/496(VDDM_LVSysErrPwrOutErr_flg)  "<VDDM_LVSysErrPwrOutErr_flg>"
  bus_selector4/135 -> outpmodule/492(VDDM_DisengagePFail_flg)  "<VDDM_DisengagePFail_flg>"
  outpmodule/719(VOUTP_FDFWVCmd_flg) -> bus_creator/719
  bus_selector4/31 -> outpmodule/388(VDDM_MidLvSaChkDTC_raw32)  "<VDDM_MidLvSaChkDTC_raw32>"
  bus_selector2/58 -> outpmodule/61(VAPM_RRRawWhlSpeedV_flg)  "<VAPM_RRRawWhlSpeedV_flg>"
  outpmodule/767(VOUTP_FDCTHCLEVentZSta_enum) -> bus_creator/767
  outpmodule/720(VOUTP_FDTWVCmd_pct) -> bus_creator/720
  outpmodule/423(VOUTP_FMRUSSDTC_raw32) -> bus_creator/423
  outpmodule/768(VOUTP_FDCTHCCLEVentZSta_enum) -> bus_creator/768
  bus_selector10/32 -> outpmodule/652(VPMM_FDADC12VDetAvg_mV)  "<VPMM_FDADC12VDetAvg_mV>"
  outpmodule/384(VOUTP_HVRlyCloDTC_raw32) -> bus_creator/384
  outpmodule/766(VOUTP_FDCTHCREVentModeSta_enum) -> bus_creator/766
  outpmodule/531(VOUTP_APPE_pct) -> bus_creator/531
  bus_selector6/17 -> outpmodule/542(VDID_ResetCDEODTR_km)  "<VDID_ResetCDEODTR_km>"
  outpmodule/763(VOUTP_sigDfrstSt_flg) -> bus_creator/763
  bus_selector13/35 -> outpmodule/922(VTPM_RRWheelPSW_raw8)  "<VTPM_RRWheelPSW_raw8>"
  outpmodule/765(VOUTP_FDCTHCLEVentModeSta_enum) -> bus_creator/765
  bus_selector4/150 -> outpmodule/507(VDDM_CAN1BusErrorDTC_raw32)  "<VDDM_CAN1BusErrorDTC_raw32>"
  outpmodule/526(VOUTP_VSS_kph) -> bus_creator/526
  outpmodule/487(VOUTP_EPBLockTODTC_raw32) -> bus_creator/487
  outpmodule/764(VOUTP_FDCTHCAirIntZ3Sta_enum) -> bus_creator/764
  outpmodule/761(VOUTP_fdefog_flg) -> bus_creator/761
  bus_selector10/42 -> outpmodule/662(VPMM_CtrlDrPwrStbA2_flg)  "<VPMM_CtrlDrPwrStbA2_flg>"
  outpmodule/66(VOUTP_RFWhlRotDirTimeOut_flg) -> bus_creator/66
  outpmodule/762(VOUTP_sigSetTempZon2StM_C) -> bus_creator/762
  outpmodule/758(VOUTP_ACForceOFF_flg) -> bus_creator/758
  outpmodule/687(VOUTP_Change1_cnt) -> bus_creator/687
  outpmodule/759(VOUTP_RecAutoFlg_flg) -> bus_creator/759
  outpmodule/157(VOUTP_APSProgressPCT_pct) -> bus_creator/157
  outpmodule/760(VOUTP_AirIntenZone1M_enum) -> bus_creator/760
  outpmodule/1039(VOUTP_MaxWhlSlideRate_pct) -> bus_creator/1039
  outpmodule/528(VOUTP_MILDIST_km) -> bus_creator/528
  bus_selector13/23 -> outpmodule/910(VTPM_LFPressIndi_enum)  "<VTPM_LFPressIndi_enum>"
  outpmodule/756(VOUTP_FootM_flg) -> bus_creator/756
  outpmodule/695(VOUTP_SHA6_cnt) -> bus_creator/695
  bus_selector6/10 -> outpmodule/535(VDID_PSAL_sec)  "<VDID_PSAL_sec>"
  outpmodule/466(VOUTP_FrMCUTqErrDTC_raw32) -> bus_creator/466
  outpmodule/752(VOUTP_Face_flg) -> bus_creator/752
  outpmodule/753(VOUTP_Foot_flg) -> bus_creator/753
  bus_selector17/83 -> outpmodule/1142(VVMC_ADASAEBSta_enum)  "<VVMC_ADASAEBSta_enum>"
  outpmodule/483(VOUTP_RRSensorFailDTC_raw32) -> bus_creator/483
  outpmodule/689(VOUTP_Dash2_cnt) -> bus_creator/689
  bus_selector4/55 -> outpmodule/412(VDDM_ESC7NoComDTC_raw32)  "<VDDM_ESC7NoComDTC_raw32>"
  outpmodule/750(VOUTP_FDRecyAutoCmd_enum) -> bus_creator/750
  outpmodule/749(VOUTP_ACSubMode_enum) -> bus_creator/749
  outpmodule/1069(VOUTP_FeatReqSpd_kph) -> bus_creator/1069
  outpmodule/748(VOUTP_sigCbnAirT_C) -> bus_creator/748
  outpmodule/877(VOUTP_ACModeSet457_enum) -> bus_creator/877
  outpmodule/746(VOUTP_sigCbnSolarRight_W) -> bus_creator/746
  outpmodule/745(VOUTP_sigClntTHvBattIn_C) -> bus_creator/745
  bus_selector4/144 -> outpmodule/501(VDDM_VCUFRDoorSta_flg)  "<VDDM_VCUFRDoorSta_flg>"
  outpmodule/744(VOUTP_sigCbnSolarLeft_W) -> bus_creator/744
  outpmodule/742(VOUTP_sigSetTempZon2St_C) -> bus_creator/742
  outpmodule/739(VOUTP_sigWindDirZon1St_enum) -> bus_creator/739
  outpmodule/697(VOUTP_SHA8_cnt) -> bus_creator/697
  outpmodule/489(VOUTP_LimpHomeAct_flg) -> bus_creator/489
  bus_selector13/36 -> outpmodule/923(VTPM_CWheelTips_enum)  "<VTPM_CWheelTips_enum>"
  outpmodule/737(VOUTP_CCUSyncLampSts_flg) -> bus_creator/737
  outpmodule/851(VOUTP_FDCTHCLEVentYStaSet7_enum) -> bus_creator/851
  outpmodule/735(VOUTP_CCUAutoLampSts_flg) -> bus_creator/735
  outpmodule/732(VOUTP_EDriveMode_enum) -> bus_creator/732
  bus_selector2/53 -> outpmodule/56(VAPM_LFRawWhlSpeedVTimeOut_flg)  "<VAPM_LFRawWhlSpeedVTimeOut_flg>"
  outpmodule/164(VOUTP_APSRqEPASCtrl_flg) -> bus_creator/164
  outpmodule/731(VOUTP_BatteryMode_enum) -> bus_creator/731
  outpmodule/665(VOUTP_PwrReq_OTA_enum) -> bus_creator/665
  outpmodule/769(VOUTP_FDCTHCREVentZSta_enum) -> bus_creator/769
  outpmodule/1137(VOUTP_FCMACCmode_enum) -> bus_creator/1137
  outpmodule/776(VOUTP_FDCTHCRVentENSta_flg) -> bus_creator/776
  bus_selector12/116 -> outpmodule/827(VTHC_FDCTHCLEVentZStaSet7_enum)  "<VTHC_FDCTHCLEVentZStaSet7_enum>"
  bus_selector12/120 -> outpmodule/831(VTHC_FDCTHCCLEVentZStaSet4_enum)  "<VTHC_FDCTHCCLEVentZStaSet4_enum>"
  outpmodule/681(VOUTP_Patch1_cnt) -> bus_creator/681
  outpmodule/512(VOUTP_CAN6BusErrorDTC_raw32) -> bus_creator/512
  bus_selector12/119 -> outpmodule/830(VTHC_FDCTHCCLEVentZStaSet3_enum)  "<VTHC_FDCTHCCLEVentZStaSet3_enum>"
  outpmodule/743(VOUTP_sigClntTHvBattOut_C) -> bus_creator/743
  bus_selector3/108 -> outpmodule/286(VBCM_AmbBrightnessSta3_enum)  "<VBCM_AmbBrightnessSta3_enum>"
  outpmodule/741(VOUTP_sigSetTempZon1St_C) -> bus_creator/741
  bus_selector2/2 -> outpmodule/5(VAPM_VehSpeedTimeOut_flg)  "<VAPM_VehSpeedTimeOut_flg>"
  bus_selector12/117 -> outpmodule/828(VTHC_FDCTHCCLEVentZStaSet1_enum)  "<VTHC_FDCTHCCLEVentZStaSet1_enum>"
  bus_selector12/118 -> outpmodule/829(VTHC_FDCTHCCLEVentZStaSet2_enum)  "<VTHC_FDCTHCCLEVentZStaSet2_enum>"
  bus_selector2/123 -> outpmodule/126(VAPM_ESCStandstillTimeOut_flg)  "<VAPM_ESCStandstillTimeOut_flg>"
  outpmodule/172(VOUTP_APSVMCReqA_flg) -> bus_creator/172
  bus_selector12/114 -> outpmodule/825(VTHC_FDCTHCLEVentZStaSet4_enum)  "<VTHC_FDCTHCLEVentZStaSet4_enum>"
  bus_selector12/110 -> outpmodule/821(VTHC_REVentModeStaSet457_enum)  "<VTHC_REVentModeStaSet457_enum>"
  bus_selector12/113 -> outpmodule/824(VTHC_FDCTHCLEVentZStaSet3_enum)  "<VTHC_FDCTHCLEVentZStaSet3_enum>"
  bus_selector12/107 -> outpmodule/818(VTHC_LEVentModeStaSet123_enum)  "<VTHC_LEVentModeStaSet123_enum>"
  outpmodule/861(VOUTP_FDCTHCREVentYStaSet4_enum) -> bus_creator/861
  bus_selector12/109 -> outpmodule/820(VTHC_REVentModeStaSet123_enum)  "<VTHC_REVentModeStaSet123_enum>"
  outpmodule/446(VOUTP_FrMCUSigErrDetDTC_raw32) -> bus_creator/446
  bus_selector12/104 -> outpmodule/815(VTHC_CLVentENSet_enum)  "<VTHC_CLVentENSet_enum>"
  outpmodule/203(VOUTP_RrFogLamp_flg) -> bus_creator/203
  outpmodule/1141(VOUTP_ADASLanecurveR_raw32) -> bus_creator/1141
  bus_selector12/106 -> outpmodule/817(VTHC_CRVentENSet_enum)  "<VTHC_CRVentENSet_enum>"
  bus_selector4/27 -> outpmodule/384(VDDM_HVRlyCloDTC_raw32)  "<VDDM_HVRlyCloDTC_raw32>"
  bus_selector12/95 -> outpmodule/806(VTHC_AirIntenZone3MSet4_enum)  "<VTHC_AirIntenZone3MSet4_enum>"
  bus_selector12/94 -> outpmodule/805(VTHC_AirIntenZone3MSet3_enum)  "<VTHC_AirIntenZone3MSet3_enum>"
  outpmodule/664(VOUTP_Sched_ChgTOSta_enum) -> bus_creator/664
  outpmodule/1172(VOUTP_FDCVMCAngCtrlTqWtGn_pct) -> bus_creator/1172
  bus_selector12/93 -> outpmodule/804(VTHC_AirIntenZone3MSet2_enum)  "<VTHC_AirIntenZone3MSet2_enum>"
  outpmodule/1062(VOUTP_VehicleSpeed_kph) -> bus_creator/1062
  bus_selector12/89 -> outpmodule/800(VTHC_AirIntenZone1MSet4_enum)  "<VTHC_AirIntenZone1MSet4_enum>"
  outpmodule/866(VOUTP_FDCTHCCREVentYStaSet3_enum) -> bus_creator/866
  bus_selector2/169 -> outpmodule/172(VAPM_APSVMCReqA_flg)  "<VAPM_APSVMCReqA_flg>"
  outpmodule/40(VOUTP_USSStaFCL_flg) -> bus_creator/40
  bus_selector12/92 -> outpmodule/803(VTHC_AirIntenZone3MSet1_enum)  "<VTHC_AirIntenZone3MSet1_enum>"
  outpmodule/494(VOUTP_VCURAPSErrLv3_flg) -> bus_creator/494
  outpmodule/997(VOUTP_DriverWhlTqDemFr_Nm) -> bus_creator/997
  bus_selector12/91 -> outpmodule/802(VTHC_AirIntenZone1MSet7_enum)  "<VTHC_AirIntenZone1MSet7_enum>"
  bus_selector12/87 -> outpmodule/798(VTHC_AirIntenZone1MSet2_enum)  "<VTHC_AirIntenZone1MSet2_enum>"
  outpmodule/511(VOUTP_CAN5BusErrorDTC_raw32) -> bus_creator/511
  outpmodule/678(VOUTP_Major2_cnt) -> bus_creator/678
  outpmodule/1146(VOUTP_ACCPedalOvrd_flg) -> bus_creator/1146
  bus_selector12/86 -> outpmodule/797(VTHC_AirIntenZone1MSet1_enum)  "<VTHC_AirIntenZone1MSet1_enum>"
  outpmodule/60(VOUTP_LRRawWhlSpeedVTimeOut_flg) -> bus_creator/60
  bus_selector2/170 -> outpmodule/173(VAPM_RAPSBCMLamp_enum)  "<VAPM_RAPSBCMLamp_enum>"
  bus_selector12/85 -> outpmodule/796(VTHC_RecyAutoSet_enum)  "<VTHC_RecyAutoSet_enum>"
  outpmodule/700(VOUTP_FdcSlpTime_sec) -> bus_creator/700
  outpmodule/397(VOUTP_DrStSWDTC_raw32) -> bus_creator/397
  bus_selector12/83 -> outpmodule/794(VTHC_CCUSyncStsSet_enum)  "<VTHC_CCUSyncStsSet_enum>"
  bus_selector2/57 -> outpmodule/60(VAPM_LRRawWhlSpeedVTimeOut_flg)  "<VAPM_LRRawWhlSpeedVTimeOut_flg>"
  bus_selector3/140 -> outpmodule/318(VBCM_UserHeightSet_cnt)  "<VBCM_UserHeightSet_cnt>"
  bus_selector12/84 -> outpmodule/795(VTHC_sigRecircStSet_enum)  "<VTHC_sigRecircStSet_enum>"
  bus_selector12/82 -> outpmodule/793(VTHC_fdefogSet_enum)  "<VTHC_fdefogSet_enum>"
  bus_selector12/81 -> outpmodule/792(VTHC_FootMSet_enum)  "<VTHC_FootMSet_enum>"
  outpmodule/408(VOUTP_APSCorrErrDTC_raw32) -> bus_creator/408
  bus_selector12/78 -> outpmodule/789(VTHC_EWPBUflag2_flg)  "<VTHC_EWPBUflag2_flg>"
  bus_selector13/29 -> outpmodule/916(VTPM_RFWheelTmpIndi_flg)  "<VTPM_RFWheelTmpIndi_flg>"
  outpmodule/809(VOUTP_IONSWStaSet_enum) -> bus_creator/809
  bus_selector12/77 -> outpmodule/788(VTHC_EWPBUflag1_flg)  "<VTHC_EWPBUflag1_flg>"
  bus_selector2/172 -> outpmodule/175(VAPM_APSPwrReq_enum)  "<VAPM_APSPwrReq_enum>"
  bus_selector12/79 -> outpmodule/790(VTHC_EWPBUflag3_flg)  "<VTHC_EWPBUflag3_flg>"
  outpmodule/185(VOUTP_HoodSW_flg) -> bus_creator/185
  bus_selector12/75 -> outpmodule/786(VTHC_FDCFGSIONCmd_flg)  "<VTHC_FDCFGSIONCmd_flg>"
  outpmodule/878(VOUTP_FACESet_enum) -> bus_creator/878
  outpmodule/895(VOUTP_RRWheelPress_raw8) -> bus_creator/895
  bus_selector12/76 -> outpmodule/787(VTHC_FDCTHCMPreWPTCHeatSta_enum)  "<VTHC_FDCTHCMPreWPTCHeatSta_enum>"
  bus_selector12/71 -> outpmodule/782(VTHC_FDCFGSAirIntCmd_enum)  "<VTHC_FDCFGSAirIntCmd_enum>"
  outpmodule/492(VOUTP_DisengagePFail_flg) -> bus_creator/492
  bus_selector12/73 -> outpmodule/784(VTHC_FDCFGSChCmd_enum)  "<VTHC_FDCFGSChCmd_enum>"
  bus_selector10/20 -> outpmodule/640(VPMM_TCountSta_enum)  "<VPMM_TCountSta_enum>"
  bus_selector12/74 -> outpmodule/785(VTHC_FDCFGSIONSWSta_flg)  "<VTHC_FDCFGSIONSWSta_flg>"
  bus_selector3/20 -> outpmodule/198(VBCM_Dimmer_pct)  "<VBCM_Dimmer_pct>"
  bus_selector14/49 -> outpmodule/1033(VTQD_SpdCtrlMode_enum)  "<VTQD_SpdCtrlMode_enum>"
  bus_selector3/22 -> outpmodule/200(VBCM_PosLamp_flg)  "<VBCM_PosLamp_flg>"
  bus_selector3/19 -> outpmodule/197(VBCM_CTDLockSW_flg)  "<VBCM_CTDLockSW_flg>"
  outpmodule/358(VOUTP_C3BMS6RCDTC_raw32) -> bus_creator/358
  bus_selector4/36 -> outpmodule/393(VDDM_OBC4PreDTC_raw32)  "<VDDM_OBC4PreDTC_raw32>"
  outpmodule/124(VOUTP_BrkSwVTimeOut_flg) -> bus_creator/124
  bus_selector3/15 -> outpmodule/193(VBCM_RrChargingDoorCtrl_enum)  "<VBCM_RrChargingDoorCtrl_enum>"
  bus_selector3/14 -> outpmodule/192(VBCM_FrChargingDoorCtrl_enum)  "<VBCM_FrChargingDoorCtrl_enum>"
  outpmodule/651(VOUTP_TimerAllowSleep_flg) -> bus_creator/651
  bus_selector3/12 -> outpmodule/190(VBCM_RRDoorSW_flg)  "<VBCM_RRDoorSW_flg>"
  outpmodule/584(VOUTP_A0UWBEvent_enum) -> bus_creator/584
  bus_selector3/13 -> outpmodule/191(VBCM_LockSetting_flg)  "<VBCM_LockSetting_flg>"
  bus_selector2/18 -> outpmodule/21(VAPM_PASAFCL_enum)  "<VAPM_PASAFCL_enum>"
  bus_selector3/9 -> outpmodule/187(VBCM_DrDoorSW_flg)  "<VBCM_DrDoorSW_flg>"
  outpmodule/881(VOUTP_LVentEN_flg) -> bus_creator/881
  bus_selector13/3 -> outpmodule/890(VTPM_LRBatWarn_flg)  "<VTPM_LRBatWarn_flg>"
  bus_selector4/109 -> outpmodule/466(VDDM_FrMCUTqErrDTC_raw32)  "<VDDM_FrMCUTqErrDTC_raw32>"
  outpmodule/599(VOUTP_UWB3FPP_enum) -> bus_creator/599
  bus_selector3/11 -> outpmodule/189(VBCM_RLDoorSW_flg)  "<VBCM_RLDoorSW_flg>"
  bus_selector4/52 -> outpmodule/409(VDDM_MCUF1NoComDTC_raw32)  "<VDDM_MCUF1NoComDTC_raw32>"
  outpmodule/22(VOUTP_PASARMR_enum) -> bus_creator/22
  bus_selector3/8 -> outpmodule/186(VBCM_TailgateSW_flg)  "<VBCM_TailgateSW_flg>"
  outpmodule/890(VOUTP_LRBatWarn_flg) -> bus_creator/890
  bus_selector3/4 -> outpmodule/182(VBCM_AllDoorSW_flg)  "<VBCM_AllDoorSW_flg>"
  outpmodule/906(VOUTP_RFWheelDebug_flg) -> bus_creator/906
  bus_selector3/6 -> outpmodule/184(VBCM_AntitheftSeatFlod_flg)  "<VBCM_AntitheftSeatFlod_flg>"
  outpmodule/290(VOUTP_HazardIND_flg) -> bus_creator/290
  bus_selector3/5 -> outpmodule/183(VBCM_BCMDoorLockSta_flg)  "<VBCM_BCMDoorLockSta_flg>"
  bus_selector3/1 -> outpmodule/179(VBCM_AntitheftSta_enum)  "<VBCM_AntitheftSta_enum>"
  outpmodule/1075(VOUTP_LatAccCtrl_flg) -> bus_creator/1075
  outpmodule/722(VOUTP_CoolgFanActDuty_pct) -> bus_creator/722
  outpmodule/200(VOUTP_PosLamp_flg) -> bus_creator/200
  outpmodule/263(VOUTP_AmbLinkDriSta_flg) -> bus_creator/263
  bus_selector2/166 -> outpmodule/169(VAPM_CAASVMCReqA_flg)  "<VAPM_CAASVMCReqA_flg>"
  outpmodule/236(VOUTP_AmbLightBrightness5_enum) -> bus_creator/236
  outpmodule/246(VOUTP_APSOpenPTG_flg) -> bus_creator/246
  outpmodule/680(VOUTP_Minor2_cnt) -> bus_creator/680
  outpmodule/242(VOUTP_AmbLightColor5_enum) -> bus_creator/242
  outpmodule/239(VOUTP_AmbLightColor2_enum) -> bus_creator/239
  bus_selector3/52 -> outpmodule/230(VBCM_AmbLightBreath5_enum)  "<VBCM_AmbLightBreath5_enum>"
  bus_selector3/54 -> outpmodule/232(VBCM_AmbLightBrightness1_enum)  "<VBCM_AmbLightBrightness1_enum>"
  bus_selector3/18 -> outpmodule/196(VBCM_DoorLockIND_flg)  "<VBCM_DoorLockIND_flg>"
  bus_selector3/49 -> outpmodule/227(VBCM_AmbLightBreath2_enum)  "<VBCM_AmbLightBreath2_enum>"
  outpmodule/305(VOUTP_HBeamADB_enum) -> bus_creator/305
  bus_selector3/48 -> outpmodule/226(VBCM_AmbLightBreath1_enum)  "<VBCM_AmbLightBreath1_enum>"
  outpmodule/804(VOUTP_AirIntenZone3MSet2_enum) -> bus_creator/804
  outpmodule/1084(VOUTP_FeatArbitrFinal_enum) -> bus_creator/1084
  bus_selector13/26 -> outpmodule/913(VTPM_RRPressIndi_enum)  "<VTPM_RRPressIndi_enum>"
  bus_selector3/47 -> outpmodule/225(VBCM_WiperFixMode_flg)  "<VBCM_WiperFixMode_flg>"
  outpmodule/964(VOUTP_WriteChkRRID_raw) -> bus_creator/964
  bus_selector10/43 -> outpmodule/663(VPMM_PwrStaTOSta_enum)  "<VPMM_PwrStaTOSta_enum>"
  outpmodule/241(VOUTP_AmbLightColor4_enum) -> bus_creator/241
  bus_selector3/41 -> outpmodule/219(VBCM_TrunkRel_flg)  "<VBCM_TrunkRel_flg>"
  outpmodule/152(VOUTP_ABSActiveTimeOut_flg) -> bus_creator/152
  outpmodule/1160(VOUTP_CAASCtrlAvail_flg) -> bus_creator/1160
  bus_selector3/37 -> outpmodule/215(VBCM_MirrorDefog_flg)  "<VBCM_MirrorDefog_flg>"
  bus_selector2/101 -> outpmodule/104(VAPM_GRADETimeOut_flg)  "<VAPM_GRADETimeOut_flg>"
  bus_selector3/34 -> outpmodule/212(VBCM_RTurnLP_flg)  "<VBCM_RTurnLP_flg>"
  bus_selector4/71 -> outpmodule/428(VDDM_RCRUSSDTC_raw32)  "<VDDM_RCRUSSDTC_raw32>"
  bus_selector3/31 -> outpmodule/209(VBCM_RBSD_flg)  "<VBCM_RBSD_flg>"
  bus_selector3/35 -> outpmodule/213(VBCM_BCMBuzzerReq_flg)  "<VBCM_BCMBuzzerReq_flg>"
  bus_selector3/77 -> outpmodule/255(VBCM_DrvWdwCtrlCmd_pct)  "<VBCM_DrvWdwCtrlCmd_pct>"
  bus_selector3/76 -> outpmodule/254(VBCM_PTGInnerSW2_enum)  "<VBCM_PTGInnerSW2_enum>"
  outpmodule/41(VOUTP_Chime_enum) -> bus_creator/41
  outpmodule/500(VOUTP_VCUFLDoorSta_flg) -> bus_creator/500
  bus_selector3/74 -> outpmodule/252(VBCM_FuelDoorPos_flg)  "<VBCM_FuelDoorPos_flg>"
  bus_selector3/71 -> outpmodule/249(VBCM_CountAlarm_enum)  "<VBCM_CountAlarm_enum>"
  bus_selector3/40 -> outpmodule/218(VBCM_RoomLampL_flg)  "<VBCM_RoomLampL_flg>"
  bus_selector10/12 -> outpmodule/632(VPMM_HVPwrSta_flg)  "<VPMM_HVPwrSta_flg>"
  bus_selector3/68 -> outpmodule/246(VBCM_APSOpenPTG_flg)  "<VBCM_APSOpenPTG_flg>"
  outpmodule/565(VOUTP_KeyAreaPS_enum) -> bus_creator/565
  bus_selector13/96 -> outpmodule/983(VTPM_ModelVersion_raw)  "<VTPM_ModelVersion_raw>"
  bus_selector3/65 -> outpmodule/243(VBCM_AmbLightColor6_enum)  "<VBCM_AmbLightColor6_enum>"
  bus_selector14/37 -> outpmodule/1021(VTQD_ReBrakeLPReq_flg)  "<VTQD_ReBrakeLPReq_flg>"
  outpmodule/1107(VOUTP_ADASForceIdle_flg) -> bus_creator/1107
  outpmodule/313(VOUTP_RmLpModeENFunSta_flg) -> bus_creator/313
  bus_selector13/11 -> outpmodule/898(VTPM_LRWheelTemp_C)  "<VTPM_LRWheelTemp_C>"
  bus_selector3/60 -> outpmodule/238(VBCM_AmbLightColor1_enum)  "<VBCM_AmbLightColor1_enum>"
  bus_selector13/66 -> outpmodule/953(VTPM_SetIDLoc_flg)  "<VTPM_SetIDLoc_flg>"
  outpmodule/598(VOUTP_UWB2FPP_enum) -> bus_creator/598
  bus_selector3/59 -> outpmodule/237(VBCM_AmbLightBrightness6_enum)  "<VBCM_AmbLightBrightness6_enum>"
  bus_selector3/55 -> outpmodule/233(VBCM_AmbLightBrightness2_enum)  "<VBCM_AmbLightBrightness2_enum>"
  bus_selector12/101 -> outpmodule/812(VTHC_FDCFGSAirIntStaSet123_enum)  "<VTHC_FDCFGSAirIntStaSet123_enum>"
  bus_selector12/72 -> outpmodule/783(VTHC_FDCFGSFuncSta_enum)  "<VTHC_FDCFGSFuncSta_enum>"
  outpmodule/437(VOUTP_FCM3RCErrDTC_raw32) -> bus_creator/437
  bus_selector2/99 -> outpmodule/102(VAPM_SASVTimeOut_flg)  "<VAPM_SASVTimeOut_flg>"
  outpmodule/704(VOUTP_CurrentNmState_enum) -> bus_creator/704
  bus_selector2/140 -> outpmodule/143(VAPM_AVMErrSTA_flg)  "<VAPM_AVMErrSTA_flg>"
  outpmodule/73(VOUTP_RFPulseCountV_flg) -> bus_creator/73
  outpmodule/1041(VOUTP_ForceP_flg) -> bus_creator/1041
  outpmodule/244(VOUTP_LampPwr_flg) -> bus_creator/244
  bus_selector2/90 -> outpmodule/93(VAPM_SASAngle_Deg)  "<VAPM_SASAngle_Deg>"
  outpmodule/78(VOUTP_RRPulseCountVTimeOut_flg) -> bus_creator/78
  bus_selector7/44 -> outpmodule/598(VDKC_UWB2FPP_enum)  "<VDKC_UWB2FPP_enum>"
  bus_selector3/58 -> outpmodule/236(VBCM_AmbLightBrightness5_enum)  "<VBCM_AmbLightBrightness5_enum>"
  outpmodule/865(VOUTP_FDCTHCCREVentYStaSet2_enum) -> bus_creator/865
  bus_selector12/112 -> outpmodule/823(VTHC_FDCTHCLEVentZStaSet2_enum)  "<VTHC_FDCTHCLEVentZStaSet2_enum>"
  bus_selector7/45 -> outpmodule/599(VDKC_UWB3FPP_enum)  "<VDKC_UWB3FPP_enum>"
  bus_selector7/39 -> outpmodule/593(VDKC_UWB4Distance_enum)  "<VDKC_UWB4Distance_enum>"
  bus_selector2/132 -> outpmodule/135(VAPM_EPBSta_enum)  "<VAPM_EPBSta_enum>"
  bus_selector4/140 -> outpmodule/497(VDDM_HVRlyOpFail_flg)  "<VDDM_HVRlyOpFail_flg>"
  bus_selector7/31 -> outpmodule/585(VDKC_ParkingModeCmd_enum)  "<VDKC_ParkingModeCmd_enum>"
  bus_selector10/5 -> outpmodule/625(VPMM_ActiveDischargeReq_flg)  "<VPMM_ActiveDischargeReq_flg>"
  outpmodule/206(VOUTP_LDRL_flg) -> bus_creator/206
  bus_selector7/27 -> outpmodule/581(VDKC_KeyTypeSta_enum)  "<VDKC_KeyTypeSta_enum>"
  outpmodule/456(VOUTP_MCUF1CSErrDTC_raw32) -> bus_creator/456
  bus_selector12/103 -> outpmodule/814(VTHC_LVentENSet_enum)  "<VTHC_LVentENSet_enum>"
  outpmodule/237(VOUTP_AmbLightBrightness6_enum) -> bus_creator/237
  bus_selector4/108 -> outpmodule/465(VDDM_ESC5CSErrDTC_raw32)  "<VDDM_ESC5CSErrDTC_raw32>"
  bus_selector7/21 -> outpmodule/575(VDKC_CoordinateX_enum)  "<VDKC_CoordinateX_enum>"
  outpmodule/217(VOUTP_RoomLampH_flg) -> bus_creator/217
  bus_selector2/8 -> outpmodule/11(VAPM_PASDRCR_cm)  "<VAPM_PASDRCR_cm>"
  bus_selector7/43 -> outpmodule/597(VDKC_UWB1FPP_enum)  "<VDKC_UWB1FPP_enum>"
  bus_selector7/22 -> outpmodule/576(VDKC_FDCSPTGDet_flg)  "<VDKC_FDCSPTGDet_flg>"
  bus_selector2/24 -> outpmodule/27(VAPM_PASAFML_enum)  "<VAPM_PASAFML_enum>"
  bus_selector7/16 -> outpmodule/570(VDKC_UWB3Invalid_flg)  "<VDKC_UWB3Invalid_flg>"
  BDKC_outputs/1 -> bus_selector7/1
  outpmodule/542(VOUTP_ResetCDEODTR_km) -> bus_creator/542
  bus_selector3/78 -> outpmodule/256(VBCM_PasWdwCtrlCmd_pct)  "<VBCM_PasWdwCtrlCmd_pct>"
  bus_selector7/18 -> outpmodule/572(VDKC_UWB2Invalid_flg)  "<VDKC_UWB2Invalid_flg>"
  bus_selector7/17 -> outpmodule/571(VDKC_UWB1Invalid_flg)  "<VDKC_UWB1Invalid_flg>"
  bus_selector13/40 -> outpmodule/927(VTPM_LRSensorMode_flg)  "<VTPM_LRSensorMode_flg>"
  outpmodule/277(VOUTP_AmbODAENFlash_enum) -> bus_creator/277
  bus_selector7/14 -> outpmodule/568(VDKC_UWB4Invalid_flg)  "<VDKC_UWB4Invalid_flg>"
  outpmodule/541(VOUTP_PKEL_kphsqr) -> bus_creator/541
  outpmodule/33(VOUTP_USSStaRCR_flg) -> bus_creator/33
  bus_selector7/10 -> outpmodule/564(VDKC_DkeyAreaRAPSSta_enum)  "<VDKC_DkeyAreaRAPSSta_enum>"
  outpmodule/29(VOUTP_USSStaRMR_flg) -> bus_creator/29
  bus_selector7/13 -> outpmodule/567(VDKC_KeyAreaPTG_enum)  "<VDKC_KeyAreaPTG_enum>"
  outpmodule/245(VOUTP_SPTGDet_flg) -> bus_creator/245
  outpmodule/252(VOUTP_FuelDoorPos_flg) -> bus_creator/252
  outpmodule/830(VOUTP_FDCTHCCLEVentZStaSet3_enum) -> bus_creator/830
  bus_selector9/12 -> outpmodule/620(VNMM_NetworkReq_flg)  "<VNMM_NetworkReq_flg>"
  outpmodule/113(VOUTP_YawRateV_flg) -> bus_creator/113
  bus_selector9/10 -> outpmodule/618(VNMM_ActiveWU_flg)  "<VNMM_ActiveWU_flg>"
  bus_selector12/108 -> outpmodule/819(VTHC_LEVentModeStaSet457_enum)  "<VTHC_LEVentModeStaSet457_enum>"
  bus_selector2/9 -> outpmodule/12(VAPM_PASDRCL_cm)  "<VAPM_PASDRCL_cm>"
  bus_selector2/85 -> outpmodule/88(VAPM_ShifterHandleCmdTimeOut_flg)  "<VAPM_ShifterHandleCmdTimeOut_flg>"
  bus_selector3/70 -> outpmodule/248(VBCM_IVIRST_flg)  "<VBCM_IVIRST_flg>"
  bus_selector9/11 -> outpmodule/619(VNMM_SysNMmSta_enum)  "<VNMM_SysNMmSta_enum>"
  outpmodule/887(VOUTP_THSysErrlampReq_flg) -> bus_creator/887
  outpmodule/302(VOUTP_FDLHandleLampCmd_flg) -> bus_creator/302
  bus_selector9/9 -> outpmodule/617(VNMM_WakeUp_enum)  "<VNMM_WakeUp_enum>"
  bus_selector3/119 -> outpmodule/297(VBCM_SPTGENFun_flg)  "<VBCM_SPTGENFun_flg>"
  bus_selector2/106 -> outpmodule/109(VAPM_LongAccel_Gps)  "<VAPM_LongAccel_Gps>"
  bus_selector4/25 -> outpmodule/382(VDDM_MCU4PreDTC_raw32)  "<VDDM_MCU4PreDTC_raw32>"
  bus_selector2/45 -> outpmodule/48(VAPM_LFRawWhlSpeedTimeOut_flg)  "<VAPM_LFRawWhlSpeedTimeOut_flg>"
  bus_selector9/8 -> outpmodule/616(VNMM_RptMsgReq_flg)  "<VNMM_RptMsgReq_flg>"
  outpmodule/666(VOUTP_OTAPwrReqOFFChkSta_enum) -> bus_creator/666
  bus_selector12/171 -> outpmodule/882(VTHC_CLVentEN_flg)  "<VTHC_CLVentEN_flg>"
  bus_selector9/6 -> outpmodule/614(VNMM_NodeID_enum)  "<VNMM_NodeID_enum>"
  outpmodule/810(VOUTP_FDCFGSChStaSet123_enum) -> bus_creator/810
  outpmodule/109(VOUTP_LongAccel_Gps) -> bus_creator/109
  outpmodule/471(VOUTP_RRBatwarnDTC_raw32) -> bus_creator/471
  bus_selector3/61 -> outpmodule/239(VBCM_AmbLightColor2_enum)  "<VBCM_AmbLightColor2_enum>"
  bus_selector12/80 -> outpmodule/791(VTHC_FaceMSet_enum)  "<VTHC_FaceMSet_enum>"
  BBCM_outputs/1 -> bus_selector3/1
  bus_selector9/7 -> outpmodule/615(VNMM_PNI_flg)  "<VNMM_PNI_flg>"
  bus_selector14/36 -> outpmodule/1020(VTQD_RrUdcMax_V)  "<VTQD_RrUdcMax_V>"
  outpmodule/34(VOUTP_USSStaRCL_flg) -> bus_creator/34
  outpmodule/414(VOUTP_ESC5NoComDTC_raw32) -> bus_creator/414
  bus_selector9/1 -> outpmodule/609(VNMM_AllCANTxReq_flg)  "<VNMM_AllCANTxReq_flg>"
  bus_selector4/90 -> outpmodule/447(VDDM_RrMCUSigErrDetDTC_raw32)  "<VDDM_RrMCUSigErrDetDTC_raw32>"
  BDSC_outputs/1 -> bus_selector8/1
  outpmodule/1073(VOUTP_RearWhlSlipRatioCtrl_flg) -> bus_creator/1073
  outpmodule/382(VOUTP_MCU4PreDTC_raw32) -> bus_creator/382
  bus_selector3/27 -> outpmodule/205(VBCM_ReverseLamp_flg)  "<VBCM_ReverseLamp_flg>"
  bus_selector2/25 -> outpmodule/28(VAPM_PASAFCR_enum)  "<VAPM_PASAFCR_enum>"
  bus_selector3/144 -> outpmodule/322(VBCM_PTGUserHeight4_cnt)  "<VBCM_PTGUserHeight4_cnt>"
  bus_selector7/9 -> outpmodule/563(VDKC_DkeyShowIVISta_enum)  "<VDKC_DkeyShowIVISta_enum>"
  bus_selector8/4 -> outpmodule/608(VDSC_DISCButtSta_flg)  "<VDSC_DISCButtSta_flg>"
  bus_selector8/2 -> outpmodule/606(VDSC_DISCTargetSpd_kph)  "<VDSC_DISCTargetSpd_kph>"
  outpmodule/202(VOUTP_HBeam_flg) -> bus_creator/202
  bus_selector4/24 -> outpmodule/381(VDDM_HVB4PreDTC_raw32)  "<VDDM_HVB4PreDTC_raw32>"
  bus_selector2/142 -> outpmodule/145(VAPM_IVIStatus_flg)  "<VAPM_IVIStatus_flg>"
  bus_selector4/6 -> outpmodule/363(VDDM_C3BMS1LCDTC_raw32)  "<VDDM_C3BMS1LCDTC_raw32>"
  bus_selector4/5 -> outpmodule/362(VDDM_C3BMS1CSDTC_raw32)  "<VDDM_C3BMS1CSDTC_raw32>"
  outpmodule/892(VOUTP_LFWheelPress_raw8) -> bus_creator/892
  outpmodule/814(VOUTP_LVentENSet_enum) -> bus_creator/814
  outpmodule/317(VOUTP_PTGOpenHeightSta_enum) -> bus_creator/317
  bus_creator/1 -> BOUTP_outputs/1
  bus_selector4/1 -> outpmodule/358(VDDM_C3BMS6RCDTC_raw32)  "<VDDM_C3BMS6RCDTC_raw32>"
  bus_selector4/138 -> outpmodule/495(VDDM_EDriveSysErrShifterErr_flg)  "<VDDM_EDriveSysErrShifterErr_flg>"
  bus_selector3/39 -> outpmodule/217(VBCM_RoomLampH_flg)  "<VBCM_RoomLampH_flg>"
  bus_selector4/4 -> outpmodule/361(VDDM_C3BMS1RCDTC_raw32)  "<VDDM_C3BMS1RCDTC_raw32>"
  outpmodule/754(VOUTP_Frost_flg) -> bus_creator/754
  bus_selector2/66 -> outpmodule/69(VAPM_RRWhlRotDir_enum)  "<VAPM_RRWhlRotDir_enum>"
  outpmodule/971(VOUTP_unlearnSfali_flg) -> bus_creator/971
  bus_selector4/7 -> outpmodule/364(VDDM_C3CCU1RCDTC_raw32)  "<VDDM_C3CCU1RCDTC_raw32>"
  outpmodule/936(VOUTP_S4L_enum) -> bus_creator/936
  bus_selector4/10 -> outpmodule/367(VDDM_C3CCU2RCDTC_raw32)  "<VDDM_C3CCU2RCDTC_raw32>"
  bus_selector12/96 -> outpmodule/807(VTHC_AirIntenZone3MSet5_enum)  "<VTHC_AirIntenZone3MSet5_enum>"
  outpmodule/281(VOUTP_AmbColorSta4_enum) -> bus_creator/281
  bus_selector2/174 -> outpmodule/177(VAPM_RAPSErrLv1_flg)  "<VAPM_RAPSErrLv1_flg>"
